simulink model "SecRwLtStCalib"  (R2024b)
settings: Solver=FixedStepDiscrete  StartTime=0.0  StopTime=10.0  FixedStep=0.01  RelTol=1e-3
model workspace (MAT data in the model file):
  KeSMSwAcsMd6SecRwLtStBkReclnUpwdDnwdPos1Max_Val : Simulink.Parameter (value not decoded)
  KeSMSwAcsMd6SecRwLtStBkReclnUpwdDnwdPos1Min_Val : Simulink.Parameter (value not decoded)
  KeSMSwAcsMd6SecRwLtStBkReclnUpwdDnwdPos1_Val : Simulink.Parameter (value not decoded)
  KeSMSwAcsMd6SecRwLtStBkReclnUpwdDnwdPosMax_Val : Simulink.Parameter (value not decoded)
  KeSMSwAcsMd6SecRwLtStBkReclnUpwdDnwdPosMin_Val : Simulink.Parameter (value not decoded)
  KeSMSwAcsMd6SecRwLtStBkReclnUpwdDnwdPos_Val : Simulink.Parameter (value not decoded)
symbols that are objects in the model workspace (value not decoded): KeSMSwAcsMd6SecRwLtStBkReclnUpwdDnwdPos1_Val, KeSMSwAcsMd6SecRwLtStBkReclnUpwdDnwdPos1Max_Val, KeSMSwAcsMd6SecRwLtStBkReclnUpwdDnwdPos1Min_Val, KeSMSwAcsMd6SecRwLtStBkReclnUpwdDnwdPos_Val, KeSMSwAcsMd6SecRwLtStBkReclnUpwdDnwdPosMax_Val, KeSMSwAcsMd6SecRwLtStBkReclnUpwdDnwdPosMin_Val
undefined symbols (not defined in the file or in its folder): KeSMSw4SAcsMd21SecRwLtStBkReclnUpwdDnwdPos_Val, KeSMSw4SAcsMd21SecRwLtStBkReclnUpwdDnwdPosMax_Val, KeSMSw4SAcsMd21SecRwLtStBkReclnUpwdDnwdPosMin_Val, KeSMSw4SAcsMd21SecRwLtStFrwdBkwdPos_Val, KeSMSw4SAcsMd21SecRwLtStFrwdBkwdPosMax_Val, KeSMSw4SAcsMd21SecRwLtStFrwdBkwdPosMin_Val, KeSMSw4SAcsMd21SecRwLtStHdrstFrwdBkwdPos_Val, KeSMSw4SAcsMd21SecRwLtStHdrstFrwdBkwdPosMax_Val, KeSMSw4SAcsMd21SecRwLtStHdrstFrwdBkwdPosMin_Val, KeSMSw4SAcsMd21SecRwLtStHdrstUpwdDnwdPos_Val, KeSMSw4SAcsMd21SecRwLtStHdrstUpwdDnwdPosMax_Val, KeSMSw4SAcsMd21SecRwLtStHdrstUpwdDnwdPosMin_Val, KeSMSw4SAcsMd22SecRwLtStBkReclnUpwdDnwdPos1_Val, KeSMSw4SAcsMd22SecRwLtStBkReclnUpwdDnwdPos2_Val, KeSMSw4SAcsMd22SecRwLtStBkReclnUpwdDnwdPos2Max_Val, KeSMSw4SAcsMd22SecRwLtStBkReclnUpwdDnwdPos2Min_Val, KeSMSw4SAcsMd22SecRwLtStBkReclnUpwdDnwdPosMax_Val, KeSMSw4SAcsMd22SecRwLtStBkReclnUpwdDnwdPosMin_Val, KeSMSw4SAcsMd22SecRwLtStFrwdBkwdPos_Val, KeSMSw4SAcsMd22SecRwLtStFrwdBkwdPosMax_Val, KeSMSw4SAcsMd22SecRwLtStFrwdBkwdPosMin_Val, KeSMSw4SAcsMd22SecRwLtStFtrstUpwdDnwdPos_Val, KeSMSw4SAcsMd22SecRwLtStFtrstUpwdDnwdPosMax_Val, KeSMSw4SAcsMd22SecRwLtStFtrstUpwdDnwdPosMin_Val, KeSMSw4SAcsMd22SecRwLtStHdrstFrwdBkwdPos_Val, KeSMSw4SAcsMd22SecRwLtStHdrstFrwdBkwdPosMax_Val, KeSMSw4SAcsMd22SecRwLtStHdrstFrwdBkwdPosMin_Val, KeSMSw4SAcsMd22SecRwLtStHdrstUpwdDnwdPos_Val, KeSMSw4SAcsMd22SecRwLtStHdrstUpwdDnwdPosMax_Val, KeSMSw4SAcsMd22SecRwLtStHdrstUpwdDnwdPosMin_Val, KeSMSw4SAcsMd22SecRwLtStLegrstOtwdInwdPos_Val, KeSMSw4SAcsMd22SecRwLtStLegrstOtwdInwdPosMax_Val, KeSMSw4SAcsMd22SecRwLtStLegrstOtwdInwdPosMin_Val, KeSMSw4SAcsMd22SecRwLtStLegrstUpwdDnwdPos_Val, KeSMSw4SAcsMd22SecRwLtStLegrstUpwdDnwdPosMax_Val, KeSMSw4SAcsMd22SecRwLtStLegrstUpwdDnwdPosMin_Val, KeSMSw4SAcsMd25SecRwLtStBkReclnUpwdDnwdPos_Val, KeSMSw4SAcsMd25SecRwLtStBkReclnUpwdDnwdPosMax_Val, KeSMSw4SAcsMd25SecRwLtStBkReclnUpwdDnwdPosMin_Val, KeSMSw4SAcsMd25SecRwLtStFrwdBkwdPos_Val, KeSMSw4SAcsMd25SecRwLtStFrwdBkwdPosMax_Val, KeSMSw4SAcsMd25SecRwLtStFrwdBkwdPosMin_Val, KeSMSw4SAcsMd25SecRwLtStHdrstFrwdBkwdPos_Val, KeSMSw4SAcsMd25SecRwLtStHdrstFrwdBkwdPosMax_Val, KeSMSw4SAcsMd25SecRwLtStHdrstFrwdBkwdPosMin_Val, KeSMSw4SAcsMd25SecRwLtStHdrstUpwdDnwdPos_Val, KeSMSw4SAcsMd25SecRwLtStHdrstUpwdDnwdPosMax_Val, KeSMSw4SAcsMd25SecRwLtStHdrstUpwdDnwdPosMin_Val, KeSMSw4SAcsMd26SecRwLtStBkReclnUpwdDnwdPos_Val, KeSMSw4SAcsMd26SecRwLtStBkReclnUpwdDnwdPosMax_Val, KeSMSw4SAcsMd26SecRwLtStBkReclnUpwdDnwdPosMin_Val, KeSMSw4SAcsMd26SecRwLtStFrwdBkwdPos_Val, KeSMSw4SAcsMd26SecRwLtStFrwdBkwdPosMax_Val, KeSMSw4SAcsMd26SecRwLtStFrwdBkwdPosMin_Val, KeSMSw4SAcsMd26SecRwLtStFtrstUpwdDnwdPos_Val, KeSMSw4SAcsMd26SecRwLtStFtrstUpwdDnwdPosMax_Val, KeSMSw4SAcsMd26SecRwLtStFtrstUpwdDnwdPosMin_Val, KeSMSw4SAcsMd26SecRwLtStHdrstFrwdBkwdPos_Val, KeSMSw4SAcsMd26SecRwLtStHdrstFrwdBkwdPosMax_Val, KeSMSw4SAcsMd26SecRwLtStHdrstFrwdBkwdPosMin_Val ... (+496)
libraries: TrgtPosSelcLib x61, StIsPosChkLib x1, simulink x1
(part 4 of 8)

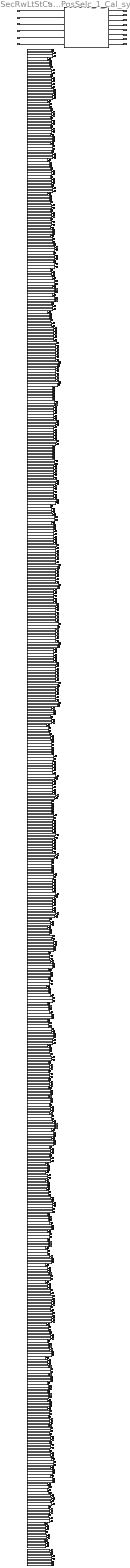
== system SecRwLtStCalib/SecRwLtStZeroTrgtPosSelc_1_Cal_sys ==
  note: Added blocks
  note: Added blocks
  note: Added blocks
  note: Added blocks
  note: Added blocks
  note: Added blocks
  note: Added blocks
  note: Added blocks
  note: Added blocks
  note: Added blocks
  note: Added blocks
  note: Added blocks
  note: Added blocks
  note: Added blocks
  note: Added blocks
  note: Added blocks
  note: Added blocks
  note: Added blocks
  note: Added blocks
  note: Added blocks
  note: Added blocks
  note: Added blocks
  note: Added blocks
  note: Added blocks
  note: Added blocks
  note: Added blocks
  note: Added blocks
  note: Added blocks
  note: Added blocks
  note: Added blocks
  note: Added blocks
  note: Added blocks
  note: Added blocks
  note: Added blocks
  note: Added blocks
  note: Added blocks
  note: Added blocks
  note: Added blocks
  note: Added blocks
  note: Added blocks
  note: Added blocks
  note: Added blocks
  note: Added blocks
  note: Added blocks
  note: Added blocks
  note: Added blocks
  note: Added blocks
  note: Added blocks
  note: Added blocks
  note: Added blocks
  note: Added blocks
  note: Added blocks
  note: Added blocks
  note: Added blocks
  note: Added blocks
  note: Added blocks
  note: Added blocks
  note: Added blocks
  note: Added blocks
  note: Added blocks
  note: Added blocks
  note: Added blocks
  note: Added blocks
  note: Added blocks
  note: Added blocks
  note: Added blocks
  note: Added blocks
  note: Added blocks
  note: Added blocks
  note: Added blocks
  note: Added blocks
  note: Added blocks
  note: Added blocks
  note: Added blocks
  note: Added blocks
  note: Added blocks
  note: Added blocks
  note: Added blocks
  note: Added blocks
  note: Added blocks
  note: Added blocks
  note: Added blocks
  note: Added blocks
  note: Added blocks
  note: Added blocks
  note: Added blocks
  note: Added blocks
  note: Added blocks
  note: Added blocks
  note: Added blocks
  note: Added blocks
  note: Added blocks
  note: Added blocks
  note: Added blocks
  note: Added blocks
  note: Added blocks
  note: Added blocks
  note: Added blocks
  note: Added blocks
  note: Added blocks
  note: Added blocks
  note: Added blocks
  note: Added blocks
  note: Added blocks
  note: Added blocks
  note: Added blocks
  note: Added blocks
  note: Added blocks
  note: Added blocks
  note: Added blocks
  note: Added blocks
  note: Added blocks
  note: Added blocks
  note: Added blocks
  note: Added blocks
  note: Added blocks
  note: Added blocks
  note: Added blocks
  note: Added blocks
  note: Added blocks
  note: Added blocks
  note: Added blocks
  note: Added blocks
  note: Added blocks
  note: Added blocks
  note: Added blocks
  note: Added blocks
  note: Added blocks
  note: Added blocks
  note: Added blocks
  note: Added blocks
  note: Added blocks
  note: Added blocks
  note: Added blocks
  note: Added blocks
  note: Added blocks
  note: Added blocks
  note: Added blocks
  note: Added blocks
  note: Added blocks
  note: Added blocks
  note: Added blocks
  note: Added blocks
  note: Added blocks
  note: Added blocks
  note: Added blocks
  note: Added blocks
  note: Added blocks
  note: Added blocks
  note: Added blocks
  note: Added blocks
  note: Added blocks
  note: Added blocks
  note: Added blocks
  note: Added blocks
  note: Added blocks
  note: Added blocks
  note: Added blocks
  note: Added blocks
  note: Added blocks
  note: Added blocks
  note: Added blocks
  note: Added blocks
  note: Added blocks
  note: Added blocks
  note: Added blocks
  note: Added blocks
  note: Added blocks
  note: Added blocks
  note: Added blocks
  note: Added blocks
  note: Added blocks
  note: Added blocks
  note: Added blocks
  note: Added blocks
  note: Added blocks
  note: Added blocks
  note: Added blocks
  note: Added blocks
  note: Added blocks
  note: Added blocks
  note: Added blocks
  note: Added blocks
  note: Added blocks
  note: Added blocks
  note: Added blocks
  note: Added blocks
  note: Added blocks
  note: Added blocks
  note: Added blocks
  note: Added blocks
  note: Added blocks
  note: Added blocks
  note: Added blocks
  note: Added blocks
  note: Added blocks
  note: Added blocks
  note: Added blocks
  note: Added blocks
  note: Added blocks
  note: Added blocks
  note: Added blocks
  note: Added blocks
  note: Added blocks
  note: Added blocks
  note: Added blocks
  note: Added blocks
  note: Added blocks
  note: Added blocks
  note: Added blocks
  note: Added blocks
  note: Added blocks
  note: Added blocks
  note: Added blocks
  note: Added blocks
  note: Added blocks
  note: Added blocks
  note: Added blocks
  note: Added blocks
  note: Added blocks
  note: Added blocks
  note: Added blocks
  note: Added blocks
  note: Added blocks
  note: Added blocks
  note: Added blocks
  note: Added blocks
  note: Added blocks
  note: Added blocks
  note: Added blocks
  note: Added blocks
  note: Added blocks
  note: Added blocks
  note: Added blocks
  note: Added blocks
  note: Added blocks
  note: Added blocks
  note: Added blocks
  note: Added blocks
  note: Added blocks
  note: Added blocks
  note: Added blocks
  note: Added blocks
  note: Added blocks
  note: Added blocks
  note: Added blocks
  note: Added blocks
  note: Added blocks
  note: Added blocks
  note: Added blocks
  note: Added blocks
  note: Added blocks
  note: Added blocks
  note: Added blocks
  note: Added blocks
  note: Added blocks
  note: Added blocks
  note: Added blocks
  note: Added blocks
  note: Added blocks
  note: Added blocks
  note: Added blocks
  note: Added blocks
  note: Added blocks
  note: Added blocks
  note: Added blocks
  note: Added blocks
  note: Added blocks
  note: Added blocks
  note: Added blocks
  note: Added blocks
  note: Added blocks
  note: Added blocks
  note: Added blocks
  note: Added blocks
  note: Added blocks
  note: Added blocks
  note: Added blocks
  note: Added blocks
  note: Added blocks
  note: Added blocks
  note: Added blocks
  note: Added blocks
  note: Added blocks
  note: Added blocks
  note: Added blocks
  note: Added blocks
  note: Added blocks
  note: Added blocks
  note: Added blocks
  note: Added blocks
  note: Added blocks
  note: Added blocks
  note: Added blocks
  note: Added blocks
  note: Added blocks
  note: Added blocks
  note: Added blocks
  note: Added blocks
  note: Added blocks
  note: Added blocks
  note: Added blocks
  note: Added blocks
  note: Added blocks
  note: Added blocks
  note: Added blocks
  note: Added blocks
  note: Added blocks
  note: Added blocks
  note: Added blocks
  note: Added blocks
  note: Added blocks
  note: Added blocks
  note: Added blocks
  note: Added blocks
  note: Added blocks
  note: Added blocks
  note: Added blocks
  note: Added blocks
  note: Added blocks
  note: Added blocks
  note: Added blocks
  note: Added blocks
  note: Added blocks
  note: Added blocks
  note: Added blocks
  note: Added blocks
  note: Added blocks
  note: Added blocks
  note: Added blocks
  note: Added blocks
  note: Added blocks
  note: Added blocks
  note: Added blocks
  note: Added blocks
  note: Added blocks
  note: Added blocks
  note: Added blocks
  note: Added blocks
  note: Added blocks
  note: Added blocks
  note: Added blocks
  note: Added blocks
  note: Added blocks
  note: Added blocks
  note: Added blocks
  note: Added blocks
  note: Added blocks
  note: Added blocks
  note: Added blocks
  note: Added blocks
  note: Added blocks
  note: Added blocks
  note: Added blocks
  note: Added blocks
  note: Added blocks
  note: Added blocks
  note: Added blocks
  note: Added blocks
  note: Added blocks
  note: Added blocks
  note: Added blocks
  note: Added blocks
  note: Added blocks
  note: Added blocks
  note: Added blocks
  note: Added blocks
  note: Added blocks
  note: Added blocks
  note: Added blocks
  note: Added blocks
  note: Added blocks
  note: Added blocks
  note: Added blocks
  note: Added blocks
  note: Added blocks
  note: Added blocks
  note: Added blocks
  note: Added blocks
  note: Added blocks
  note: Added blocks
  note: Added blocks
  note: Added blocks
  note: Added blocks
  note: Added blocks
  note: Added blocks
  note: Added blocks
  note: Added blocks
  note: Added blocks
  note: Added blocks
  note: Added blocks
  note: Added blocks
  note: Added blocks
  note: Added blocks
  note: Added blocks
  note: Added blocks
  note: Added blocks
  note: Added blocks
  note: Added blocks
  note: Added blocks
  note: Added blocks
  note: Added blocks
  note: Added blocks
  note: Added blocks
  note: Added blocks
  note: Added blocks
  note: Added blocks
  note: Added blocks
  note: Added blocks
  note: Added blocks
  note: Added blocks
  note: Added blocks
  note: Added blocks
  note: Added blocks
  note: Added blocks
  note: Added blocks
  note: Added blocks
  note: Added blocks
  note: Added blocks
  note: Added blocks
  note: Added blocks
  note: Added blocks
  note: Added blocks
  note: Added blocks
  note: Added blocks
  note: Added blocks
  note: Added blocks
  note: Added blocks
  note: Added blocks
  note: Added blocks
  note: Added blocks
  note: Added blocks
  note: Added blocks
  note: Added blocks
  note: Added blocks
  note: Added blocks
  note: Added blocks
  note: Added blocks
  note: Added blocks
  note: Added blocks
  note: Added blocks
  note: Added blocks
  note: Added blocks
  note: Added blocks
  note: Added blocks
  note: Added blocks
  note: Added blocks
  note: Added blocks
  note: Added blocks
  note: Added blocks
  note: Added blocks
  note: Added blocks
  note: Added blocks
  note: Added blocks
  note: Added blocks
  note: Added blocks
  note: Added blocks
  note: Added blocks
  note: Added blocks
  note: Added blocks
  note: Added blocks
  note: Added blocks
  note: Added blocks
  note: Added blocks
  note: Added blocks
  note: Added blocks
  note: Added blocks
  note: Added blocks
  note: Added blocks
  note: Added blocks
  note: Added blocks
  note: Added blocks
  note: Added blocks
  note: Added blocks
  note: Added blocks
  note: Added blocks
  note: Added blocks
  note: Added blocks
  note: Added blocks
  note: Added blocks
  note: Added blocks
  note: Added blocks
  note: Added blocks
  note: Added blocks
  note: Added blocks
  note: Added blocks
  note: Added blocks
  note: Added blocks
  note: Added blocks
  note: Added blocks
  note: Added blocks
  note: Added blocks
  note: Added blocks
  note: Added blocks
  note: Added blocks
  note: Added blocks
  note: Added blocks
  note: Added blocks
  note: Added blocks
  note: Added blocks
  note: Added blocks
  note: Added blocks
  note: Added blocks
  note: Added blocks
  note: Added blocks
  note: Added blocks
  note: Added blocks
  note: Added blocks
  note: Added blocks
  note: Added blocks
  note: Added blocks
  note: Added blocks
  note: Added blocks
  note: Added blocks
  note: Added blocks
  note: Added blocks
  note: Added blocks
  note: Added blocks
  note: Added blocks
  note: Added blocks
  note: Added blocks
  note: Added blocks
  note: Added blocks
  note: Added blocks
  note: Added blocks
  note: Added blocks
  note: Added blocks
  note: Added blocks
  note: Added blocks
  note: Added blocks
  note: Added blocks
  note: Added blocks
  note: Added blocks
  note: Added blocks
  note: Added blocks
  note: Added blocks
  note: Added blocks
  note: Added blocks
  note: Added blocks
  StNumFlg_Is4s_read : Inport
  StNumFlg_Is6s_read : Inport  Port=2
  StNumFlg_Is6s7s_read : Inport  Port=3
  StNumFlg_Is7s_read : Inport  Port=4
  Md61SecRwRtStCushFrntTrgtPosCalib_TrgtPosArray_read : Inport  Port=5
  Md62SecRwLtStCushFrntTrgtPosCalib_TrgtPosArray_read : Inport  Port=6
  function : TriggerPort  TriggerType=function-call  IsSimulinkFunction=on  FunctionName=SecRwLtStZeroTrgtPosSelc_1_Cal  VariantControl=(inherit)
  PA_KeSMSw4SAcsMd21SecRwLtStBkReclnUpwdDnwdPosMax_Val : Constant  Value=KeSMSw4SAcsMd21SecRwLtStBkReclnUpwdDnwdPosMax_Val
  PA_KeSMSw4SAcsMd21SecRwLtStBkReclnUpwdDnwdPosMin_Val : Constant  Value=KeSMSw4SAcsMd21SecRwLtStBkReclnUpwdDnwdPosMin_Val
  PA_KeSMSw4SAcsMd21SecRwLtStBkReclnUpwdDnwdPos_Val : Constant  Value=KeSMSw4SAcsMd21SecRwLtStBkReclnUpwdDnwdPos_Val
  PA_KeSMSw4SAcsMd21SecRwLtStFrwdBkwdPosMax_Val : Constant  Value=KeSMSw4SAcsMd21SecRwLtStFrwdBkwdPosMax_Val
  PA_KeSMSw4SAcsMd21SecRwLtStFrwdBkwdPosMin_Val : Constant  Value=KeSMSw4SAcsMd21SecRwLtStFrwdBkwdPosMin_Val
  PA_KeSMSw4SAcsMd21SecRwLtStFrwdBkwdPos_Val : Constant  Value=KeSMSw4SAcsMd21SecRwLtStFrwdBkwdPos_Val
  PA_KeSMSw4SAcsMd21SecRwLtStHdrstFrwdBkwdPosMax_Val : Constant  Value=KeSMSw4SAcsMd21SecRwLtStHdrstFrwdBkwdPosMax_Val
  PA_KeSMSw4SAcsMd21SecRwLtStHdrstFrwdBkwdPosMin_Val : Constant  Value=KeSMSw4SAcsMd21SecRwLtStHdrstFrwdBkwdPosMin_Val
  PA_KeSMSw4SAcsMd21SecRwLtStHdrstFrwdBkwdPos_Val : Constant  Value=KeSMSw4SAcsMd21SecRwLtStHdrstFrwdBkwdPos_Val
  PA_KeSMSw4SAcsMd21SecRwLtStHdrstUpwdDnwdPosMax_Val : Constant  Value=KeSMSw4SAcsMd21SecRwLtStHdrstUpwdDnwdPosMax_Val
  PA_KeSMSw4SAcsMd21SecRwLtStHdrstUpwdDnwdPosMin_Val : Constant  Value=KeSMSw4SAcsMd21SecRwLtStHdrstUpwdDnwdPosMin_Val
  PA_KeSMSw4SAcsMd21SecRwLtStHdrstUpwdDnwdPos_Val : Constant  Value=KeSMSw4SAcsMd21SecRwLtStHdrstUpwdDnwdPos_Val
  PA_KeSMSw4SAcsMd22SecRwLtStBkReclnUpwdDnwdPos1_Val : Constant  Value=KeSMSw4SAcsMd22SecRwLtStBkReclnUpwdDnwdPos1_Val
  PA_KeSMSw4SAcsMd22SecRwLtStBkReclnUpwdDnwdPos2Max_Val : Constant  Value=KeSMSw4SAcsMd22SecRwLtStBkReclnUpwdDnwdPos2Max_Val
  PA_KeSMSw4SAcsMd22SecRwLtStBkReclnUpwdDnwdPos2Min_Val : Constant  Value=KeSMSw4SAcsMd22SecRwLtStBkReclnUpwdDnwdPos2Min_Val
  PA_KeSMSw4SAcsMd22SecRwLtStBkReclnUpwdDnwdPos2_Val : Constant  Value=KeSMSw4SAcsMd22SecRwLtStBkReclnUpwdDnwdPos2_Val
  PA_KeSMSw4SAcsMd22SecRwLtStBkReclnUpwdDnwdPosMax_Val : Constant  Value=KeSMSw4SAcsMd22SecRwLtStBkReclnUpwdDnwdPosMax_Val
  PA_KeSMSw4SAcsMd22SecRwLtStBkReclnUpwdDnwdPosMin_Val : Constant  Value=KeSMSw4SAcsMd22SecRwLtStBkReclnUpwdDnwdPosMin_Val
  PA_KeSMSw4SAcsMd22SecRwLtStFrwdBkwdPosMax_Val : Constant  Value=KeSMSw4SAcsMd22SecRwLtStFrwdBkwdPosMax_Val
  PA_KeSMSw4SAcsMd22SecRwLtStFrwdBkwdPosMin_Val : Constant  Value=KeSMSw4SAcsMd22SecRwLtStFrwdBkwdPosMin_Val
  PA_KeSMSw4SAcsMd22SecRwLtStFrwdBkwdPos_Val : Constant  Value=KeSMSw4SAcsMd22SecRwLtStFrwdBkwdPos_Val
  PA_KeSMSw4SAcsMd22SecRwLtStFtrstUpwdDnwdPosMax_Val : Constant  Value=KeSMSw4SAcsMd22SecRwLtStFtrstUpwdDnwdPosMax_Val
  PA_KeSMSw4SAcsMd22SecRwLtStFtrstUpwdDnwdPosMin_Val : Constant  Value=KeSMSw4SAcsMd22SecRwLtStFtrstUpwdDnwdPosMin_Val
  PA_KeSMSw4SAcsMd22SecRwLtStFtrstUpwdDnwdPos_Val : Constant  Value=KeSMSw4SAcsMd22SecRwLtStFtrstUpwdDnwdPos_Val
  PA_KeSMSw4SAcsMd22SecRwLtStHdrstFrwdBkwdPosMax_Val : Constant  Value=KeSMSw4SAcsMd22SecRwLtStHdrstFrwdBkwdPosMax_Val
  PA_KeSMSw4SAcsMd22SecRwLtStHdrstFrwdBkwdPosMin_Val : Constant  Value=KeSMSw4SAcsMd22SecRwLtStHdrstFrwdBkwdPosMin_Val
  PA_KeSMSw4SAcsMd22SecRwLtStHdrstFrwdBkwdPos_Val : Constant  Value=KeSMSw4SAcsMd22SecRwLtStHdrstFrwdBkwdPos_Val
  PA_KeSMSw4SAcsMd22SecRwLtStHdrstUpwdDnwdPosMax_Val : Constant  Value=KeSMSw4SAcsMd22SecRwLtStHdrstUpwdDnwdPosMax_Val
  PA_KeSMSw4SAcsMd22SecRwLtStHdrstUpwdDnwdPosMin_Val : Constant  Value=KeSMSw4SAcsMd22SecRwLtStHdrstUpwdDnwdPosMin_Val
  PA_KeSMSw4SAcsMd22SecRwLtStHdrstUpwdDnwdPos_Val : Constant  Value=KeSMSw4SAcsMd22SecRwLtStHdrstUpwdDnwdPos_Val
  PA_KeSMSw4SAcsMd22SecRwLtStLegrstOtwdInwdPosMax_Val : Constant  Value=KeSMSw4SAcsMd22SecRwLtStLegrstOtwdInwdPosMax_Val
  PA_KeSMSw4SAcsMd22SecRwLtStLegrstOtwdInwdPosMin_Val : Constant  Value=KeSMSw4SAcsMd22SecRwLtStLegrstOtwdInwdPosMin_Val
  PA_KeSMSw4SAcsMd22SecRwLtStLegrstOtwdInwdPos_Val : Constant  Value=KeSMSw4SAcsMd22SecRwLtStLegrstOtwdInwdPos_Val
  PA_KeSMSw4SAcsMd22SecRwLtStLegrstUpwdDnwdPosMax_Val : Constant  Value=KeSMSw4SAcsMd22SecRwLtStLegrstUpwdDnwdPosMax_Val
  PA_KeSMSw4SAcsMd22SecRwLtStLegrstUpwdDnwdPosMin_Val : Constant  Value=KeSMSw4SAcsMd22SecRwLtStLegrstUpwdDnwdPosMin_Val
  PA_KeSMSw4SAcsMd22SecRwLtStLegrstUpwdDnwdPos_Val : Constant  Value=KeSMSw4SAcsMd22SecRwLtStLegrstUpwdDnwdPos_Val
  PA_KeSMSw4SAcsMd25SecRwLtStBkReclnUpwdDnwdPosMax_Val : Constant  Value=KeSMSw4SAcsMd25SecRwLtStBkReclnUpwdDnwdPosMax_Val
  PA_KeSMSw4SAcsMd25SecRwLtStBkReclnUpwdDnwdPosMin_Val : Constant  Value=KeSMSw4SAcsMd25SecRwLtStBkReclnUpwdDnwdPosMin_Val
  PA_KeSMSw4SAcsMd25SecRwLtStBkReclnUpwdDnwdPos_Val : Constant  Value=KeSMSw4SAcsMd25SecRwLtStBkReclnUpwdDnwdPos_Val
  PA_KeSMSw4SAcsMd25SecRwLtStFrwdBkwdPosMax_Val : Constant  Value=KeSMSw4SAcsMd25SecRwLtStFrwdBkwdPosMax_Val
  PA_KeSMSw4SAcsMd25SecRwLtStFrwdBkwdPosMin_Val : Constant  Value=KeSMSw4SAcsMd25SecRwLtStFrwdBkwdPosMin_Val
  PA_KeSMSw4SAcsMd25SecRwLtStFrwdBkwdPos_Val : Constant  Value=KeSMSw4SAcsMd25SecRwLtStFrwdBkwdPos_Val
  PA_KeSMSw4SAcsMd25SecRwLtStHdrstFrwdBkwdPosMax_Val : Constant  Value=KeSMSw4SAcsMd25SecRwLtStHdrstFrwdBkwdPosMax_Val
  PA_KeSMSw4SAcsMd25SecRwLtStHdrstFrwdBkwdPosMin_Val : Constant  Value=KeSMSw4SAcsMd25SecRwLtStHdrstFrwdBkwdPosMin_Val
  PA_KeSMSw4SAcsMd25SecRwLtStHdrstFrwdBkwdPos_Val : Constant  Value=KeSMSw4SAcsMd25SecRwLtStHdrstFrwdBkwdPos_Val
  PA_KeSMSw4SAcsMd25SecRwLtStHdrstUpwdDnwdPosMax_Val : Constant  Value=KeSMSw4SAcsMd25SecRwLtStHdrstUpwdDnwdPosMax_Val
  PA_KeSMSw4SAcsMd25SecRwLtStHdrstUpwdDnwdPosMin_Val : Constant  Value=KeSMSw4SAcsMd25SecRwLtStHdrstUpwdDnwdPosMin_Val
  PA_KeSMSw4SAcsMd25SecRwLtStHdrstUpwdDnwdPos_Val : Constant  Value=KeSMSw4SAcsMd25SecRwLtStHdrstUpwdDnwdPos_Val
  PA_KeSMSw4SAcsMd26SecRwLtStBkReclnUpwdDnwdPosMax_Val : Constant  Value=KeSMSw4SAcsMd26SecRwLtStBkReclnUpwdDnwdPosMax_Val
  PA_KeSMSw4SAcsMd26SecRwLtStBkReclnUpwdDnwdPosMin_Val : Constant  Value=KeSMSw4SAcsMd26SecRwLtStBkReclnUpwdDnwdPosMin_Val
  PA_KeSMSw4SAcsMd26SecRwLtStBkReclnUpwdDnwdPos_Val : Constant  Value=KeSMSw4SAcsMd26SecRwLtStBkReclnUpwdDnwdPos_Val
  PA_KeSMSw4SAcsMd26SecRwLtStFrwdBkwdPosMax_Val : Constant  Value=KeSMSw4SAcsMd26SecRwLtStFrwdBkwdPosMax_Val
  PA_KeSMSw4SAcsMd26SecRwLtStFrwdBkwdPosMin_Val : Constant  Value=KeSMSw4SAcsMd26SecRwLtStFrwdBkwdPosMin_Val
  PA_KeSMSw4SAcsMd26SecRwLtStFrwdBkwdPos_Val : Constant  Value=KeSMSw4SAcsMd26SecRwLtStFrwdBkwdPos_Val
  PA_KeSMSw4SAcsMd26SecRwLtStFtrstUpwdDnwdPosMax_Val : Constant  Value=KeSMSw4SAcsMd26SecRwLtStFtrstUpwdDnwdPosMax_Val
  PA_KeSMSw4SAcsMd26SecRwLtStFtrstUpwdDnwdPosMin_Val : Constant  Value=KeSMSw4SAcsMd26SecRwLtStFtrstUpwdDnwdPosMin_Val
  PA_KeSMSw4SAcsMd26SecRwLtStFtrstUpwdDnwdPos_Val : Constant  Value=KeSMSw4SAcsMd26SecRwLtStFtrstUpwdDnwdPos_Val
  PA_KeSMSw4SAcsMd26SecRwLtStHdrstFrwdBkwdPosMax_Val : Constant  Value=KeSMSw4SAcsMd26SecRwLtStHdrstFrwdBkwdPosMax_Val
  PA_KeSMSw4SAcsMd26SecRwLtStHdrstFrwdBkwdPosMin_Val : Constant  Value=KeSMSw4SAcsMd26SecRwLtStHdrstFrwdBkwdPosMin_Val
  PA_KeSMSw4SAcsMd26SecRwLtStHdrstFrwdBkwdPos_Val : Constant  Value=KeSMSw4SAcsMd26SecRwLtStHdrstFrwdBkwdPos_Val
  PA_KeSMSw4SAcsMd26SecRwLtStHdrstUpwdDnwdPosMax_Val : Constant  Value=KeSMSw4SAcsMd26SecRwLtStHdrstUpwdDnwdPosMax_Val
  PA_KeSMSw4SAcsMd26SecRwLtStHdrstUpwdDnwdPosMin_Val : Constant  Value=KeSMSw4SAcsMd26SecRwLtStHdrstUpwdDnwdPosMin_Val
  PA_KeSMSw4SAcsMd26SecRwLtStHdrstUpwdDnwdPos_Val : Constant  Value=KeSMSw4SAcsMd26SecRwLtStHdrstUpwdDnwdPos_Val
  PA_KeSMSw4SAcsMd26SecRwLtStLegrstOtwdInwdPosMax_Val : Constant  Value=KeSMSw4SAcsMd26SecRwLtStLegrstOtwdInwdPosMax_Val
  PA_KeSMSw4SAcsMd26SecRwLtStLegrstOtwdInwdPosMin_Val : Constant  Value=KeSMSw4SAcsMd26SecRwLtStLegrstOtwdInwdPosMin_Val
  PA_KeSMSw4SAcsMd26SecRwLtStLegrstOtwdInwdPos_Val : Constant  Value=KeSMSw4SAcsMd26SecRwLtStLegrstOtwdInwdPos_Val
  PA_KeSMSw4SAcsMd26SecRwLtStLegrstUpwdDnwdPosMax_Val : Constant  Value=KeSMSw4SAcsMd26SecRwLtStLegrstUpwdDnwdPosMax_Val
  PA_KeSMSw4SAcsMd26SecRwLtStLegrstUpwdDnwdPosMin_Val : Constant  Value=KeSMSw4SAcsMd26SecRwLtStLegrstUpwdDnwdPosMin_Val
  PA_KeSMSw4SAcsMd26SecRwLtStLegrstUpwdDnwdPos_Val : Constant  Value=KeSMSw4SAcsMd26SecRwLtStLegrstUpwdDnwdPos_Val
  PA_KeSMSw4SLegrstCloseMdSecRwLtStFtrstUpwdDnwdPosMax_Val : Constant  Value=KeSMSw4SLegrstCloseMdSecRwLtStFtrstUpwdDnwdPosMax_Val
  PA_KeSMSw4SLegrstCloseMdSecRwLtStFtrstUpwdDnwdPosMin_Val : Constant  Value=KeSMSw4SLegrstCloseMdSecRwLtStFtrstUpwdDnwdPosMin_Val
  PA_KeSMSw4SLegrstCloseMdSecRwLtStFtrstUpwdDnwdPos_Val : Constant  Value=KeSMSw4SLegrstCloseMdSecRwLtStFtrstUpwdDnwdPos_Val
  PA_KeSMSw4SLegrstCloseMdSecRwLtStLgrstOtwdInwdPosMax_Val : Constant  Value=KeSMSw4SLegrstCloseMdSecRwLtStLgrstOtwdInwdPosMax_Val
  PA_KeSMSw4SLegrstCloseMdSecRwLtStLgrstOtwdInwdPosMin_Val : Constant  Value=KeSMSw4SLegrstCloseMdSecRwLtStLgrstOtwdInwdPosMin_Val
  PA_KeSMSw4SLegrstCloseMdSecRwLtStLgrstOtwdInwdPos_Val : Constant  Value=KeSMSw4SLegrstCloseMdSecRwLtStLgrstOtwdInwdPos_Val
  PA_KeSMSw4SLegrstCloseMdSecRwLtStLgrstUpwdDnwdPosMax_Val : Constant  Value=KeSMSw4SLegrstCloseMdSecRwLtStLgrstUpwdDnwdPosMax_Val
  PA_KeSMSw4SLegrstCloseMdSecRwLtStLgrstUpwdDnwdPosMin_Val : Constant  Value=KeSMSw4SLegrstCloseMdSecRwLtStLgrstUpwdDnwdPosMin_Val
  PA_KeSMSw4SLegrstCloseMdSecRwLtStLgrstUpwdDnwdPos_Val : Constant  Value=KeSMSw4SLegrstCloseMdSecRwLtStLgrstUpwdDnwdPos_Val
  PA_KeSMSw4SLegrstOpenMdSecRwLtStFrwdBkwdPosMax_Val : Constant  Value=KeSMSw4SLegrstOpenMdSecRwLtStFrwdBkwdPosMax_Val
  PA_KeSMSw4SLegrstOpenMdSecRwLtStFrwdBkwdPosMin_Val : Constant  Value=KeSMSw4SLegrstOpenMdSecRwLtStFrwdBkwdPosMin_Val
  PA_KeSMSw4SLegrstOpenMdSecRwLtStFrwdBkwdPos_Val : Constant  Value=KeSMSw4SLegrstOpenMdSecRwLtStFrwdBkwdPos_Val
  PA_KeSMSw4SLegrstOpenMdSecRwLtStFtrstUpwdDnwdPosMax_Val : Constant  Value=KeSMSw4SLegrstOpenMdSecRwLtStFtrstUpwdDnwdPosMax_Val
  PA_KeSMSw4SLegrstOpenMdSecRwLtStFtrstUpwdDnwdPosMin_Val : Constant  Value=KeSMSw4SLegrstOpenMdSecRwLtStFtrstUpwdDnwdPosMin_Val
  PA_KeSMSw4SLegrstOpenMdSecRwLtStFtrstUpwdDnwdPos_Val : Constant  Value=KeSMSw4SLegrstOpenMdSecRwLtStFtrstUpwdDnwdPos_Val
  PA_KeSMSw4SLegrstOpenMdSecRwLtStLgrstOtwdInwdPosMax_Val : Constant  Value=KeSMSw4SLegrstOpenMdSecRwLtStLgrstOtwdInwdPosMax_Val
  PA_KeSMSw4SLegrstOpenMdSecRwLtStLgrstOtwdInwdPosMin_Val : Constant  Value=KeSMSw4SLegrstOpenMdSecRwLtStLgrstOtwdInwdPosMin_Val
  PA_KeSMSw4SLegrstOpenMdSecRwLtStLgrstOtwdInwdPos_Val : Constant  Value=KeSMSw4SLegrstOpenMdSecRwLtStLgrstOtwdInwdPos_Val
  PA_KeSMSw4SLegrstOpenMdSecRwLtStLgrstUpwdDnwdPosMax_Val : Constant  Value=KeSMSw4SLegrstOpenMdSecRwLtStLgrstUpwdDnwdPosMax_Val
  PA_KeSMSw4SLegrstOpenMdSecRwLtStLgrstUpwdDnwdPosMin_Val : Constant  Value=KeSMSw4SLegrstOpenMdSecRwLtStLgrstUpwdDnwdPosMin_Val
  PA_KeSMSw4SLegrstOpenMdSecRwLtStLgrstUpwdDnwdPos_Val : Constant  Value=KeSMSw4SLegrstOpenMdSecRwLtStLgrstUpwdDnwdPos_Val
  PA_KeSMSw4SLyingMDSecRwLtStFrwdBkwdPosMax_Val : Constant  Value=KeSMSw4SLyingMDSecRwLtStFrwdBkwdPosMax_Val
  PA_KeSMSw4SLyingMDSecRwLtStFrwdBkwdPosMin_Val : Constant  Value=KeSMSw4SLyingMDSecRwLtStFrwdBkwdPosMin_Val
  PA_KeSMSw4SLyingMDSecRwLtStFrwdBkwdPos_Val : Constant  Value=KeSMSw4SLyingMDSecRwLtStFrwdBkwdPos_Val
  PA_KeSMSw4SVIPMDSecRwLtStFrwdBkwdPosMax_Val : Constant  Value=KeSMSw4SVIPMDSecRwLtStFrwdBkwdPosMax_Val
  PA_KeSMSw4SVIPMDSecRwLtStFrwdBkwdPosMin_Val : Constant  Value=KeSMSw4SVIPMDSecRwLtStFrwdBkwdPosMin_Val
  PA_KeSMSw4SVIPMDSecRwLtStFrwdBkwdPos_Val : Constant  Value=KeSMSw4SVIPMDSecRwLtStFrwdBkwdPos_Val
  PA_KeSMSw4sLyingMDSecRwLtStBkReclnUpwdDnwdPosMax_Val : Constant  Value=KeSMSw4sLyingMDSecRwLtStBkReclnUpwdDnwdPosMax_Val
  PA_KeSMSw4sLyingMDSecRwLtStBkReclnUpwdDnwdPosMin_Val : Constant  Value=KeSMSw4sLyingMDSecRwLtStBkReclnUpwdDnwdPosMin_Val
  PA_KeSMSw4sLyingMDSecRwLtStBkReclnUpwdDnwdPos_Val : Constant  Value=KeSMSw4sLyingMDSecRwLtStBkReclnUpwdDnwdPos_Val
  PA_KeSMSw4sLyingMDSecRwLtStFtrstUpwdDnwdPosMax_Val : Constant  Value=KeSMSw4sLyingMDSecRwLtStFtrstUpwdDnwdPosMax_Val
  PA_KeSMSw4sLyingMDSecRwLtStFtrstUpwdDnwdPosMin_Val : Constant  Value=KeSMSw4sLyingMDSecRwLtStFtrstUpwdDnwdPosMin_Val
  PA_KeSMSw4sLyingMDSecRwLtStFtrstUpwdDnwdPos_Val : Constant  Value=KeSMSw4sLyingMDSecRwLtStFtrstUpwdDnwdPos_Val
  PA_KeSMSw4sLyingMDSecRwLtStHdrstFrwdBkwdnwdPosMax_160_Val : Constant  Value=KeSMSw4sLyingMDSecRwLtStHdrstFrwdBkwdnwdPosMax_160_Val
  PA_KeSMSw4sLyingMDSecRwLtStHdrstFrwdBkwdnwdPosMax_165_Val : Constant  Value=KeSMSw4sLyingMDSecRwLtStHdrstFrwdBkwdnwdPosMax_165_Val
  PA_KeSMSw4sLyingMDSecRwLtStHdrstFrwdBkwdnwdPosMax_170_Val : Constant  Value=KeSMSw4sLyingMDSecRwLtStHdrstFrwdBkwdnwdPosMax_170_Val
  PA_KeSMSw4sLyingMDSecRwLtStHdrstFrwdBkwdnwdPosMax_175_Val : Constant  Value=KeSMSw4sLyingMDSecRwLtStHdrstFrwdBkwdnwdPosMax_175_Val
  PA_KeSMSw4sLyingMDSecRwLtStHdrstFrwdBkwdnwdPosMax_180_Val : Constant  Value=KeSMSw4sLyingMDSecRwLtStHdrstFrwdBkwdnwdPosMax_180_Val
  PA_KeSMSw4sLyingMDSecRwLtStHdrstFrwdBkwdnwdPosMax_Below160_Val : Constant  Value=KeSMSw4sLyingMDSecRwLtStHdrstFrwdBkwdnwdPosMax_Below160_Val
  PA_KeSMSw4sLyingMDSecRwLtStHdrstFrwdBkwdnwdPosMax_Over180_Val : Constant  Value=KeSMSw4sLyingMDSecRwLtStHdrstFrwdBkwdnwdPosMax_Over180_Val
  PA_KeSMSw4sLyingMDSecRwLtStHdrstFrwdBkwdnwdPosMin_160_Val : Constant  Value=KeSMSw4sLyingMDSecRwLtStHdrstFrwdBkwdnwdPosMin_160_Val
  PA_KeSMSw4sLyingMDSecRwLtStHdrstFrwdBkwdnwdPosMin_165_Val : Constant  Value=KeSMSw4sLyingMDSecRwLtStHdrstFrwdBkwdnwdPosMin_165_Val
  PA_KeSMSw4sLyingMDSecRwLtStHdrstFrwdBkwdnwdPosMin_170_Val : Constant  Value=KeSMSw4sLyingMDSecRwLtStHdrstFrwdBkwdnwdPosMin_170_Val
  PA_KeSMSw4sLyingMDSecRwLtStHdrstFrwdBkwdnwdPosMin_175_Val : Constant  Value=KeSMSw4sLyingMDSecRwLtStHdrstFrwdBkwdnwdPosMin_175_Val
  PA_KeSMSw4sLyingMDSecRwLtStHdrstFrwdBkwdnwdPosMin_180_Val : Constant  Value=KeSMSw4sLyingMDSecRwLtStHdrstFrwdBkwdnwdPosMin_180_Val
  PA_KeSMSw4sLyingMDSecRwLtStHdrstFrwdBkwdnwdPosMin_Below160_Val : Constant  Value=KeSMSw4sLyingMDSecRwLtStHdrstFrwdBkwdnwdPosMin_Below160_Val
  PA_KeSMSw4sLyingMDSecRwLtStHdrstFrwdBkwdnwdPosMin_Over180_Val : Constant  Value=KeSMSw4sLyingMDSecRwLtStHdrstFrwdBkwdnwdPosMin_Over180_Val
  PA_KeSMSw4sLyingMDSecRwLtStHdrstFrwdBkwdnwdPos_160_Val : Constant  Value=KeSMSw4sLyingMDSecRwLtStHdrstFrwdBkwdnwdPos_160_Val
  PA_KeSMSw4sLyingMDSecRwLtStHdrstFrwdBkwdnwdPos_165_Val : Constant  Value=KeSMSw4sLyingMDSecRwLtStHdrstFrwdBkwdnwdPos_165_Val
  PA_KeSMSw4sLyingMDSecRwLtStHdrstFrwdBkwdnwdPos_170_Val : Constant  Value=KeSMSw4sLyingMDSecRwLtStHdrstFrwdBkwdnwdPos_170_Val
  PA_KeSMSw4sLyingMDSecRwLtStHdrstFrwdBkwdnwdPos_175_Val : Constant  Value=KeSMSw4sLyingMDSecRwLtStHdrstFrwdBkwdnwdPos_175_Val
  PA_KeSMSw4sLyingMDSecRwLtStHdrstFrwdBkwdnwdPos_180_Val : Constant  Value=KeSMSw4sLyingMDSecRwLtStHdrstFrwdBkwdnwdPos_180_Val
  PA_KeSMSw4sLyingMDSecRwLtStHdrstFrwdBkwdnwdPos_Below160_Val : Constant  Value=KeSMSw4sLyingMDSecRwLtStHdrstFrwdBkwdnwdPos_Below160_Val
  PA_KeSMSw4sLyingMDSecRwLtStHdrstFrwdBkwdnwdPos_Over180_Val : Constant  Value=KeSMSw4sLyingMDSecRwLtStHdrstFrwdBkwdnwdPos_Over180_Val
  PA_KeSMSw4sLyingMDSecRwLtStHdrstUpwdDnwdPosMax_160_Val : Constant  Value=KeSMSw4sLyingMDSecRwLtStHdrstUpwdDnwdPosMax_160_Val
  PA_KeSMSw4sLyingMDSecRwLtStHdrstUpwdDnwdPosMax_165_Val : Constant  Value=KeSMSw4sLyingMDSecRwLtStHdrstUpwdDnwdPosMax_165_Val
  PA_KeSMSw4sLyingMDSecRwLtStHdrstUpwdDnwdPosMax_170_Val : Constant  Value=KeSMSw4sLyingMDSecRwLtStHdrstUpwdDnwdPosMax_170_Val
  PA_KeSMSw4sLyingMDSecRwLtStHdrstUpwdDnwdPosMax_175_Val : Constant  Value=KeSMSw4sLyingMDSecRwLtStHdrstUpwdDnwdPosMax_175_Val
  PA_KeSMSw4sLyingMDSecRwLtStHdrstUpwdDnwdPosMax_180_Val : Constant  Value=KeSMSw4sLyingMDSecRwLtStHdrstUpwdDnwdPosMax_180_Val
  PA_KeSMSw4sLyingMDSecRwLtStHdrstUpwdDnwdPosMax_Below160_Val : Constant  Value=KeSMSw4sLyingMDSecRwLtStHdrstUpwdDnwdPosMax_Below160_Val
  PA_KeSMSw4sLyingMDSecRwLtStHdrstUpwdDnwdPosMax_Over180_Val : Constant  Value=KeSMSw4sLyingMDSecRwLtStHdrstUpwdDnwdPosMax_Over180_Val
  PA_KeSMSw4sLyingMDSecRwLtStHdrstUpwdDnwdPosMin_160_Val : Constant  Value=KeSMSw4sLyingMDSecRwLtStHdrstUpwdDnwdPosMin_160_Val
  PA_KeSMSw4sLyingMDSecRwLtStHdrstUpwdDnwdPosMin_165_Val : Constant  Value=KeSMSw4sLyingMDSecRwLtStHdrstUpwdDnwdPosMin_165_Val
  PA_KeSMSw4sLyingMDSecRwLtStHdrstUpwdDnwdPosMin_170_Val : Constant  Value=KeSMSw4sLyingMDSecRwLtStHdrstUpwdDnwdPosMin_170_Val
  PA_KeSMSw4sLyingMDSecRwLtStHdrstUpwdDnwdPosMin_175_Val : Constant  Value=KeSMSw4sLyingMDSecRwLtStHdrstUpwdDnwdPosMin_175_Val
  PA_KeSMSw4sLyingMDSecRwLtStHdrstUpwdDnwdPosMin_180_Val : Constant  Value=KeSMSw4sLyingMDSecRwLtStHdrstUpwdDnwdPosMin_180_Val
  PA_KeSMSw4sLyingMDSecRwLtStHdrstUpwdDnwdPosMin_Below160_Val : Constant  Value=KeSMSw4sLyingMDSecRwLtStHdrstUpwdDnwdPosMin_Below160_Val
  PA_KeSMSw4sLyingMDSecRwLtStHdrstUpwdDnwdPosMin_Over180_Val : Constant  Value=KeSMSw4sLyingMDSecRwLtStHdrstUpwdDnwdPosMin_Over180_Val
  PA_KeSMSw4sLyingMDSecRwLtStHdrstUpwdDnwdPos_160_Val : Constant  Value=KeSMSw4sLyingMDSecRwLtStHdrstUpwdDnwdPos_160_Val
  PA_KeSMSw4sLyingMDSecRwLtStHdrstUpwdDnwdPos_165_Val : Constant  Value=KeSMSw4sLyingMDSecRwLtStHdrstUpwdDnwdPos_165_Val
  PA_KeSMSw4sLyingMDSecRwLtStHdrstUpwdDnwdPos_170_Val : Constant  Value=KeSMSw4sLyingMDSecRwLtStHdrstUpwdDnwdPos_170_Val
  PA_KeSMSw4sLyingMDSecRwLtStHdrstUpwdDnwdPos_175_Val : Constant  Value=KeSMSw4sLyingMDSecRwLtStHdrstUpwdDnwdPos_175_Val
  PA_KeSMSw4sLyingMDSecRwLtStHdrstUpwdDnwdPos_180_Val : Constant  Value=KeSMSw4sLyingMDSecRwLtStHdrstUpwdDnwdPos_180_Val
  PA_KeSMSw4sLyingMDSecRwLtStHdrstUpwdDnwdPos_Below160_Val : Constant  Value=KeSMSw4sLyingMDSecRwLtStHdrstUpwdDnwdPos_Below160_Val
  PA_KeSMSw4sLyingMDSecRwLtStHdrstUpwdDnwdPos_Over180_Val : Constant  Value=KeSMSw4sLyingMDSecRwLtStHdrstUpwdDnwdPos_Over180_Val
  PA_KeSMSw4sLyingMDSecRwLtStLgrstOtwdInwdPosMax_160_Val : Constant  Value=KeSMSw4sLyingMDSecRwLtStLgrstOtwdInwdPosMax_160_Val
  PA_KeSMSw4sLyingMDSecRwLtStLgrstOtwdInwdPosMax_165_Val : Constant  Value=KeSMSw4sLyingMDSecRwLtStLgrstOtwdInwdPosMax_165_Val
  PA_KeSMSw4sLyingMDSecRwLtStLgrstOtwdInwdPosMax_170_Val : Constant  Value=KeSMSw4sLyingMDSecRwLtStLgrstOtwdInwdPosMax_170_Val
  PA_KeSMSw4sLyingMDSecRwLtStLgrstOtwdInwdPosMax_175_Val : Constant  Value=KeSMSw4sLyingMDSecRwLtStLgrstOtwdInwdPosMax_175_Val
  PA_KeSMSw4sLyingMDSecRwLtStLgrstOtwdInwdPosMax_180_Val : Constant  Value=KeSMSw4sLyingMDSecRwLtStLgrstOtwdInwdPosMax_180_Val
  PA_KeSMSw4sLyingMDSecRwLtStLgrstOtwdInwdPosMax_Below160_Val : Constant  Value=KeSMSw4sLyingMDSecRwLtStLgrstOtwdInwdPosMax_Below160_Val
  PA_KeSMSw4sLyingMDSecRwLtStLgrstOtwdInwdPosMax_Over180_Val : Constant  Value=KeSMSw4sLyingMDSecRwLtStLgrstOtwdInwdPosMax_Over180_Val
  PA_KeSMSw4sLyingMDSecRwLtStLgrstOtwdInwdPosMin_160_Val : Constant  Value=KeSMSw4sLyingMDSecRwLtStLgrstOtwdInwdPosMin_160_Val
  PA_KeSMSw4sLyingMDSecRwLtStLgrstOtwdInwdPosMin_165_Val : Constant  Value=KeSMSw4sLyingMDSecRwLtStLgrstOtwdInwdPosMin_165_Val
  PA_KeSMSw4sLyingMDSecRwLtStLgrstOtwdInwdPosMin_170_Val : Constant  Value=KeSMSw4sLyingMDSecRwLtStLgrstOtwdInwdPosMin_170_Val
  PA_KeSMSw4sLyingMDSecRwLtStLgrstOtwdInwdPosMin_175_Val : Constant  Value=KeSMSw4sLyingMDSecRwLtStLgrstOtwdInwdPosMin_175_Val
  PA_KeSMSw4sLyingMDSecRwLtStLgrstOtwdInwdPosMin_180_Val : Constant  Value=KeSMSw4sLyingMDSecRwLtStLgrstOtwdInwdPosMin_180_Val
  PA_KeSMSw4sLyingMDSecRwLtStLgrstOtwdInwdPosMin_Below160_Val : Constant  Value=KeSMSw4sLyingMDSecRwLtStLgrstOtwdInwdPosMin_Below160_Val
  PA_KeSMSw4sLyingMDSecRwLtStLgrstOtwdInwdPosMin_Over180_Val : Constant  Value=KeSMSw4sLyingMDSecRwLtStLgrstOtwdInwdPosMin_Over180_Val
  PA_KeSMSw4sLyingMDSecRwLtStLgrstOtwdInwdPos_160_Val : Constant  Value=KeSMSw4sLyingMDSecRwLtStLgrstOtwdInwdPos_160_Val
  PA_KeSMSw4sLyingMDSecRwLtStLgrstOtwdInwdPos_165_Val : Constant  Value=KeSMSw4sLyingMDSecRwLtStLgrstOtwdInwdPos_165_Val
  PA_KeSMSw4sLyingMDSecRwLtStLgrstOtwdInwdPos_170_Val : Constant  Value=KeSMSw4sLyingMDSecRwLtStLgrstOtwdInwdPos_170_Val
  PA_KeSMSw4sLyingMDSecRwLtStLgrstOtwdInwdPos_175_Val : Constant  Value=KeSMSw4sLyingMDSecRwLtStLgrstOtwdInwdPos_175_Val
  PA_KeSMSw4sLyingMDSecRwLtStLgrstOtwdInwdPos_180_Val : Constant  Value=KeSMSw4sLyingMDSecRwLtStLgrstOtwdInwdPos_180_Val
  PA_KeSMSw4sLyingMDSecRwLtStLgrstOtwdInwdPos_Below160_Val : Constant  Value=KeSMSw4sLyingMDSecRwLtStLgrstOtwdInwdPos_Below160_Val
  PA_KeSMSw4sLyingMDSecRwLtStLgrstOtwdInwdPos_Over180_Val : Constant  Value=KeSMSw4sLyingMDSecRwLtStLgrstOtwdInwdPos_Over180_Val
  PA_KeSMSw4sLyingMDSecRwLtStLgrstUpwdDnwdPosMax_Val : Constant  Value=KeSMSw4sLyingMDSecRwLtStLgrstUpwdDnwdPosMax_Val
  PA_KeSMSw4sLyingMDSecRwLtStLgrstUpwdDnwdPosMin_Val : Constant  Value=KeSMSw4sLyingMDSecRwLtStLgrstUpwdDnwdPosMin_Val
  PA_KeSMSw4sLyingMDSecRwLtStLgrstUpwdDnwdPos_Val : Constant  Value=KeSMSw4sLyingMDSecRwLtStLgrstUpwdDnwdPos_Val
  PA_KeSMSw4sRecoveryMDSecRwLtStBkReclnUpwdDnwdPosMax_Val : Constant  Value=KeSMSw4sRecoveryMDSecRwLtStBkReclnUpwdDnwdPosMax_Val
  PA_KeSMSw4sRecoveryMDSecRwLtStBkReclnUpwdDnwdPosMin_Val : Constant  Value=KeSMSw4sRecoveryMDSecRwLtStBkReclnUpwdDnwdPosMin_Val
  PA_KeSMSw4sRecoveryMDSecRwLtStBkReclnUpwdDnwdPos_Val : Constant  Value=KeSMSw4sRecoveryMDSecRwLtStBkReclnUpwdDnwdPos_Val
  PA_KeSMSw4sRecoveryMDSecRwLtStFtrstUpwdDnwdPosMax_Val : Constant  Value=KeSMSw4sRecoveryMDSecRwLtStFtrstUpwdDnwdPosMax_Val
  PA_KeSMSw4sRecoveryMDSecRwLtStFtrstUpwdDnwdPosMin_Val : Constant  Value=KeSMSw4sRecoveryMDSecRwLtStFtrstUpwdDnwdPosMin_Val
  PA_KeSMSw4sRecoveryMDSecRwLtStFtrstUpwdDnwdPos_Val : Constant  Value=KeSMSw4sRecoveryMDSecRwLtStFtrstUpwdDnwdPos_Val
  PA_KeSMSw4sRecoveryMDSecRwLtStHdrstFrwdBkwdPosMax_160_Val : Constant  Value=KeSMSw4sRecoveryMDSecRwLtStHdrstFrwdBkwdPosMax_160_Val
  PA_KeSMSw4sRecoveryMDSecRwLtStHdrstFrwdBkwdPosMax_165_Val : Constant  Value=KeSMSw4sRecoveryMDSecRwLtStHdrstFrwdBkwdPosMax_165_Val
  PA_KeSMSw4sRecoveryMDSecRwLtStHdrstFrwdBkwdPosMax_170_Val : Constant  Value=KeSMSw4sRecoveryMDSecRwLtStHdrstFrwdBkwdPosMax_170_Val
  PA_KeSMSw4sRecoveryMDSecRwLtStHdrstFrwdBkwdPosMax_175_Val : Constant  Value=KeSMSw4sRecoveryMDSecRwLtStHdrstFrwdBkwdPosMax_175_Val
  PA_KeSMSw4sRecoveryMDSecRwLtStHdrstFrwdBkwdPosMax_180_Val : Constant  Value=KeSMSw4sRecoveryMDSecRwLtStHdrstFrwdBkwdPosMax_180_Val
  PA_KeSMSw4sRecoveryMDSecRwLtStHdrstFrwdBkwdPosMax_Below160_Val : Constant  Value=KeSMSw4sRecoveryMDSecRwLtStHdrstFrwdBkwdPosMax_Below160_Val
  PA_KeSMSw4sRecoveryMDSecRwLtStHdrstFrwdBkwdPosMax_Over180_Val : Constant  Value=KeSMSw4sRecoveryMDSecRwLtStHdrstFrwdBkwdPosMax_Over180_Val
  PA_KeSMSw4sRecoveryMDSecRwLtStHdrstFrwdBkwdPosMin_160_Val : Constant  Value=KeSMSw4sRecoveryMDSecRwLtStHdrstFrwdBkwdPosMin_160_Val
  PA_KeSMSw4sRecoveryMDSecRwLtStHdrstFrwdBkwdPosMin_165_Val : Constant  Value=KeSMSw4sRecoveryMDSecRwLtStHdrstFrwdBkwdPosMin_165_Val
  PA_KeSMSw4sRecoveryMDSecRwLtStHdrstFrwdBkwdPosMin_170_Val : Constant  Value=KeSMSw4sRecoveryMDSecRwLtStHdrstFrwdBkwdPosMin_170_Val
  PA_KeSMSw4sRecoveryMDSecRwLtStHdrstFrwdBkwdPosMin_175_Val : Constant  Value=KeSMSw4sRecoveryMDSecRwLtStHdrstFrwdBkwdPosMin_175_Val
  PA_KeSMSw4sRecoveryMDSecRwLtStHdrstFrwdBkwdPosMin_180_Val : Constant  Value=KeSMSw4sRecoveryMDSecRwLtStHdrstFrwdBkwdPosMin_180_Val
  PA_KeSMSw4sRecoveryMDSecRwLtStHdrstFrwdBkwdPosMin_Below160_Val : Constant  Value=KeSMSw4sRecoveryMDSecRwLtStHdrstFrwdBkwdPosMin_Below160_Val
  PA_KeSMSw4sRecoveryMDSecRwLtStHdrstFrwdBkwdPosMin_Over180_Val : Constant  Value=KeSMSw4sRecoveryMDSecRwLtStHdrstFrwdBkwdPosMin_Over180_Val
  PA_KeSMSw4sRecoveryMDSecRwLtStHdrstFrwdBkwdPos_160_Val : Constant  Value=KeSMSw4sRecoveryMDSecRwLtStHdrstFrwdBkwdPos_160_Val
  PA_KeSMSw4sRecoveryMDSecRwLtStHdrstFrwdBkwdPos_165_Val : Constant  Value=KeSMSw4sRecoveryMDSecRwLtStHdrstFrwdBkwdPos_165_Val
  PA_KeSMSw4sRecoveryMDSecRwLtStHdrstFrwdBkwdPos_170_Val : Constant  Value=KeSMSw4sRecoveryMDSecRwLtStHdrstFrwdBkwdPos_170_Val
  PA_KeSMSw4sRecoveryMDSecRwLtStHdrstFrwdBkwdPos_175_Val : Constant  Value=KeSMSw4sRecoveryMDSecRwLtStHdrstFrwdBkwdPos_175_Val
  PA_KeSMSw4sRecoveryMDSecRwLtStHdrstFrwdBkwdPos_180_Val : Constant  Value=KeSMSw4sRecoveryMDSecRwLtStHdrstFrwdBkwdPos_180_Val
  PA_KeSMSw4sRecoveryMDSecRwLtStHdrstFrwdBkwdPos_Below160_Val : Constant  Value=KeSMSw4sRecoveryMDSecRwLtStHdrstFrwdBkwdPos_Below160_Val
  PA_KeSMSw4sRecoveryMDSecRwLtStHdrstFrwdBkwdPos_Over180_Val : Constant  Value=KeSMSw4sRecoveryMDSecRwLtStHdrstFrwdBkwdPos_Over180_Val
  PA_KeSMSw4sRecoveryMDSecRwLtStHdrstUpwdDnwdPosMax_160_Val : Constant  Value=KeSMSw4sRecoveryMDSecRwLtStHdrstUpwdDnwdPosMax_160_Val
  PA_KeSMSw4sRecoveryMDSecRwLtStHdrstUpwdDnwdPosMax_165_Val : Constant  Value=KeSMSw4sRecoveryMDSecRwLtStHdrstUpwdDnwdPosMax_165_Val
  PA_KeSMSw4sRecoveryMDSecRwLtStHdrstUpwdDnwdPosMax_170_Val : Constant  Value=KeSMSw4sRecoveryMDSecRwLtStHdrstUpwdDnwdPosMax_170_Val
  PA_KeSMSw4sRecoveryMDSecRwLtStHdrstUpwdDnwdPosMax_175_Val : Constant  Value=KeSMSw4sRecoveryMDSecRwLtStHdrstUpwdDnwdPosMax_175_Val
  PA_KeSMSw4sRecoveryMDSecRwLtStHdrstUpwdDnwdPosMax_180_Val : Constant  Value=KeSMSw4sRecoveryMDSecRwLtStHdrstUpwdDnwdPosMax_180_Val
  PA_KeSMSw4sRecoveryMDSecRwLtStHdrstUpwdDnwdPosMax_Below160_Val : Constant  Value=KeSMSw4sRecoveryMDSecRwLtStHdrstUpwdDnwdPosMax_Below160_Val
  PA_KeSMSw4sRecoveryMDSecRwLtStHdrstUpwdDnwdPosMax_Over180_Val : Constant  Value=KeSMSw4sRecoveryMDSecRwLtStHdrstUpwdDnwdPosMax_Over180_Val
  PA_KeSMSw4sRecoveryMDSecRwLtStHdrstUpwdDnwdPosMin_160_Val : Constant  Value=KeSMSw4sRecoveryMDSecRwLtStHdrstUpwdDnwdPosMin_160_Val
  PA_KeSMSw4sRecoveryMDSecRwLtStHdrstUpwdDnwdPosMin_165_Val : Constant  Value=KeSMSw4sRecoveryMDSecRwLtStHdrstUpwdDnwdPosMin_165_Val
  PA_KeSMSw4sRecoveryMDSecRwLtStHdrstUpwdDnwdPosMin_170_Val : Constant  Value=KeSMSw4sRecoveryMDSecRwLtStHdrstUpwdDnwdPosMin_170_Val
  PA_KeSMSw4sRecoveryMDSecRwLtStHdrstUpwdDnwdPosMin_175_Val : Constant  Value=KeSMSw4sRecoveryMDSecRwLtStHdrstUpwdDnwdPosMin_175_Val
  PA_KeSMSw4sRecoveryMDSecRwLtStHdrstUpwdDnwdPosMin_180_Val : Constant  Value=KeSMSw4sRecoveryMDSecRwLtStHdrstUpwdDnwdPosMin_180_Val
  PA_KeSMSw4sRecoveryMDSecRwLtStHdrstUpwdDnwdPosMin_Below160_Val : Constant  Value=KeSMSw4sRecoveryMDSecRwLtStHdrstUpwdDnwdPosMin_Below160_Val
  PA_KeSMSw4sRecoveryMDSecRwLtStHdrstUpwdDnwdPosMin_Over180_Val : Constant  Value=KeSMSw4sRecoveryMDSecRwLtStHdrstUpwdDnwdPosMin_Over180_Val
  PA_KeSMSw4sRecoveryMDSecRwLtStHdrstUpwdDnwdPos_160_Val : Constant  Value=KeSMSw4sRecoveryMDSecRwLtStHdrstUpwdDnwdPos_160_Val
  PA_KeSMSw4sRecoveryMDSecRwLtStHdrstUpwdDnwdPos_165_Val : Constant  Value=KeSMSw4sRecoveryMDSecRwLtStHdrstUpwdDnwdPos_165_Val
  PA_KeSMSw4sRecoveryMDSecRwLtStHdrstUpwdDnwdPos_170_Val : Constant  Value=KeSMSw4sRecoveryMDSecRwLtStHdrstUpwdDnwdPos_170_Val
  PA_KeSMSw4sRecoveryMDSecRwLtStHdrstUpwdDnwdPos_175_Val : Constant  Value=KeSMSw4sRecoveryMDSecRwLtStHdrstUpwdDnwdPos_175_Val
  PA_KeSMSw4sRecoveryMDSecRwLtStHdrstUpwdDnwdPos_180_Val : Constant  Value=KeSMSw4sRecoveryMDSecRwLtStHdrstUpwdDnwdPos_180_Val
  PA_KeSMSw4sRecoveryMDSecRwLtStHdrstUpwdDnwdPos_Below160_Val : Constant  Value=KeSMSw4sRecoveryMDSecRwLtStHdrstUpwdDnwdPos_Below160_Val
  PA_KeSMSw4sRecoveryMDSecRwLtStHdrstUpwdDnwdPos_Over180_Val : Constant  Value=KeSMSw4sRecoveryMDSecRwLtStHdrstUpwdDnwdPos_Over180_Val
  PA_KeSMSw4sRecoveryMDSecRwLtStLgrstOtwdInwdPosMax_160_Val : Constant  Value=KeSMSw4sRecoveryMDSecRwLtStLgrstOtwdInwdPosMax_160_Val
  PA_KeSMSw4sRecoveryMDSecRwLtStLgrstOtwdInwdPosMax_165_Val : Constant  Value=KeSMSw4sRecoveryMDSecRwLtStLgrstOtwdInwdPosMax_165_Val
  PA_KeSMSw4sRecoveryMDSecRwLtStLgrstOtwdInwdPosMax_170_Val : Constant  Value=KeSMSw4sRecoveryMDSecRwLtStLgrstOtwdInwdPosMax_170_Val
  PA_KeSMSw4sRecoveryMDSecRwLtStLgrstOtwdInwdPosMax_175_Val : Constant  Value=KeSMSw4sRecoveryMDSecRwLtStLgrstOtwdInwdPosMax_175_Val
  PA_KeSMSw4sRecoveryMDSecRwLtStLgrstOtwdInwdPosMax_180_Val : Constant  Value=KeSMSw4sRecoveryMDSecRwLtStLgrstOtwdInwdPosMax_180_Val
  PA_KeSMSw4sRecoveryMDSecRwLtStLgrstOtwdInwdPosMax_Below160_Val : Constant  Value=KeSMSw4sRecoveryMDSecRwLtStLgrstOtwdInwdPosMax_Below160_Val
  PA_KeSMSw4sRecoveryMDSecRwLtStLgrstOtwdInwdPosMax_Over180_Val : Constant  Value=KeSMSw4sRecoveryMDSecRwLtStLgrstOtwdInwdPosMax_Over180_Val
  PA_KeSMSw4sRecoveryMDSecRwLtStLgrstOtwdInwdPosMin_160_Val : Constant  Value=KeSMSw4sRecoveryMDSecRwLtStLgrstOtwdInwdPosMin_160_Val
  PA_KeSMSw4sRecoveryMDSecRwLtStLgrstOtwdInwdPosMin_165_Val : Constant  Value=KeSMSw4sRecoveryMDSecRwLtStLgrstOtwdInwdPosMin_165_Val
  PA_KeSMSw4sRecoveryMDSecRwLtStLgrstOtwdInwdPosMin_170_Val : Constant  Value=KeSMSw4sRecoveryMDSecRwLtStLgrstOtwdInwdPosMin_170_Val
  PA_KeSMSw4sRecoveryMDSecRwLtStLgrstOtwdInwdPosMin_175_Val : Constant  Value=KeSMSw4sRecoveryMDSecRwLtStLgrstOtwdInwdPosMin_175_Val
  PA_KeSMSw4sRecoveryMDSecRwLtStLgrstOtwdInwdPosMin_180_Val : Constant  Value=KeSMSw4sRecoveryMDSecRwLtStLgrstOtwdInwdPosMin_180_Val
  PA_KeSMSw4sRecoveryMDSecRwLtStLgrstOtwdInwdPosMin_Below160_Val : Constant  Value=KeSMSw4sRecoveryMDSecRwLtStLgrstOtwdInwdPosMin_Below160_Val
  PA_KeSMSw4sRecoveryMDSecRwLtStLgrstOtwdInwdPosMin_Over180_Val : Constant  Value=KeSMSw4sRecoveryMDSecRwLtStLgrstOtwdInwdPosMin_Over180_Val
  PA_KeSMSw4sRecoveryMDSecRwLtStLgrstOtwdInwdPos_160_Val : Constant  Value=KeSMSw4sRecoveryMDSecRwLtStLgrstOtwdInwdPos_160_Val
  PA_KeSMSw4sRecoveryMDSecRwLtStLgrstOtwdInwdPos_165_Val : Constant  Value=KeSMSw4sRecoveryMDSecRwLtStLgrstOtwdInwdPos_165_Val
  PA_KeSMSw4sRecoveryMDSecRwLtStLgrstOtwdInwdPos_170_Val : Constant  Value=KeSMSw4sRecoveryMDSecRwLtStLgrstOtwdInwdPos_170_Val
  PA_KeSMSw4sRecoveryMDSecRwLtStLgrstOtwdInwdPos_175_Val : Constant  Value=KeSMSw4sRecoveryMDSecRwLtStLgrstOtwdInwdPos_175_Val
  PA_KeSMSw4sRecoveryMDSecRwLtStLgrstOtwdInwdPos_180_Val : Constant  Value=KeSMSw4sRecoveryMDSecRwLtStLgrstOtwdInwdPos_180_Val
  PA_KeSMSw4sRecoveryMDSecRwLtStLgrstOtwdInwdPos_Below160_Val : Constant  Value=KeSMSw4sRecoveryMDSecRwLtStLgrstOtwdInwdPos_Below160_Val
  PA_KeSMSw4sRecoveryMDSecRwLtStLgrstOtwdInwdPos_Over180_Val : Constant  Value=KeSMSw4sRecoveryMDSecRwLtStLgrstOtwdInwdPos_Over180_Val
  PA_KeSMSw4sRecoveryMDSecRwLtStLgrstUpwdDnwdPosMax_Val : Constant  Value=KeSMSw4sRecoveryMDSecRwLtStLgrstUpwdDnwdPosMax_Val
  PA_KeSMSw4sRecoveryMDSecRwLtStLgrstUpwdDnwdPosMin_Val : Constant  Value=KeSMSw4sRecoveryMDSecRwLtStLgrstUpwdDnwdPosMin_Val
  PA_KeSMSw4sRecoveryMDSecRwLtStLgrstUpwdDnwdPos_Val : Constant  Value=KeSMSw4sRecoveryMDSecRwLtStLgrstUpwdDnwdPos_Val
  PA_KeSMSw4sVIPMDSecRwLtStBkReclnUpwdDnwdPosMax_Val : Constant  Value=KeSMSw4sVIPMDSecRwLtStBkReclnUpwdDnwdPosMax_Val
  PA_KeSMSw4sVIPMDSecRwLtStBkReclnUpwdDnwdPosMin_Val : Constant  Value=KeSMSw4sVIPMDSecRwLtStBkReclnUpwdDnwdPosMin_Val
  PA_KeSMSw4sVIPMDSecRwLtStBkReclnUpwdDnwdPos_Val : Constant  Value=KeSMSw4sVIPMDSecRwLtStBkReclnUpwdDnwdPos_Val
  PA_KeSMSw4sVIPMDSecRwLtStFtrstUpwdDnwdPosMax_Val : Constant  Value=KeSMSw4sVIPMDSecRwLtStFtrstUpwdDnwdPosMax_Val
  PA_KeSMSw4sVIPMDSecRwLtStFtrstUpwdDnwdPosMin_Val : Constant  Value=KeSMSw4sVIPMDSecRwLtStFtrstUpwdDnwdPosMin_Val
  PA_KeSMSw4sVIPMDSecRwLtStFtrstUpwdDnwdPos_Val : Constant  Value=KeSMSw4sVIPMDSecRwLtStFtrstUpwdDnwdPos_Val
  PA_KeSMSw4sVIPMDSecRwLtStHdrstFrwdBkwdPosMax_160_Val : Constant  Value=KeSMSw4sVIPMDSecRwLtStHdrstFrwdBkwdPosMax_160_Val
  PA_KeSMSw4sVIPMDSecRwLtStHdrstFrwdBkwdPosMax_165_Val : Constant  Value=KeSMSw4sVIPMDSecRwLtStHdrstFrwdBkwdPosMax_165_Val
  PA_KeSMSw4sVIPMDSecRwLtStHdrstFrwdBkwdPosMax_170_Val : Constant  Value=KeSMSw4sVIPMDSecRwLtStHdrstFrwdBkwdPosMax_170_Val
  PA_KeSMSw4sVIPMDSecRwLtStHdrstFrwdBkwdPosMax_175_Val : Constant  Value=KeSMSw4sVIPMDSecRwLtStHdrstFrwdBkwdPosMax_175_Val
  PA_KeSMSw4sVIPMDSecRwLtStHdrstFrwdBkwdPosMax_180_Val : Constant  Value=KeSMSw4sVIPMDSecRwLtStHdrstFrwdBkwdPosMax_180_Val
  PA_KeSMSw4sVIPMDSecRwLtStHdrstFrwdBkwdPosMax_Below160_Val : Constant  Value=KeSMSw4sVIPMDSecRwLtStHdrstFrwdBkwdPosMax_Below160_Val
  PA_KeSMSw4sVIPMDSecRwLtStHdrstFrwdBkwdPosMax_Over180_Val : Constant  Value=KeSMSw4sVIPMDSecRwLtStHdrstFrwdBkwdPosMax_Over180_Val
  PA_KeSMSw4sVIPMDSecRwLtStHdrstFrwdBkwdPosMin_160_Val : Constant  Value=KeSMSw4sVIPMDSecRwLtStHdrstFrwdBkwdPosMin_160_Val
  PA_KeSMSw4sVIPMDSecRwLtStHdrstFrwdBkwdPosMin_165_Val : Constant  Value=KeSMSw4sVIPMDSecRwLtStHdrstFrwdBkwdPosMin_165_Val
  PA_KeSMSw4sVIPMDSecRwLtStHdrstFrwdBkwdPosMin_170_Val : Constant  Value=KeSMSw4sVIPMDSecRwLtStHdrstFrwdBkwdPosMin_170_Val
  PA_KeSMSw4sVIPMDSecRwLtStHdrstFrwdBkwdPosMin_175_Val : Constant  Value=KeSMSw4sVIPMDSecRwLtStHdrstFrwdBkwdPosMin_175_Val
  PA_KeSMSw4sVIPMDSecRwLtStHdrstFrwdBkwdPosMin_180_Val : Constant  Value=KeSMSw4sVIPMDSecRwLtStHdrstFrwdBkwdPosMin_180_Val
  PA_KeSMSw4sVIPMDSecRwLtStHdrstFrwdBkwdPosMin_Below160_Val : Constant  Value=KeSMSw4sVIPMDSecRwLtStHdrstFrwdBkwdPosMin_Below160_Val
  PA_KeSMSw4sVIPMDSecRwLtStHdrstFrwdBkwdPosMin_Over180_Val : Constant  Value=KeSMSw4sVIPMDSecRwLtStHdrstFrwdBkwdPosMin_Over180_Val
  PA_KeSMSw4sVIPMDSecRwLtStHdrstFrwdBkwdPos_160_Val : Constant  Value=KeSMSw4sVIPMDSecRwLtStHdrstFrwdBkwdPos_160_Val
  PA_KeSMSw4sVIPMDSecRwLtStHdrstFrwdBkwdPos_165_Val : Constant  Value=KeSMSw4sVIPMDSecRwLtStHdrstFrwdBkwdPos_165_Val
  PA_KeSMSw4sVIPMDSecRwLtStHdrstFrwdBkwdPos_170_Val : Constant  Value=KeSMSw4sVIPMDSecRwLtStHdrstFrwdBkwdPos_170_Val
  PA_KeSMSw4sVIPMDSecRwLtStHdrstFrwdBkwdPos_175_Val : Constant  Value=KeSMSw4sVIPMDSecRwLtStHdrstFrwdBkwdPos_175_Val
  PA_KeSMSw4sVIPMDSecRwLtStHdrstFrwdBkwdPos_180_Val : Constant  Value=KeSMSw4sVIPMDSecRwLtStHdrstFrwdBkwdPos_180_Val
  PA_KeSMSw4sVIPMDSecRwLtStHdrstFrwdBkwdPos_Below160_Val : Constant  Value=KeSMSw4sVIPMDSecRwLtStHdrstFrwdBkwdPos_Below160_Val
  PA_KeSMSw4sVIPMDSecRwLtStHdrstFrwdBkwdPos_Over180_Val : Constant  Value=KeSMSw4sVIPMDSecRwLtStHdrstFrwdBkwdPos_Over180_Val
  PA_KeSMSw4sVIPMDSecRwLtStHdrstUpwdDnwdPosMax_160_Val : Constant  Value=KeSMSw4sVIPMDSecRwLtStHdrstUpwdDnwdPosMax_160_Val
  PA_KeSMSw4sVIPMDSecRwLtStHdrstUpwdDnwdPosMax_165_Val : Constant  Value=KeSMSw4sVIPMDSecRwLtStHdrstUpwdDnwdPosMax_165_Val
  PA_KeSMSw4sVIPMDSecRwLtStHdrstUpwdDnwdPosMax_170_Val : Constant  Value=KeSMSw4sVIPMDSecRwLtStHdrstUpwdDnwdPosMax_170_Val
  PA_KeSMSw4sVIPMDSecRwLtStHdrstUpwdDnwdPosMax_175_Val : Constant  Value=KeSMSw4sVIPMDSecRwLtStHdrstUpwdDnwdPosMax_175_Val
  PA_KeSMSw4sVIPMDSecRwLtStHdrstUpwdDnwdPosMax_180_Val : Constant  Value=KeSMSw4sVIPMDSecRwLtStHdrstUpwdDnwdPosMax_180_Val
  PA_KeSMSw4sVIPMDSecRwLtStHdrstUpwdDnwdPosMax_Below160_Val : Constant  Value=KeSMSw4sVIPMDSecRwLtStHdrstUpwdDnwdPosMax_Below160_Val
  PA_KeSMSw4sVIPMDSecRwLtStHdrstUpwdDnwdPosMax_Over180_Val : Constant  Value=KeSMSw4sVIPMDSecRwLtStHdrstUpwdDnwdPosMax_Over180_Val
  PA_KeSMSw4sVIPMDSecRwLtStHdrstUpwdDnwdPosMin_160_Val : Constant  Value=KeSMSw4sVIPMDSecRwLtStHdrstUpwdDnwdPosMin_160_Val
  PA_KeSMSw4sVIPMDSecRwLtStHdrstUpwdDnwdPosMin_165_Val : Constant  Value=KeSMSw4sVIPMDSecRwLtStHdrstUpwdDnwdPosMin_165_Val
  PA_KeSMSw4sVIPMDSecRwLtStHdrstUpwdDnwdPosMin_170_Val : Constant  Value=KeSMSw4sVIPMDSecRwLtStHdrstUpwdDnwdPosMin_170_Val
  PA_KeSMSw4sVIPMDSecRwLtStHdrstUpwdDnwdPosMin_175_Val : Constant  Value=KeSMSw4sVIPMDSecRwLtStHdrstUpwdDnwdPosMin_175_Val
  PA_KeSMSw4sVIPMDSecRwLtStHdrstUpwdDnwdPosMin_180_Val : Constant  Value=KeSMSw4sVIPMDSecRwLtStHdrstUpwdDnwdPosMin_180_Val
  PA_KeSMSw4sVIPMDSecRwLtStHdrstUpwdDnwdPosMin_Below160_Val : Constant  Value=KeSMSw4sVIPMDSecRwLtStHdrstUpwdDnwdPosMin_Below160_Val
  PA_KeSMSw4sVIPMDSecRwLtStHdrstUpwdDnwdPosMin_Over180_Val : Constant  Value=KeSMSw4sVIPMDSecRwLtStHdrstUpwdDnwdPosMin_Over180_Val
  PA_KeSMSw4sVIPMDSecRwLtStHdrstUpwdDnwdPos_160_Val : Constant  Value=KeSMSw4sVIPMDSecRwLtStHdrstUpwdDnwdPos_160_Val
  PA_KeSMSw4sVIPMDSecRwLtStHdrstUpwdDnwdPos_165_Val : Constant  Value=KeSMSw4sVIPMDSecRwLtStHdrstUpwdDnwdPos_165_Val
  PA_KeSMSw4sVIPMDSecRwLtStHdrstUpwdDnwdPos_170_Val : Constant  Value=KeSMSw4sVIPMDSecRwLtStHdrstUpwdDnwdPos_170_Val
  PA_KeSMSw4sVIPMDSecRwLtStHdrstUpwdDnwdPos_175_Val : Constant  Value=KeSMSw4sVIPMDSecRwLtStHdrstUpwdDnwdPos_175_Val
  PA_KeSMSw4sVIPMDSecRwLtStHdrstUpwdDnwdPos_180_Val : Constant  Value=KeSMSw4sVIPMDSecRwLtStHdrstUpwdDnwdPos_180_Val
  PA_KeSMSw4sVIPMDSecRwLtStHdrstUpwdDnwdPos_Below160_Val : Constant  Value=KeSMSw4sVIPMDSecRwLtStHdrstUpwdDnwdPos_Below160_Val
  PA_KeSMSw4sVIPMDSecRwLtStHdrstUpwdDnwdPos_Over180_Val : Constant  Value=KeSMSw4sVIPMDSecRwLtStHdrstUpwdDnwdPos_Over180_Val
  PA_KeSMSw4sVIPMDSecRwLtStLgrstOtwdInwdPosMax_160_Val : Constant  Value=KeSMSw4sVIPMDSecRwLtStLgrstOtwdInwdPosMax_160_Val
  PA_KeSMSw4sVIPMDSecRwLtStLgrstOtwdInwdPosMax_165_Val : Constant  Value=KeSMSw4sVIPMDSecRwLtStLgrstOtwdInwdPosMax_165_Val
  PA_KeSMSw4sVIPMDSecRwLtStLgrstOtwdInwdPosMax_170_Val : Constant  Value=KeSMSw4sVIPMDSecRwLtStLgrstOtwdInwdPosMax_170_Val
  PA_KeSMSw4sVIPMDSecRwLtStLgrstOtwdInwdPosMax_175_Val : Constant  Value=KeSMSw4sVIPMDSecRwLtStLgrstOtwdInwdPosMax_175_Val
  PA_KeSMSw4sVIPMDSecRwLtStLgrstOtwdInwdPosMax_180_Val : Constant  Value=KeSMSw4sVIPMDSecRwLtStLgrstOtwdInwdPosMax_180_Val
  PA_KeSMSw4sVIPMDSecRwLtStLgrstOtwdInwdPosMax_Below160_Val : Constant  Value=KeSMSw4sVIPMDSecRwLtStLgrstOtwdInwdPosMax_Below160_Val
  PA_KeSMSw4sVIPMDSecRwLtStLgrstOtwdInwdPosMax_Over180_Val : Constant  Value=KeSMSw4sVIPMDSecRwLtStLgrstOtwdInwdPosMax_Over180_Val
  PA_KeSMSw4sVIPMDSecRwLtStLgrstOtwdInwdPosMin_160_Val : Constant  Value=KeSMSw4sVIPMDSecRwLtStLgrstOtwdInwdPosMin_160_Val
  PA_KeSMSw4sVIPMDSecRwLtStLgrstOtwdInwdPosMin_165_Val : Constant  Value=KeSMSw4sVIPMDSecRwLtStLgrstOtwdInwdPosMin_165_Val
  PA_KeSMSw4sVIPMDSecRwLtStLgrstOtwdInwdPosMin_170_Val : Constant  Value=KeSMSw4sVIPMDSecRwLtStLgrstOtwdInwdPosMin_170_Val
  PA_KeSMSw4sVIPMDSecRwLtStLgrstOtwdInwdPosMin_175_Val : Constant  Value=KeSMSw4sVIPMDSecRwLtStLgrstOtwdInwdPosMin_175_Val
  PA_KeSMSw4sVIPMDSecRwLtStLgrstOtwdInwdPosMin_180_Val : Constant  Value=KeSMSw4sVIPMDSecRwLtStLgrstOtwdInwdPosMin_180_Val
  PA_KeSMSw4sVIPMDSecRwLtStLgrstOtwdInwdPosMin_Below160_Val : Constant  Value=KeSMSw4sVIPMDSecRwLtStLgrstOtwdInwdPosMin_Below160_Val
  PA_KeSMSw4sVIPMDSecRwLtStLgrstOtwdInwdPosMin_Over180_Val : Constant  Value=KeSMSw4sVIPMDSecRwLtStLgrstOtwdInwdPosMin_Over180_Val
  PA_KeSMSw4sVIPMDSecRwLtStLgrstOtwdInwdPos_160_Val : Constant  Value=KeSMSw4sVIPMDSecRwLtStLgrstOtwdInwdPos_160_Val
  PA_KeSMSw4sVIPMDSecRwLtStLgrstOtwdInwdPos_165_Val : Constant  Value=KeSMSw4sVIPMDSecRwLtStLgrstOtwdInwdPos_165_Val
  PA_KeSMSw4sVIPMDSecRwLtStLgrstOtwdInwdPos_170_Val : Constant  Value=KeSMSw4sVIPMDSecRwLtStLgrstOtwdInwdPos_170_Val
  PA_KeSMSw4sVIPMDSecRwLtStLgrstOtwdInwdPos_175_Val : Constant  Value=KeSMSw4sVIPMDSecRwLtStLgrstOtwdInwdPos_175_Val
  PA_KeSMSw4sVIPMDSecRwLtStLgrstOtwdInwdPos_180_Val : Constant  Value=KeSMSw4sVIPMDSecRwLtStLgrstOtwdInwdPos_180_Val
  PA_KeSMSw4sVIPMDSecRwLtStLgrstOtwdInwdPos_Below160_Val : Constant  Value=KeSMSw4sVIPMDSecRwLtStLgrstOtwdInwdPos_Below160_Val
  PA_KeSMSw4sVIPMDSecRwLtStLgrstOtwdInwdPos_Over180_Val : Constant  Value=KeSMSw4sVIPMDSecRwLtStLgrstOtwdInwdPos_Over180_Val
  PA_KeSMSw4sVIPMDSecRwLtStLgrstUpwdDnwdPosMax_Val : Constant  Value=KeSMSw4sVIPMDSecRwLtStLgrstUpwdDnwdPosMax_Val
  PA_KeSMSw4sVIPMDSecRwLtStLgrstUpwdDnwdPosMin_Val : Constant  Value=KeSMSw4sVIPMDSecRwLtStLgrstUpwdDnwdPosMin_Val
  PA_KeSMSw4sVIPMDSecRwLtStLgrstUpwdDnwdPos_Val : Constant  Value=KeSMSw4sVIPMDSecRwLtStLgrstUpwdDnwdPos_Val
  PA_KeSMSw6SAcsMd56SecRwLtStBkReclnUpwdDnwdPos1Max_Val : Constant  Value=KeSMSw6SAcsMd56SecRwLtStBkReclnUpwdDnwdPos1Max_Val
  PA_KeSMSw6SAcsMd56SecRwLtStBkReclnUpwdDnwdPos1Min_Val : Constant  Value=KeSMSw6SAcsMd56SecRwLtStBkReclnUpwdDnwdPos1Min_Val
  PA_KeSMSw6SAcsMd56SecRwLtStBkReclnUpwdDnwdPos1_Val : Constant  Value=KeSMSw6SAcsMd56SecRwLtStBkReclnUpwdDnwdPos1_Val
  PA_KeSMSw6SAcsMd56SecRwLtStBkReclnUpwdDnwdPosMax_Val : Constant  Value=KeSMSw6SAcsMd56SecRwLtStBkReclnUpwdDnwdPosMax_Val
  PA_KeSMSw6SAcsMd56SecRwLtStBkReclnUpwdDnwdPosMin_Val : Constant  Value=KeSMSw6SAcsMd56SecRwLtStBkReclnUpwdDnwdPosMin_Val
  PA_KeSMSw6SAcsMd56SecRwLtStBkReclnUpwdDnwdPos_Val : Constant  Value=KeSMSw6SAcsMd56SecRwLtStBkReclnUpwdDnwdPos_Val
  PA_KeSMSw6SAcsMd56SecRwLtStFrwdBkwdPosMax_Val : Constant  Value=KeSMSw6SAcsMd56SecRwLtStFrwdBkwdPosMax_Val
  PA_KeSMSw6SAcsMd56SecRwLtStFrwdBkwdPosMin_Val : Constant  Value=KeSMSw6SAcsMd56SecRwLtStFrwdBkwdPosMin_Val
  PA_KeSMSw6SAcsMd56SecRwLtStFrwdBkwdPos_Val : Constant  Value=KeSMSw6SAcsMd56SecRwLtStFrwdBkwdPos_Val
  PA_KeSMSw6SAcsMd56SecRwLtStLgrstInwdOtwdPosMax_Val : Constant  Value=KeSMSw6SAcsMd56SecRwLtStLgrstInwdOtwdPosMax_Val
  PA_KeSMSw6SAcsMd56SecRwLtStLgrstInwdOtwdPosMin_Val : Constant  Value=KeSMSw6SAcsMd56SecRwLtStLgrstInwdOtwdPosMin_Val
  PA_KeSMSw6SAcsMd56SecRwLtStLgrstInwdOtwdPos_Val : Constant  Value=KeSMSw6SAcsMd56SecRwLtStLgrstInwdOtwdPos_Val
  PA_KeSMSw6SAcsMd56SecRwLtStLgrstUpwdPosMax_Val : Constant  Value=KeSMSw6SAcsMd56SecRwLtStLgrstUpwdPosMax_Val
  PA_KeSMSw6SAcsMd56SecRwLtStLgrstUpwdPosMin_Val : Constant  Value=KeSMSw6SAcsMd56SecRwLtStLgrstUpwdPosMin_Val
  PA_KeSMSw6SAcsMd56SecRwLtStLgrstUpwdPos_Val : Constant  Value=KeSMSw6SAcsMd56SecRwLtStLgrstUpwdPos_Val
  PA_KeSMSw6SVIPMdSecRwLtStLgrstInwdOtwdPosMax_Val : Constant  Value=KeSMSw6SVIPMdSecRwLtStLgrstInwdOtwdPosMax_Val
  PA_KeSMSw6SVIPMdSecRwLtStLgrstInwdOtwdPosMin_Val : Constant  Value=KeSMSw6SVIPMdSecRwLtStLgrstInwdOtwdPosMin_Val
  PA_KeSMSw6SVIPMdSecRwLtStLgrstInwdOtwdPos_Val : Constant  Value=KeSMSw6SVIPMdSecRwLtStLgrstInwdOtwdPos_Val
  PA_KeSMSw6sAcsEntrySecRwLtStArmScrnPosMax_Val : Constant  Value=KeSMSw6sAcsEntrySecRwLtStArmScrnPosMax_Val
  PA_KeSMSw6sAcsEntrySecRwLtStArmScrnPosMin_Val : Constant  Value=KeSMSw6sAcsEntrySecRwLtStArmScrnPosMin_Val
  PA_KeSMSw6sAcsEntrySecRwLtStArmScrnPos_Val : Constant  Value=KeSMSw6sAcsEntrySecRwLtStArmScrnPos_Val
  PA_KeSMSw6sAcsEntrySecRwLtStBkReclnUpwdDnwd1Pos_Val : Constant  Value=KeSMSw6sAcsEntrySecRwLtStBkReclnUpwdDnwd1Pos_Val
  PA_KeSMSw6sAcsEntrySecRwLtStBkReclnUpwdDnwdPos1Max_Val : Constant  Value=KeSMSw6sAcsEntrySecRwLtStBkReclnUpwdDnwdPos1Max_Val
  PA_KeSMSw6sAcsEntrySecRwLtStBkReclnUpwdDnwdPos1Min_Val : Constant  Value=KeSMSw6sAcsEntrySecRwLtStBkReclnUpwdDnwdPos1Min_Val
  PA_KeSMSw6sAcsEntrySecRwLtStBkReclnUpwdDnwdPosMax_Val : Constant  Value=KeSMSw6sAcsEntrySecRwLtStBkReclnUpwdDnwdPosMax_Val
  PA_KeSMSw6sAcsEntrySecRwLtStBkReclnUpwdDnwdPosMin_Val : Constant  Value=KeSMSw6sAcsEntrySecRwLtStBkReclnUpwdDnwdPosMin_Val
  PA_KeSMSw6sAcsEntrySecRwLtStBkReclnUpwdDnwdPos_Val : Constant  Value=KeSMSw6sAcsEntrySecRwLtStBkReclnUpwdDnwdPos_Val
  PA_KeSMSw6sAcsEntrySecRwLtStFrwdBkwdPosMax_Val : Constant  Value=KeSMSw6sAcsEntrySecRwLtStFrwdBkwdPosMax_Val
  PA_KeSMSw6sAcsEntrySecRwLtStFrwdBkwdPosMin_Val : Constant  Value=KeSMSw6sAcsEntrySecRwLtStFrwdBkwdPosMin_Val
  PA_KeSMSw6sAcsEntrySecRwLtStFrwdBkwdPos_Val : Constant  Value=KeSMSw6sAcsEntrySecRwLtStFrwdBkwdPos_Val
  PA_KeSMSw6sAcsEntrySecRwLtStLgrstInwdOtwdPosMax_Val : Constant  Value=KeSMSw6sAcsEntrySecRwLtStLgrstInwdOtwdPosMax_Val
  PA_KeSMSw6sAcsEntrySecRwLtStLgrstInwdOtwdPosMin_Val : Constant  Value=KeSMSw6sAcsEntrySecRwLtStLgrstInwdOtwdPosMin_Val
  PA_KeSMSw6sAcsEntrySecRwLtStLgrstInwdOtwdPos_Val : Constant  Value=KeSMSw6sAcsEntrySecRwLtStLgrstInwdOtwdPos_Val
  PA_KeSMSw6sAcsEntrySecRwLtStLgrstUpwdPosMax_Val : Constant  Value=KeSMSw6sAcsEntrySecRwLtStLgrstUpwdPosMax_Val
  PA_KeSMSw6sAcsEntrySecRwLtStLgrstUpwdPosMin_Val : Constant  Value=KeSMSw6sAcsEntrySecRwLtStLgrstUpwdPosMin_Val
  PA_KeSMSw6sAcsEntrySecRwLtStLgrstUpwdPos_Val : Constant  Value=KeSMSw6sAcsEntrySecRwLtStLgrstUpwdPos_Val
  PA_KeSMSw6sAcsEntrySecRwLtStLtwdRtwdPosMax_Val : Constant  Value=KeSMSw6sAcsEntrySecRwLtStLtwdRtwdPosMax_Val
  PA_KeSMSw6sAcsEntrySecRwLtStLtwdRtwdPosMin_Val : Constant  Value=KeSMSw6sAcsEntrySecRwLtStLtwdRtwdPosMin_Val
  PA_KeSMSw6sAcsEntrySecRwLtStLtwdRtwdPos_Val : Constant  Value=KeSMSw6sAcsEntrySecRwLtStLtwdRtwdPos_Val
  PA_KeSMSw6sAcsExtSecRwLtStArmScrnPosMax_Val : Constant  Value=KeSMSw6sAcsExtSecRwLtStArmScrnPosMax_Val
  PA_KeSMSw6sAcsExtSecRwLtStArmScrnPosMin_Val : Constant  Value=KeSMSw6sAcsExtSecRwLtStArmScrnPosMin_Val
  PA_KeSMSw6sAcsExtSecRwLtStArmScrnPos_Val : Constant  Value=KeSMSw6sAcsExtSecRwLtStArmScrnPos_Val
  PA_KeSMSw6sAcsExtSecRwLtStBkReclnUpwdDnwdPosMax_Val : Constant  Value=KeSMSw6sAcsExtSecRwLtStBkReclnUpwdDnwdPosMax_Val
  PA_KeSMSw6sAcsExtSecRwLtStBkReclnUpwdDnwdPosMin_Val : Constant  Value=KeSMSw6sAcsExtSecRwLtStBkReclnUpwdDnwdPosMin_Val
  PA_KeSMSw6sAcsExtSecRwLtStBkReclnUpwdDnwdPos_Val : Constant  Value=KeSMSw6sAcsExtSecRwLtStBkReclnUpwdDnwdPos_Val
  PA_KeSMSw6sAcsExtSecRwLtStFrwdBkwdPosMax_Val : Constant  Value=KeSMSw6sAcsExtSecRwLtStFrwdBkwdPosMax_Val
  PA_KeSMSw6sAcsExtSecRwLtStFrwdBkwdPosMin_Val : Constant  Value=KeSMSw6sAcsExtSecRwLtStFrwdBkwdPosMin_Val
  PA_KeSMSw6sAcsExtSecRwLtStFrwdBkwdPos_Val : Constant  Value=KeSMSw6sAcsExtSecRwLtStFrwdBkwdPos_Val
  PA_KeSMSw6sAcsExtSecRwLtStLgrstUpwdDnwdPosMax_Val : Constant  Value=KeSMSw6sAcsExtSecRwLtStLgrstUpwdDnwdPosMax_Val
  PA_KeSMSw6sAcsExtSecRwLtStLgrstUpwdDnwdPosMin_Val : Constant  Value=KeSMSw6sAcsExtSecRwLtStLgrstUpwdDnwdPosMin_Val
  PA_KeSMSw6sAcsExtSecRwLtStLgrstUpwdDnwdPos_Val : Constant  Value=KeSMSw6sAcsExtSecRwLtStLgrstUpwdDnwdPos_Val
  PA_KeSMSw6sAcsExtSecRwLtStLtwdRtwdPosMax_Val : Constant  Value=KeSMSw6sAcsExtSecRwLtStLtwdRtwdPosMax_Val
  PA_KeSMSw6sAcsExtSecRwLtStLtwdRtwdPosMin_Val : Constant  Value=KeSMSw6sAcsExtSecRwLtStLtwdRtwdPosMin_Val
  PA_KeSMSw6sAcsExtSecRwLtStLtwdRtwdPos_Val : Constant  Value=KeSMSw6sAcsExtSecRwLtStLtwdRtwdPos_Val
  PA_KeSMSw6sFamilyMdSecRwLtStFrwdBkwdPosMax_Val : Constant  Value=KeSMSw6sFamilyMdSecRwLtStFrwdBkwdPosMax_Val
  PA_KeSMSw6sFamilyMdSecRwLtStFrwdBkwdPosMin_Val : Constant  Value=KeSMSw6sFamilyMdSecRwLtStFrwdBkwdPosMin_Val
  PA_KeSMSw6sFamilyMdSecRwLtStFrwdBkwdPos_Val : Constant  Value=KeSMSw6sFamilyMdSecRwLtStFrwdBkwdPos_Val
  PA_KeSMSw6sFamilyMdSecRwLtStLtwdRtwdPosMax_Val : Constant  Value=KeSMSw6sFamilyMdSecRwLtStLtwdRtwdPosMax_Val
  PA_KeSMSw6sFamilyMdSecRwLtStLtwdRtwdPosMin_Val : Constant  Value=KeSMSw6sFamilyMdSecRwLtStLtwdRtwdPosMin_Val
  PA_KeSMSw6sFamilyMdSecRwLtStLtwdRtwdPos_Val : Constant  Value=KeSMSw6sFamilyMdSecRwLtStLtwdRtwdPos_Val
  PA_KeSMSw6sFamilyRMdSecRwLtStFrwdBkwdPosMax_Val : Constant  Value=KeSMSw6sFamilyRMdSecRwLtStFrwdBkwdPosMax_Val
  PA_KeSMSw6sFamilyRMdSecRwLtStFrwdBkwdPosMin_Val : Constant  Value=KeSMSw6sFamilyRMdSecRwLtStFrwdBkwdPosMin_Val
  PA_KeSMSw6sFamilyRMdSecRwLtStFrwdBkwdPos_Val : Constant  Value=KeSMSw6sFamilyRMdSecRwLtStFrwdBkwdPos_Val
  PA_KeSMSw6sFamilyRMdSecRwLtStLtwdRtwdPosMax_Val : Constant  Value=KeSMSw6sFamilyRMdSecRwLtStLtwdRtwdPosMax_Val
  PA_KeSMSw6sFamilyRMdSecRwLtStLtwdRtwdPosMin_Val : Constant  Value=KeSMSw6sFamilyRMdSecRwLtStLtwdRtwdPosMin_Val
  PA_KeSMSw6sFamilyRMdSecRwLtStLtwdRtwdPos_Val : Constant  Value=KeSMSw6sFamilyRMdSecRwLtStLtwdRtwdPos_Val
  PA_KeSMSw6sIntimacyMdSecRwLtStLtwdRtwdPosMax_Val : Constant  Value=KeSMSw6sIntimacyMdSecRwLtStLtwdRtwdPosMax_Val
  PA_KeSMSw6sIntimacyMdSecRwLtStLtwdRtwdPosMin_Val : Constant  Value=KeSMSw6sIntimacyMdSecRwLtStLtwdRtwdPosMin_Val
  PA_KeSMSw6sIntimacyMdSecRwLtStLtwdRtwdPos_Val : Constant  Value=KeSMSw6sIntimacyMdSecRwLtStLtwdRtwdPos_Val
  PA_KeSMSw6sIntimacyRMdSecRwLtStLtwdRtwdPosMax_Val : Constant  Value=KeSMSw6sIntimacyRMdSecRwLtStLtwdRtwdPosMax_Val
  PA_KeSMSw6sIntimacyRMdSecRwLtStLtwdRtwdPosMin_Val : Constant  Value=KeSMSw6sIntimacyRMdSecRwLtStLtwdRtwdPosMin_Val
  PA_KeSMSw6sIntimacyRMdSecRwLtStLtwdRtwdPos_Val : Constant  Value=KeSMSw6sIntimacyRMdSecRwLtStLtwdRtwdPos_Val
  PA_KeSMSw6sRecoveryMdSecRwLtStBkReclnUpwdDnwdPosMax_Val : Constant  Value=KeSMSw6sRecoveryMdSecRwLtStBkReclnUpwdDnwdPosMax_Val
  PA_KeSMSw6sRecoveryMdSecRwLtStBkReclnUpwdDnwdPosMin_Val : Constant  Value=KeSMSw6sRecoveryMdSecRwLtStBkReclnUpwdDnwdPosMin_Val
  PA_KeSMSw6sRecoveryMdSecRwLtStBkReclnUpwdDnwdPos_Val : Constant  Value=KeSMSw6sRecoveryMdSecRwLtStBkReclnUpwdDnwdPos_Val
  PA_KeSMSw6sRecoveryMdSecRwLtStLgrstInwdOtwdPosMax_Val : Constant  Value=KeSMSw6sRecoveryMdSecRwLtStLgrstInwdOtwdPosMax_Val
  PA_KeSMSw6sRecoveryMdSecRwLtStLgrstInwdOtwdPosMin_Val : Constant  Value=KeSMSw6sRecoveryMdSecRwLtStLgrstInwdOtwdPosMin_Val
  PA_KeSMSw6sRecoveryMdSecRwLtStLgrstInwdOtwdPos_Val : Constant  Value=KeSMSw6sRecoveryMdSecRwLtStLgrstInwdOtwdPos_Val
  PA_KeSMSw6sRecoveryMdSecRwLtStLgrstUpwdDnwdPosMax_Val : Constant  Value=KeSMSw6sRecoveryMdSecRwLtStLgrstUpwdDnwdPosMax_Val
  PA_KeSMSw6sRecoveryMdSecRwLtStLgrstUpwdDnwdPosMin_Val : Constant  Value=KeSMSw6sRecoveryMdSecRwLtStLgrstUpwdDnwdPosMin_Val
  PA_KeSMSw6sRecoveryMdSecRwLtStLgrstUpwdDnwdPos_Val : Constant  Value=KeSMSw6sRecoveryMdSecRwLtStLgrstUpwdDnwdPos_Val
  PA_KeSMSw6sVIPSecRwLtStBkReclnUpwdDnwdPosMax_Val : Constant  Value=KeSMSw6sVIPSecRwLtStBkReclnUpwdDnwdPosMax_Val
  PA_KeSMSw6sVIPSecRwLtStBkReclnUpwdDnwdPosMin_Val : Constant  Value=KeSMSw6sVIPSecRwLtStBkReclnUpwdDnwdPosMin_Val
  PA_KeSMSw6sVIPSecRwLtStBkReclnUpwdDnwdPos_Val : Constant  Value=KeSMSw6sVIPSecRwLtStBkReclnUpwdDnwdPos_Val
  PA_KeSMSw6sVIPSecRwLtStFrwdBkwdPosMax_Val : Constant  Value=KeSMSw6sVIPSecRwLtStFrwdBkwdPosMax_Val
  PA_KeSMSw6sVIPSecRwLtStFrwdBkwdPosMin_Val : Constant  Value=KeSMSw6sVIPSecRwLtStFrwdBkwdPosMin_Val
  PA_KeSMSw6sVIPSecRwLtStFrwdBkwdPos_Val : Constant  Value=KeSMSw6sVIPSecRwLtStFrwdBkwdPos_Val
  PA_KeSMSw6sVIPSecRwLtStLgrstUpwdPosMax_Val : Constant  Value=KeSMSw6sVIPSecRwLtStLgrstUpwdPosMax_Val
  PA_KeSMSw6sVIPSecRwLtStLgrstUpwdPosMin_Val : Constant  Value=KeSMSw6sVIPSecRwLtStLgrstUpwdPosMin_Val
  PA_KeSMSw6sVIPSecRwLtStLgrstUpwdPos_Val : Constant  Value=KeSMSw6sVIPSecRwLtStLgrstUpwdPos_Val
  PA_KeSMSw6sVIPSecRwLtStLtwdRtwdPosMax_Val : Constant  Value=KeSMSw6sVIPSecRwLtStLtwdRtwdPosMax_Val
  PA_KeSMSw6sVIPSecRwLtStLtwdRtwdPosMin_Val : Constant  Value=KeSMSw6sVIPSecRwLtStLtwdRtwdPosMin_Val
  PA_KeSMSw6sVIPSecRwLtStLtwdRtwdPos_Val : Constant  Value=KeSMSw6sVIPSecRwLtStLtwdRtwdPos_Val
  PA_KeSMSwAcsEntrySecRwLtStArmScrnPosMax_Val : Constant  Value=KeSMSwAcsEntrySecRwLtStArmScrnPosMax_Val
  PA_KeSMSwAcsEntrySecRwLtStArmScrnPosMin_Val : Constant  Value=KeSMSwAcsEntrySecRwLtStArmScrnPosMin_Val
  PA_KeSMSwAcsEntrySecRwLtStArmScrnPos_Val : Constant  Value=KeSMSwAcsEntrySecRwLtStArmScrnPos_Val
  PA_KeSMSwAcsEntrySecRwLtStBkReclnUpwdDnwdPos1Max_Val : Constant  Value=KeSMSwAcsEntrySecRwLtStBkReclnUpwdDnwdPos1Max_Val
  PA_KeSMSwAcsEntrySecRwLtStBkReclnUpwdDnwdPos1Min_Val : Constant  Value=KeSMSwAcsEntrySecRwLtStBkReclnUpwdDnwdPos1Min_Val
  PA_KeSMSwAcsEntrySecRwLtStBkReclnUpwdDnwdPos1_Val : Constant  Value=KeSMSwAcsEntrySecRwLtStBkReclnUpwdDnwdPos1_Val
  PA_KeSMSwAcsEntrySecRwLtStBkReclnUpwdDnwdPosMax_Val : Constant  Value=KeSMSwAcsEntrySecRwLtStBkReclnUpwdDnwdPosMax_Val
  PA_KeSMSwAcsEntrySecRwLtStBkReclnUpwdDnwdPosMin_Val : Constant  Value=KeSMSwAcsEntrySecRwLtStBkReclnUpwdDnwdPosMin_Val
  PA_KeSMSwAcsEntrySecRwLtStBkReclnUpwdDnwdPos_Val : Constant  Value=KeSMSwAcsEntrySecRwLtStBkReclnUpwdDnwdPos_Val
  PA_KeSMSwAcsEntrySecRwLtStFrwdBkwdPosMax_Val : Constant  Value=KeSMSwAcsEntrySecRwLtStFrwdBkwdPosMax_Val
  PA_KeSMSwAcsEntrySecRwLtStFrwdBkwdPosMin_Val : Constant  Value=KeSMSwAcsEntrySecRwLtStFrwdBkwdPosMin_Val
  PA_KeSMSwAcsEntrySecRwLtStFrwdBkwdPos_Val : Constant  Value=KeSMSwAcsEntrySecRwLtStFrwdBkwdPos_Val
  PA_KeSMSwAcsEntrySecRwLtStLgrstInwdOtwdPosMax_Val : Constant  Value=KeSMSwAcsEntrySecRwLtStLgrstInwdOtwdPosMax_Val
  PA_KeSMSwAcsEntrySecRwLtStLgrstInwdOtwdPosMin_Val : Constant  Value=KeSMSwAcsEntrySecRwLtStLgrstInwdOtwdPosMin_Val
  PA_KeSMSwAcsEntrySecRwLtStLgrstInwdOtwdPos_Val : Constant  Value=KeSMSwAcsEntrySecRwLtStLgrstInwdOtwdPos_Val
  PA_KeSMSwAcsEntrySecRwLtStLgrstUpwdPosMax_Val : Constant  Value=KeSMSwAcsEntrySecRwLtStLgrstUpwdPosMax_Val
  PA_KeSMSwAcsEntrySecRwLtStLgrstUpwdPosMin_Val : Constant  Value=KeSMSwAcsEntrySecRwLtStLgrstUpwdPosMin_Val
  PA_KeSMSwAcsEntrySecRwLtStLgrstUpwdPos_Val : Constant  Value=KeSMSwAcsEntrySecRwLtStLgrstUpwdPos_Val
  PA_KeSMSwAcsEntrySecRwLtStLtwdRtwdPosMax_Val : Constant  Value=KeSMSwAcsEntrySecRwLtStLtwdRtwdPosMax_Val
  PA_KeSMSwAcsEntrySecRwLtStLtwdRtwdPosMin_Val : Constant  Value=KeSMSwAcsEntrySecRwLtStLtwdRtwdPosMin_Val
  PA_KeSMSwAcsEntrySecRwLtStLtwdRtwdPos_Val : Constant  Value=KeSMSwAcsEntrySecRwLtStLtwdRtwdPos_Val
  PA_KeSMSwAcsExtSecRwLtStArmScrnPosMax_Val : Constant  Value=KeSMSwAcsExtSecRwLtStArmScrnPosMax_Val
  PA_KeSMSwAcsExtSecRwLtStArmScrnPosMin_Val : Constant  Value=KeSMSwAcsExtSecRwLtStArmScrnPosMin_Val
  PA_KeSMSwAcsExtSecRwLtStArmScrnPos_Val : Constant  Value=KeSMSwAcsExtSecRwLtStArmScrnPos_Val
  PA_KeSMSwAcsExtSecRwLtStBkReclnUpwdDnwdPosMax_Val : Constant  Value=KeSMSwAcsExtSecRwLtStBkReclnUpwdDnwdPosMax_Val
  PA_KeSMSwAcsExtSecRwLtStBkReclnUpwdDnwdPosMin_Val : Constant  Value=KeSMSwAcsExtSecRwLtStBkReclnUpwdDnwdPosMin_Val
  PA_KeSMSwAcsExtSecRwLtStBkReclnUpwdDnwdPos_Val : Constant  Value=KeSMSwAcsExtSecRwLtStBkReclnUpwdDnwdPos_Val
  PA_KeSMSwAcsExtSecRwLtStFrwdBkwdPosMax_Val : Constant  Value=KeSMSwAcsExtSecRwLtStFrwdBkwdPosMax_Val
  PA_KeSMSwAcsExtSecRwLtStFrwdBkwdPosMin_Val : Constant  Value=KeSMSwAcsExtSecRwLtStFrwdBkwdPosMin_Val
  PA_KeSMSwAcsExtSecRwLtStFrwdBkwdPos_Val : Constant  Value=KeSMSwAcsExtSecRwLtStFrwdBkwdPos_Val
  PA_KeSMSwAcsExtSecRwLtStLgrstUpwdDnwdPosMax_Val : Constant  Value=KeSMSwAcsExtSecRwLtStLgrstUpwdDnwdPosMax_Val
  PA_KeSMSwAcsExtSecRwLtStLgrstUpwdDnwdPosMin_Val : Constant  Value=KeSMSwAcsExtSecRwLtStLgrstUpwdDnwdPosMin_Val
  PA_KeSMSwAcsExtSecRwLtStLgrstUpwdDnwdPos_Val : Constant  Value=KeSMSwAcsExtSecRwLtStLgrstUpwdDnwdPos_Val
  PA_KeSMSwAcsExtSecRwLtStLtwdRtwdPosMax_Val : Constant  Value=KeSMSwAcsExtSecRwLtStLtwdRtwdPosMax_Val
  PA_KeSMSwAcsExtSecRwLtStLtwdRtwdPosMin_Val : Constant  Value=KeSMSwAcsExtSecRwLtStLtwdRtwdPosMin_Val
  PA_KeSMSwAcsExtSecRwLtStLtwdRtwdPos_Val : Constant  Value=KeSMSwAcsExtSecRwLtStLtwdRtwdPos_Val
  PA_KeSMSwAcsMd32SecRwLtStBkReclnUpwdDnwdPos1Max_Val : Constant  Value=KeSMSwAcsMd32SecRwLtStBkReclnUpwdDnwdPos1Max_Val
  PA_KeSMSwAcsMd32SecRwLtStBkReclnUpwdDnwdPos1Min_Val : Constant  Value=KeSMSwAcsMd32SecRwLtStBkReclnUpwdDnwdPos1Min_Val
  PA_KeSMSwAcsMd32SecRwLtStBkReclnUpwdDnwdPos1_Val : Constant  Value=KeSMSwAcsMd32SecRwLtStBkReclnUpwdDnwdPos1_Val
  PA_KeSMSwAcsMd32SecRwLtStBkReclnUpwdDnwdPosMax_Val : Constant  Value=KeSMSwAcsMd32SecRwLtStBkReclnUpwdDnwdPosMax_Val
  PA_KeSMSwAcsMd32SecRwLtStBkReclnUpwdDnwdPosMin_Val : Constant  Value=KeSMSwAcsMd32SecRwLtStBkReclnUpwdDnwdPosMin_Val
  PA_KeSMSwAcsMd32SecRwLtStBkReclnUpwdDnwdPos_Val : Constant  Value=KeSMSwAcsMd32SecRwLtStBkReclnUpwdDnwdPos_Val
  PA_KeSMSwAcsMd56SecRwLtStBkReclnUpwdDnwdPos1Max_Val : Constant  Value=KeSMSwAcsMd56SecRwLtStBkReclnUpwdDnwdPos1Max_Val
  PA_KeSMSwAcsMd56SecRwLtStBkReclnUpwdDnwdPos1Min_Val : Constant  Value=KeSMSwAcsMd56SecRwLtStBkReclnUpwdDnwdPos1Min_Val
  PA_KeSMSwAcsMd56SecRwLtStBkReclnUpwdDnwdPos1_Val : Constant  Value=KeSMSwAcsMd56SecRwLtStBkReclnUpwdDnwdPos1_Val
  PA_KeSMSwAcsMd56SecRwLtStBkReclnUpwdDnwdPosMax_Val : Constant  Value=KeSMSwAcsMd56SecRwLtStBkReclnUpwdDnwdPosMax_Val
  PA_KeSMSwAcsMd56SecRwLtStBkReclnUpwdDnwdPosMin_Val : Constant  Value=KeSMSwAcsMd56SecRwLtStBkReclnUpwdDnwdPosMin_Val
  PA_KeSMSwAcsMd56SecRwLtStBkReclnUpwdDnwdPos_Val : Constant  Value=KeSMSwAcsMd56SecRwLtStBkReclnUpwdDnwdPos_Val
  PA_KeSMSwAcsMd56SecRwLtStFrwdBkwdPosMax_Val : Constant  Value=KeSMSwAcsMd56SecRwLtStFrwdBkwdPosMax_Val
  PA_KeSMSwAcsMd56SecRwLtStFrwdBkwdPosMin_Val : Constant  Value=KeSMSwAcsMd56SecRwLtStFrwdBkwdPosMin_Val
  PA_KeSMSwAcsMd56SecRwLtStFrwdBkwdPos_Val : Constant  Value=KeSMSwAcsMd56SecRwLtStFrwdBkwdPos_Val
  PA_KeSMSwAcsMd56SecRwLtStLgrstInwdOtwdPosMax_Val : Constant  Value=KeSMSwAcsMd56SecRwLtStLgrstInwdOtwdPosMax_Val
  PA_KeSMSwAcsMd56SecRwLtStLgrstInwdOtwdPosMin_Val : Constant  Value=KeSMSwAcsMd56SecRwLtStLgrstInwdOtwdPosMin_Val
  PA_KeSMSwAcsMd56SecRwLtStLgrstInwdOtwdPos_Val : Constant  Value=KeSMSwAcsMd56SecRwLtStLgrstInwdOtwdPos_Val
  PA_KeSMSwAcsMd56SecRwLtStLgrstUpwdPosMax_Val : Constant  Value=KeSMSwAcsMd56SecRwLtStLgrstUpwdPosMax_Val
  PA_KeSMSwAcsMd56SecRwLtStLgrstUpwdPosMin_Val : Constant  Value=KeSMSwAcsMd56SecRwLtStLgrstUpwdPosMin_Val
  PA_KeSMSwAcsMd56SecRwLtStLgrstUpwdPos_Val : Constant  Value=KeSMSwAcsMd56SecRwLtStLgrstUpwdPos_Val
  PA_KeSMSwAcsMd6SecRwLtStBkReclnUpwdDnwdPos1Max_Val : Constant  Value=KeSMSwAcsMd6SecRwLtStBkReclnUpwdDnwdPos1Max_Val
  PA_KeSMSwAcsMd6SecRwLtStBkReclnUpwdDnwdPos1Min_Val : Constant  Value=KeSMSwAcsMd6SecRwLtStBkReclnUpwdDnwdPos1Min_Val
  PA_KeSMSwAcsMd6SecRwLtStBkReclnUpwdDnwdPos1_Val : Constant  Value=KeSMSwAcsMd6SecRwLtStBkReclnUpwdDnwdPos1_Val
  PA_KeSMSwAcsMd6SecRwLtStBkReclnUpwdDnwdPosMax_Val : Constant  Value=KeSMSwAcsMd6SecRwLtStBkReclnUpwdDnwdPosMax_Val
  PA_KeSMSwAcsMd6SecRwLtStBkReclnUpwdDnwdPosMin_Val : Constant  Value=KeSMSwAcsMd6SecRwLtStBkReclnUpwdDnwdPosMin_Val
  PA_KeSMSwAcsMd6SecRwLtStBkReclnUpwdDnwdPos_Val : Constant  Value=KeSMSwAcsMd6SecRwLtStBkReclnUpwdDnwdPos_Val
  PA_KeSMSwAcsMd8SecRwLtStBkReclnUpwdDnwdPosMax_Val : Constant  Value=KeSMSwAcsMd8SecRwLtStBkReclnUpwdDnwdPosMax_Val
  PA_KeSMSwAcsMd8SecRwLtStBkReclnUpwdDnwdPosMin_Val : Constant  Value=KeSMSwAcsMd8SecRwLtStBkReclnUpwdDnwdPosMin_Val
  PA_KeSMSwAcsMd8SecRwLtStBkReclnUpwdDnwdPos_Val : Constant  Value=KeSMSwAcsMd8SecRwLtStBkReclnUpwdDnwdPos_Val
  PA_KeSMSwAcsMd8SecRwLtStFrwdBkwdPosMax_Val : Constant  Value=KeSMSwAcsMd8SecRwLtStFrwdBkwdPosMax_Val
  PA_KeSMSwAcsMd8SecRwLtStFrwdBkwdPosMin_Val : Constant  Value=KeSMSwAcsMd8SecRwLtStFrwdBkwdPosMin_Val
  PA_KeSMSwAcsMd8SecRwLtStFrwdBkwdPos_Val : Constant  Value=KeSMSwAcsMd8SecRwLtStFrwdBkwdPos_Val
  PA_KeSMSwAcsMd8SecRwLtStLgrstInwdOtwdPosMax_Val : Constant  Value=KeSMSwAcsMd8SecRwLtStLgrstInwdOtwdPosMax_Val
  PA_KeSMSwAcsMd8SecRwLtStLgrstInwdOtwdPosMin_Val : Constant  Value=KeSMSwAcsMd8SecRwLtStLgrstInwdOtwdPosMin_Val
  PA_KeSMSwAcsMd8SecRwLtStLgrstInwdOtwdPos_Val : Constant  Value=KeSMSwAcsMd8SecRwLtStLgrstInwdOtwdPos_Val
  PA_KeSMSwAcsMd8SecRwLtStLgrstUpwdDnwdPosMax_Val : Constant  Value=KeSMSwAcsMd8SecRwLtStLgrstUpwdDnwdPosMax_Val
  PA_KeSMSwAcsMd8SecRwLtStLgrstUpwdDnwdPosMin_Val : Constant  Value=KeSMSwAcsMd8SecRwLtStLgrstUpwdDnwdPosMin_Val
  PA_KeSMSwAcsMd8SecRwLtStLgrstUpwdDnwdPos_Val : Constant  Value=KeSMSwAcsMd8SecRwLtStLgrstUpwdDnwdPos_Val
  PA_KeSMSwFamilyMdSecRwLtStFrwdBkwdPosMax_Val : Constant  Value=KeSMSwFamilyMdSecRwLtStFrwdBkwdPosMax_Val
  PA_KeSMSwFamilyMdSecRwLtStFrwdBkwdPosMin_Val : Constant  Value=KeSMSwFamilyMdSecRwLtStFrwdBkwdPosMin_Val
  PA_KeSMSwFamilyMdSecRwLtStFrwdBkwdPos_Val : Constant  Value=KeSMSwFamilyMdSecRwLtStFrwdBkwdPos_Val
  PA_KeSMSwFamilyMdSecRwLtStLtwdRtwdPosMax_Val : Constant  Value=KeSMSwFamilyMdSecRwLtStLtwdRtwdPosMax_Val
  PA_KeSMSwFamilyMdSecRwLtStLtwdRtwdPosMin_Val : Constant  Value=KeSMSwFamilyMdSecRwLtStLtwdRtwdPosMin_Val
  PA_KeSMSwFamilyMdSecRwLtStLtwdRtwdPos_Val : Constant  Value=KeSMSwFamilyMdSecRwLtStLtwdRtwdPos_Val
  PA_KeSMSwFamilyRMdSecRwLtStFrwdBkwdPosMax_Val : Constant  Value=KeSMSwFamilyRMdSecRwLtStFrwdBkwdPosMax_Val
  PA_KeSMSwFamilyRMdSecRwLtStFrwdBkwdPosMin_Val : Constant  Value=KeSMSwFamilyRMdSecRwLtStFrwdBkwdPosMin_Val
  PA_KeSMSwFamilyRMdSecRwLtStFrwdBkwdPos_Val : Constant  Value=KeSMSwFamilyRMdSecRwLtStFrwdBkwdPos_Val
  PA_KeSMSwFamilyRMdSecRwLtStLtwdRtwdPosMax_Val : Constant  Value=KeSMSwFamilyRMdSecRwLtStLtwdRtwdPosMax_Val
  PA_KeSMSwFamilyRMdSecRwLtStLtwdRtwdPosMin_Val : Constant  Value=KeSMSwFamilyRMdSecRwLtStLtwdRtwdPosMin_Val
  PA_KeSMSwFamilyRMdSecRwLtStLtwdRtwdPos_Val : Constant  Value=KeSMSwFamilyRMdSecRwLtStLtwdRtwdPos_Val
  PA_KeSMSwIntimacyMdSecRwLtStLtwdRtwdPosMax_Val : Constant  Value=KeSMSwIntimacyMdSecRwLtStLtwdRtwdPosMax_Val
  PA_KeSMSwIntimacyMdSecRwLtStLtwdRtwdPosMin_Val : Constant  Value=KeSMSwIntimacyMdSecRwLtStLtwdRtwdPosMin_Val
  PA_KeSMSwIntimacyMdSecRwLtStLtwdRtwdPos_Val : Constant  Value=KeSMSwIntimacyMdSecRwLtStLtwdRtwdPos_Val
  PA_KeSMSwIntimacyRMdSecRwLtStLtwdRtwdPosMax_Val : Constant  Value=KeSMSwIntimacyRMdSecRwLtStLtwdRtwdPosMax_Val
  PA_KeSMSwIntimacyRMdSecRwLtStLtwdRtwdPosMin_Val : Constant  Value=KeSMSwIntimacyRMdSecRwLtStLtwdRtwdPosMin_Val
  PA_KeSMSwIntimacyRMdSecRwLtStLtwdRtwdPos_Val : Constant  Value=KeSMSwIntimacyRMdSecRwLtStLtwdRtwdPos_Val
  PA_KeSMSwMd27SecRwLtStBkReclnUpwdDnwdPos1Max_Val : Constant  Value=KeSMSwMd27SecRwLtStBkReclnUpwdDnwdPos1Max_Val
  PA_KeSMSwMd27SecRwLtStBkReclnUpwdDnwdPos1Min_Val : Constant  Value=KeSMSwMd27SecRwLtStBkReclnUpwdDnwdPos1Min_Val
  PA_KeSMSwMd27SecRwLtStBkReclnUpwdDnwdPos1_Val : Constant  Value=KeSMSwMd27SecRwLtStBkReclnUpwdDnwdPos1_Val
  PA_KeSMSwMd27SecRwLtStBkReclnUpwdDnwdPos2Max_Val : Constant  Value=KeSMSwMd27SecRwLtStBkReclnUpwdDnwdPos2Max_Val
  PA_KeSMSwMd27SecRwLtStBkReclnUpwdDnwdPos2Min_Val : Constant  Value=KeSMSwMd27SecRwLtStBkReclnUpwdDnwdPos2Min_Val
  PA_KeSMSwMd27SecRwLtStBkReclnUpwdDnwdPos2_Val : Constant  Value=KeSMSwMd27SecRwLtStBkReclnUpwdDnwdPos2_Val
  PA_KeSMSwMd27SecRwLtStBkReclnUpwdDnwdPos3Max_Val : Constant  Value=KeSMSwMd27SecRwLtStBkReclnUpwdDnwdPos3Max_Val
  PA_KeSMSwMd27SecRwLtStBkReclnUpwdDnwdPos3Min_Val : Constant  Value=KeSMSwMd27SecRwLtStBkReclnUpwdDnwdPos3Min_Val
  PA_KeSMSwMd27SecRwLtStBkReclnUpwdDnwdPos3_Val : Constant  Value=KeSMSwMd27SecRwLtStBkReclnUpwdDnwdPos3_Val
  PA_KeSMSwRecoveryMdSecRwLtStBkReclnUpwdDnwdPosMax_Val : Constant  Value=KeSMSwRecoveryMdSecRwLtStBkReclnUpwdDnwdPosMax_Val
  PA_KeSMSwRecoveryMdSecRwLtStBkReclnUpwdDnwdPosMin_Val : Constant  Value=KeSMSwRecoveryMdSecRwLtStBkReclnUpwdDnwdPosMin_Val
  PA_KeSMSwRecoveryMdSecRwLtStBkReclnUpwdDnwdPos_Val : Constant  Value=KeSMSwRecoveryMdSecRwLtStBkReclnUpwdDnwdPos_Val
  PA_KeSMSwRecoveryMdSecRwLtStLgrstInwdOtwdPosMax_Val : Constant  Value=KeSMSwRecoveryMdSecRwLtStLgrstInwdOtwdPosMax_Val
  PA_KeSMSwRecoveryMdSecRwLtStLgrstInwdOtwdPosMin_Val : Constant  Value=KeSMSwRecoveryMdSecRwLtStLgrstInwdOtwdPosMin_Val
  PA_KeSMSwRecoveryMdSecRwLtStLgrstInwdOtwdPos_Val : Constant  Value=KeSMSwRecoveryMdSecRwLtStLgrstInwdOtwdPos_Val
  PA_KeSMSwRecoveryMdSecRwLtStLgrstUpwdDnwdPosMax_Val : Constant  Value=KeSMSwRecoveryMdSecRwLtStLgrstUpwdDnwdPosMax_Val
  PA_KeSMSwRecoveryMdSecRwLtStLgrstUpwdDnwdPosMin_Val : Constant  Value=KeSMSwRecoveryMdSecRwLtStLgrstUpwdDnwdPosMin_Val
  PA_KeSMSwRecoveryMdSecRwLtStLgrstUpwdDnwdPos_Val : Constant  Value=KeSMSwRecoveryMdSecRwLtStLgrstUpwdDnwdPos_Val
  PA_KeSMSwSecRwLtStBkReclnEnTrigBitMask6s_Val : Constant  Value=KeSMSwSecRwLtStBkReclnEnTrigBitMask6s_Val
  PA_KeSMSwSecRwLtStBkReclnEnTrigBitMask_Val : Constant  Value=KeSMSwSecRwLtStBkReclnEnTrigBitMask_Val
  PA_KeSMSwSecRwLtStFwdBkwdEnTrigBitMask6s_Val : Constant  Value=KeSMSwSecRwLtStFwdBkwdEnTrigBitMask6s_Val
  PA_KeSMSwSecRwLtStFwdBkwdEnTrigBitMask_Val : Constant  Value=KeSMSwSecRwLtStFwdBkwdEnTrigBitMask_Val
  PA_KeSMSwSecRwLtStLgrstInwdOtwdEnTrigBitMask6s_Val : Constant  Value=KeSMSwSecRwLtStLgrstInwdOtwdEnTrigBitMask6s_Val
  PA_KeSMSwSecRwLtStLgrstInwdOtwdEnTrigBitMask_Val : Constant  Value=KeSMSwSecRwLtStLgrstInwdOtwdEnTrigBitMask_Val
  PA_KeSMSwSecRwLtStLgrstUpwdDnwdEnTrigBitMask6s_Val : Constant  Value=KeSMSwSecRwLtStLgrstUpwdDnwdEnTrigBitMask6s_Val
  PA_KeSMSwSecRwLtStLgrstUpwdDnwdEnTrigBitMask_Val : Constant  Value=KeSMSwSecRwLtStLgrstUpwdDnwdEnTrigBitMask_Val
  PA_KeSMSwVIPMdSecRwLtStLgrstInwdOtwdPosMax_Val : Constant  Value=KeSMSwVIPMdSecRwLtStLgrstInwdOtwdPosMax_Val
  PA_KeSMSwVIPMdSecRwLtStLgrstInwdOtwdPosMin_Val : Constant  Value=KeSMSwVIPMdSecRwLtStLgrstInwdOtwdPosMin_Val
  PA_KeSMSwVIPMdSecRwLtStLgrstInwdOtwdPos_Val : Constant  Value=KeSMSwVIPMdSecRwLtStLgrstInwdOtwdPos_Val
  PA_KeSMSwVIPSecRwLtStBkReclnUpwdDnwdPosMax_Val : Constant  Value=KeSMSwVIPSecRwLtStBkReclnUpwdDnwdPosMax_Val
  PA_KeSMSwVIPSecRwLtStBkReclnUpwdDnwdPosMin_Val : Constant  Value=KeSMSwVIPSecRwLtStBkReclnUpwdDnwdPosMin_Val
  PA_KeSMSwVIPSecRwLtStBkReclnUpwdDnwdPos_Val : Constant  Value=KeSMSwVIPSecRwLtStBkReclnUpwdDnwdPos_Val
  PA_KeSMSwVIPSecRwLtStFrwdBkwdPosMax_Val : Constant  Value=KeSMSwVIPSecRwLtStFrwdBkwdPosMax_Val
  PA_KeSMSwVIPSecRwLtStFrwdBkwdPosMin_Val : Constant  Value=KeSMSwVIPSecRwLtStFrwdBkwdPosMin_Val
  PA_KeSMSwVIPSecRwLtStFrwdBkwdPos_Val : Constant  Value=KeSMSwVIPSecRwLtStFrwdBkwdPos_Val
  PA_KeSMSwVIPSecRwLtStLgrstUpwdPosMax_Val : Constant  Value=KeSMSwVIPSecRwLtStLgrstUpwdPosMax_Val
  PA_KeSMSwVIPSecRwLtStLgrstUpwdPosMin_Val : Constant  Value=KeSMSwVIPSecRwLtStLgrstUpwdPosMin_Val
  PA_KeSMSwVIPSecRwLtStLgrstUpwdPos_Val : Constant  Value=KeSMSwVIPSecRwLtStLgrstUpwdPos_Val
  PA_KeSMSwVIPSecRwLtStLtwdRtwdPosMax_Val : Constant  Value=KeSMSwVIPSecRwLtStLtwdRtwdPosMax_Val
  PA_KeSMSwVIPSecRwLtStLtwdRtwdPosMin_Val : Constant  Value=KeSMSwVIPSecRwLtStLtwdRtwdPosMin_Val
  PA_KeSMSwVIPSecRwLtStLtwdRtwdPos_Val : Constant  Value=KeSMSwVIPSecRwLtStLtwdRtwdPos_Val
  SecRwLtStZeroTrgtPosSelc_Cal_sys : Subsystem
  Terminator_{1..539} (539 alike) : Terminator
  ComfortMdR2LZeroTrgtPosCalib_TrgtPosArray_write : Outport  VectorParamsAs1DForOutWhenUnconnected=off
  EZEMdR2LZeroTrgtPosCalib_TrgtPosArray_write : Outport  Port=2  VectorParamsAs1DForOutWhenUnconnected=off
  Md56R2LZeroTrgtPosCalib_TrgtPosArray_write : Outport  Port=3  VectorParamsAs1DForOutWhenUnconnected=off
  Md8R2LZeroTrgtPosCalib_TrgtPosArray_write : Outport  Port=4  VectorParamsAs1DForOutWhenUnconnected=off
  SecRwLtStZeroEnTrigBitMask_Val_write : Outport  Port=5  VectorParamsAs1DForOutWhenUnconnected=off
  SecRwLtStZeroTrgtPosCalibArray32_TrgtPosArray32_write : Outport  Port=6  VectorParamsAs1DForOutWhenUnconnected=off
  VIPLExitMdR2LZeroTrgtPosCalib_TrgtPosArray_write : Outport  Port=7  VectorParamsAs1DForOutWhenUnconnected=off
  VIPLMdR2LZeroTrgtPosCalib_TrgtPosArray_write : Outport  Port=8  VectorParamsAs1DForOutWhenUnconnected=off
  wires:
  SecRwLtStZeroTrgtPosSelc_Cal_sys/1(ComfortMdR2LZeroTrgtPosCalib_TrgtPosArray_write) -> ComfortMdR2LZeroTrgtPosCalib_TrgtPosArray_write/1
  SecRwLtStZeroTrgtPosSelc_Cal_sys/2(EZEMdR2LZeroTrgtPosCalib_TrgtPosArray_write) -> EZEMdR2LZeroTrgtPosCalib_TrgtPosArray_write/1
  SecRwLtStZeroTrgtPosSelc_Cal_sys/3(SecRwLtStZeroTrgtPosCalibArray32_TrgtPosArray32_write) -> SecRwLtStZeroTrgtPosCalibArray32_TrgtPosArray32_write/1
  SecRwLtStZeroTrgtPosSelc_Cal_sys/4(VIPLMdR2LZeroTrgtPosCalib_TrgtPosArray_write) -> VIPLMdR2LZeroTrgtPosCalib_TrgtPosArray_write/1
  SecRwLtStZeroTrgtPosSelc_Cal_sys/5(VIPLExitMdR2LZeroTrgtPosCalib_TrgtPosArray_write) -> VIPLExitMdR2LZeroTrgtPosCalib_TrgtPosArray_write/1
  SecRwLtStZeroTrgtPosSelc_Cal_sys/6(SecRwLtStZeroEnTrigBitMask_Val_write) -> SecRwLtStZeroEnTrigBitMask_Val_write/1
  SecRwLtStZeroTrgtPosSelc_Cal_sys/7(Md8R2LZeroTrgtPosCalib_TrgtPosArray_write) -> Md8R2LZeroTrgtPosCalib_TrgtPosArray_write/1
  SecRwLtStZeroTrgtPosSelc_Cal_sys/8(Md56R2LZeroTrgtPosCalib_TrgtPosArray_write) -> Md56R2LZeroTrgtPosCalib_TrgtPosArray_write/1
  StNumFlg_Is4s_read/1 -> SecRwLtStZeroTrgtPosSelc_Cal_sys/1(StNumFlg_Is4s_read)
  StNumFlg_Is6s_read/1 -> SecRwLtStZeroTrgtPosSelc_Cal_sys/2(StNumFlg_Is6s_read)
  StNumFlg_Is6s7s_read/1 -> SecRwLtStZeroTrgtPosSelc_Cal_sys/3(StNumFlg_Is6s7s_read)
  StNumFlg_Is7s_read/1 -> SecRwLtStZeroTrgtPosSelc_Cal_sys/4(StNumFlg_Is7s_read)
  Md61SecRwRtStCushFrntTrgtPosCalib_TrgtPosArray_read/1 -> SecRwLtStZeroTrgtPosSelc_Cal_sys/5(Md61SecRwRtStCushFrntTrgtPosCalib_TrgtPosArray_read)
  Md62SecRwLtStCushFrntTrgtPosCalib_TrgtPosArray_read/1 -> SecRwLtStZeroTrgtPosSelc_Cal_sys/6(Md62SecRwLtStCushFrntTrgtPosCalib_TrgtPosArray_read)
  PA_KeSMSw4SAcsMd21SecRwLtStBkReclnUpwdDnwdPosMax_Val/1 -> Terminator_1/1
  PA_KeSMSw4SAcsMd21SecRwLtStBkReclnUpwdDnwdPosMin_Val/1 -> Terminator_2/1
  PA_KeSMSw4SAcsMd21SecRwLtStBkReclnUpwdDnwdPos_Val/1 -> Terminator_3/1
  PA_KeSMSw4SAcsMd21SecRwLtStFrwdBkwdPosMax_Val/1 -> Terminator_4/1
  PA_KeSMSw4SAcsMd21SecRwLtStFrwdBkwdPosMin_Val/1 -> Terminator_5/1
  PA_KeSMSw4SAcsMd21SecRwLtStFrwdBkwdPos_Val/1 -> Terminator_6/1
  PA_KeSMSw4SAcsMd21SecRwLtStHdrstFrwdBkwdPosMax_Val/1 -> Terminator_7/1
  PA_KeSMSw4SAcsMd21SecRwLtStHdrstFrwdBkwdPosMin_Val/1 -> Terminator_8/1
  PA_KeSMSw4SAcsMd21SecRwLtStHdrstFrwdBkwdPos_Val/1 -> Terminator_9/1
  PA_KeSMSw4SAcsMd21SecRwLtStHdrstUpwdDnwdPosMax_Val/1 -> Terminator_10/1
  PA_KeSMSw4SAcsMd21SecRwLtStHdrstUpwdDnwdPosMin_Val/1 -> Terminator_11/1
  PA_KeSMSw4SAcsMd21SecRwLtStHdrstUpwdDnwdPos_Val/1 -> Terminator_12/1
  PA_KeSMSw4SAcsMd22SecRwLtStBkReclnUpwdDnwdPos1_Val/1 -> Terminator_13/1
  PA_KeSMSw4SAcsMd22SecRwLtStBkReclnUpwdDnwdPos2Max_Val/1 -> Terminator_14/1
  PA_KeSMSw4SAcsMd22SecRwLtStBkReclnUpwdDnwdPos2Min_Val/1 -> Terminator_15/1
  PA_KeSMSw4SAcsMd22SecRwLtStBkReclnUpwdDnwdPos2_Val/1 -> Terminator_16/1
  PA_KeSMSw4SAcsMd22SecRwLtStBkReclnUpwdDnwdPosMax_Val/1 -> Terminator_17/1
  PA_KeSMSw4SAcsMd22SecRwLtStBkReclnUpwdDnwdPosMin_Val/1 -> Terminator_18/1
  PA_KeSMSw4SAcsMd22SecRwLtStFrwdBkwdPosMax_Val/1 -> Terminator_19/1
  PA_KeSMSw4SAcsMd22SecRwLtStFrwdBkwdPosMin_Val/1 -> Terminator_20/1
  PA_KeSMSw4SAcsMd22SecRwLtStFrwdBkwdPos_Val/1 -> Terminator_21/1
  PA_KeSMSw4SAcsMd22SecRwLtStFtrstUpwdDnwdPosMax_Val/1 -> Terminator_22/1
  PA_KeSMSw4SAcsMd22SecRwLtStFtrstUpwdDnwdPosMin_Val/1 -> Terminator_23/1
  PA_KeSMSw4SAcsMd22SecRwLtStFtrstUpwdDnwdPos_Val/1 -> Terminator_24/1
  PA_KeSMSw4SAcsMd22SecRwLtStHdrstFrwdBkwdPosMax_Val/1 -> Terminator_25/1
  PA_KeSMSw4SAcsMd22SecRwLtStHdrstFrwdBkwdPosMin_Val/1 -> Terminator_26/1
  PA_KeSMSw4SAcsMd22SecRwLtStHdrstFrwdBkwdPos_Val/1 -> Terminator_27/1
  PA_KeSMSw4SAcsMd22SecRwLtStHdrstUpwdDnwdPosMax_Val/1 -> Terminator_28/1
  PA_KeSMSw4SAcsMd22SecRwLtStHdrstUpwdDnwdPosMin_Val/1 -> Terminator_29/1
  PA_KeSMSw4SAcsMd22SecRwLtStHdrstUpwdDnwdPos_Val/1 -> Terminator_30/1
  PA_KeSMSw4SAcsMd22SecRwLtStLegrstOtwdInwdPosMax_Val/1 -> Terminator_31/1
  PA_KeSMSw4SAcsMd22SecRwLtStLegrstOtwdInwdPosMin_Val/1 -> Terminator_32/1
  PA_KeSMSw4SAcsMd22SecRwLtStLegrstOtwdInwdPos_Val/1 -> Terminator_33/1
  PA_KeSMSw4SAcsMd22SecRwLtStLegrstUpwdDnwdPosMax_Val/1 -> Terminator_34/1
  PA_KeSMSw4SAcsMd22SecRwLtStLegrstUpwdDnwdPosMin_Val/1 -> Terminator_35/1
  PA_KeSMSw4SAcsMd22SecRwLtStLegrstUpwdDnwdPos_Val/1 -> Terminator_36/1
  PA_KeSMSw4SAcsMd25SecRwLtStBkReclnUpwdDnwdPosMax_Val/1 -> Terminator_37/1
  PA_KeSMSw4SAcsMd25SecRwLtStBkReclnUpwdDnwdPosMin_Val/1 -> Terminator_38/1
  PA_KeSMSw4SAcsMd25SecRwLtStBkReclnUpwdDnwdPos_Val/1 -> Terminator_39/1
  PA_KeSMSw4SAcsMd25SecRwLtStFrwdBkwdPosMax_Val/1 -> Terminator_40/1
  PA_KeSMSw4SAcsMd25SecRwLtStFrwdBkwdPosMin_Val/1 -> Terminator_41/1
  PA_KeSMSw4SAcsMd25SecRwLtStFrwdBkwdPos_Val/1 -> Terminator_42/1
  PA_KeSMSw4SAcsMd25SecRwLtStHdrstFrwdBkwdPosMax_Val/1 -> Terminator_43/1
  PA_KeSMSw4SAcsMd25SecRwLtStHdrstFrwdBkwdPosMin_Val/1 -> Terminator_44/1
  PA_KeSMSw4SAcsMd25SecRwLtStHdrstFrwdBkwdPos_Val/1 -> Terminator_45/1
  PA_KeSMSw4SAcsMd25SecRwLtStHdrstUpwdDnwdPosMax_Val/1 -> Terminator_46/1
  PA_KeSMSw4SAcsMd25SecRwLtStHdrstUpwdDnwdPosMin_Val/1 -> Terminator_47/1
  PA_KeSMSw4SAcsMd25SecRwLtStHdrstUpwdDnwdPos_Val/1 -> Terminator_48/1
  PA_KeSMSw4SAcsMd26SecRwLtStBkReclnUpwdDnwdPosMax_Val/1 -> Terminator_49/1
  PA_KeSMSw4SAcsMd26SecRwLtStBkReclnUpwdDnwdPosMin_Val/1 -> Terminator_50/1
  PA_KeSMSw4SAcsMd26SecRwLtStBkReclnUpwdDnwdPos_Val/1 -> Terminator_51/1
  PA_KeSMSw4SAcsMd26SecRwLtStFrwdBkwdPosMax_Val/1 -> Terminator_52/1
  PA_KeSMSw4SAcsMd26SecRwLtStFrwdBkwdPosMin_Val/1 -> Terminator_53/1
  PA_KeSMSw4SAcsMd26SecRwLtStFrwdBkwdPos_Val/1 -> Terminator_54/1
  PA_KeSMSw4SAcsMd26SecRwLtStFtrstUpwdDnwdPosMax_Val/1 -> Terminator_55/1
  PA_KeSMSw4SAcsMd26SecRwLtStFtrstUpwdDnwdPosMin_Val/1 -> Terminator_56/1
  PA_KeSMSw4SAcsMd26SecRwLtStFtrstUpwdDnwdPos_Val/1 -> Terminator_57/1
  PA_KeSMSw4SAcsMd26SecRwLtStHdrstFrwdBkwdPosMax_Val/1 -> Terminator_58/1
  PA_KeSMSw4SAcsMd26SecRwLtStHdrstFrwdBkwdPosMin_Val/1 -> Terminator_59/1
  PA_KeSMSw4SAcsMd26SecRwLtStHdrstFrwdBkwdPos_Val/1 -> Terminator_60/1
  PA_KeSMSw4SAcsMd26SecRwLtStHdrstUpwdDnwdPosMax_Val/1 -> Terminator_61/1
  PA_KeSMSw4SAcsMd26SecRwLtStHdrstUpwdDnwdPosMin_Val/1 -> Terminator_62/1
  PA_KeSMSw4SAcsMd26SecRwLtStHdrstUpwdDnwdPos_Val/1 -> Terminator_63/1
  PA_KeSMSw4SAcsMd26SecRwLtStLegrstOtwdInwdPosMax_Val/1 -> Terminator_64/1
  PA_KeSMSw4SAcsMd26SecRwLtStLegrstOtwdInwdPosMin_Val/1 -> Terminator_65/1
  PA_KeSMSw4SAcsMd26SecRwLtStLegrstOtwdInwdPos_Val/1 -> Terminator_66/1
  PA_KeSMSw4SAcsMd26SecRwLtStLegrstUpwdDnwdPosMax_Val/1 -> Terminator_67/1
  PA_KeSMSw4SAcsMd26SecRwLtStLegrstUpwdDnwdPosMin_Val/1 -> Terminator_68/1
  PA_KeSMSw4SAcsMd26SecRwLtStLegrstUpwdDnwdPos_Val/1 -> Terminator_69/1
  PA_KeSMSw4SLegrstCloseMdSecRwLtStFtrstUpwdDnwdPosMax_Val/1 -> Terminator_70/1
  PA_KeSMSw4SLegrstCloseMdSecRwLtStFtrstUpwdDnwdPosMin_Val/1 -> Terminator_71/1
  PA_KeSMSw4SLegrstCloseMdSecRwLtStFtrstUpwdDnwdPos_Val/1 -> Terminator_72/1
  PA_KeSMSw4SLegrstCloseMdSecRwLtStLgrstOtwdInwdPosMax_Val/1 -> Terminator_73/1
  PA_KeSMSw4SLegrstCloseMdSecRwLtStLgrstOtwdInwdPosMin_Val/1 -> Terminator_74/1
  PA_KeSMSw4SLegrstCloseMdSecRwLtStLgrstOtwdInwdPos_Val/1 -> Terminator_75/1
  PA_KeSMSw4SLegrstCloseMdSecRwLtStLgrstUpwdDnwdPosMax_Val/1 -> Terminator_76/1
  PA_KeSMSw4SLegrstCloseMdSecRwLtStLgrstUpwdDnwdPosMin_Val/1 -> Terminator_77/1
  PA_KeSMSw4SLegrstCloseMdSecRwLtStLgrstUpwdDnwdPos_Val/1 -> Terminator_78/1
  PA_KeSMSw4SLegrstOpenMdSecRwLtStFrwdBkwdPosMax_Val/1 -> Terminator_79/1
  PA_KeSMSw4SLegrstOpenMdSecRwLtStFrwdBkwdPosMin_Val/1 -> Terminator_80/1
  PA_KeSMSw4SLegrstOpenMdSecRwLtStFrwdBkwdPos_Val/1 -> Terminator_81/1
  PA_KeSMSw4SLegrstOpenMdSecRwLtStFtrstUpwdDnwdPosMax_Val/1 -> Terminator_82/1
  PA_KeSMSw4SLegrstOpenMdSecRwLtStFtrstUpwdDnwdPosMin_Val/1 -> Terminator_83/1
  PA_KeSMSw4SLegrstOpenMdSecRwLtStFtrstUpwdDnwdPos_Val/1 -> Terminator_84/1
  PA_KeSMSw4SLegrstOpenMdSecRwLtStLgrstOtwdInwdPosMax_Val/1 -> Terminator_85/1
  PA_KeSMSw4SLegrstOpenMdSecRwLtStLgrstOtwdInwdPosMin_Val/1 -> Terminator_86/1
  PA_KeSMSw4SLegrstOpenMdSecRwLtStLgrstOtwdInwdPos_Val/1 -> Terminator_87/1
  PA_KeSMSw4SLegrstOpenMdSecRwLtStLgrstUpwdDnwdPosMax_Val/1 -> Terminator_88/1
  PA_KeSMSw4SLegrstOpenMdSecRwLtStLgrstUpwdDnwdPosMin_Val/1 -> Terminator_89/1
  PA_KeSMSw4SLegrstOpenMdSecRwLtStLgrstUpwdDnwdPos_Val/1 -> Terminator_90/1
  PA_KeSMSw4SLyingMDSecRwLtStFrwdBkwdPosMax_Val/1 -> Terminator_91/1
  PA_KeSMSw4SLyingMDSecRwLtStFrwdBkwdPosMin_Val/1 -> Terminator_92/1
  PA_KeSMSw4SLyingMDSecRwLtStFrwdBkwdPos_Val/1 -> Terminator_93/1
  PA_KeSMSw4SVIPMDSecRwLtStFrwdBkwdPosMax_Val/1 -> Terminator_94/1
  PA_KeSMSw4SVIPMDSecRwLtStFrwdBkwdPosMin_Val/1 -> Terminator_95/1
  PA_KeSMSw4SVIPMDSecRwLtStFrwdBkwdPos_Val/1 -> Terminator_96/1
  PA_KeSMSw4sLyingMDSecRwLtStBkReclnUpwdDnwdPosMax_Val/1 -> Terminator_97/1
  PA_KeSMSw4sLyingMDSecRwLtStBkReclnUpwdDnwdPosMin_Val/1 -> Terminator_98/1
  PA_KeSMSw4sLyingMDSecRwLtStBkReclnUpwdDnwdPos_Val/1 -> Terminator_99/1
  PA_KeSMSw4sLyingMDSecRwLtStFtrstUpwdDnwdPosMax_Val/1 -> Terminator_100/1
  PA_KeSMSw4sLyingMDSecRwLtStFtrstUpwdDnwdPosMin_Val/1 -> Terminator_101/1
  PA_KeSMSw4sLyingMDSecRwLtStFtrstUpwdDnwdPos_Val/1 -> Terminator_102/1
  PA_KeSMSw4sLyingMDSecRwLtStHdrstFrwdBkwdnwdPosMax_160_Val/1 -> Terminator_103/1
  PA_KeSMSw4sLyingMDSecRwLtStHdrstFrwdBkwdnwdPosMax_165_Val/1 -> Terminator_104/1
  PA_KeSMSw4sLyingMDSecRwLtStHdrstFrwdBkwdnwdPosMax_170_Val/1 -> Terminator_105/1
  PA_KeSMSw4sLyingMDSecRwLtStHdrstFrwdBkwdnwdPosMax_175_Val/1 -> Terminator_106/1
  PA_KeSMSw4sLyingMDSecRwLtStHdrstFrwdBkwdnwdPosMax_180_Val/1 -> Terminator_107/1
  PA_KeSMSw4sLyingMDSecRwLtStHdrstFrwdBkwdnwdPosMax_Below160_Val/1 -> Terminator_108/1
  PA_KeSMSw4sLyingMDSecRwLtStHdrstFrwdBkwdnwdPosMax_Over180_Val/1 -> Terminator_109/1
  PA_KeSMSw4sLyingMDSecRwLtStHdrstFrwdBkwdnwdPosMin_160_Val/1 -> Terminator_110/1
  PA_KeSMSw4sLyingMDSecRwLtStHdrstFrwdBkwdnwdPosMin_165_Val/1 -> Terminator_111/1
  PA_KeSMSw4sLyingMDSecRwLtStHdrstFrwdBkwdnwdPosMin_170_Val/1 -> Terminator_112/1
  PA_KeSMSw4sLyingMDSecRwLtStHdrstFrwdBkwdnwdPosMin_175_Val/1 -> Terminator_113/1
  PA_KeSMSw4sLyingMDSecRwLtStHdrstFrwdBkwdnwdPosMin_180_Val/1 -> Terminator_114/1
  PA_KeSMSw4sLyingMDSecRwLtStHdrstFrwdBkwdnwdPosMin_Below160_Val/1 -> Terminator_115/1
  PA_KeSMSw4sLyingMDSecRwLtStHdrstFrwdBkwdnwdPosMin_Over180_Val/1 -> Terminator_116/1
  PA_KeSMSw4sLyingMDSecRwLtStHdrstFrwdBkwdnwdPos_160_Val/1 -> Terminator_117/1
  PA_KeSMSw4sLyingMDSecRwLtStHdrstFrwdBkwdnwdPos_165_Val/1 -> Terminator_118/1
  PA_KeSMSw4sLyingMDSecRwLtStHdrstFrwdBkwdnwdPos_170_Val/1 -> Terminator_119/1
  PA_KeSMSw4sLyingMDSecRwLtStHdrstFrwdBkwdnwdPos_175_Val/1 -> Terminator_120/1
  PA_KeSMSw4sLyingMDSecRwLtStHdrstFrwdBkwdnwdPos_180_Val/1 -> Terminator_121/1
  PA_KeSMSw4sLyingMDSecRwLtStHdrstFrwdBkwdnwdPos_Below160_Val/1 -> Terminator_122/1
  PA_KeSMSw4sLyingMDSecRwLtStHdrstFrwdBkwdnwdPos_Over180_Val/1 -> Terminator_123/1
  PA_KeSMSw4sLyingMDSecRwLtStHdrstUpwdDnwdPosMax_160_Val/1 -> Terminator_124/1
  PA_KeSMSw4sLyingMDSecRwLtStHdrstUpwdDnwdPosMax_165_Val/1 -> Terminator_125/1
  PA_KeSMSw4sLyingMDSecRwLtStHdrstUpwdDnwdPosMax_170_Val/1 -> Terminator_126/1
  PA_KeSMSw4sLyingMDSecRwLtStHdrstUpwdDnwdPosMax_175_Val/1 -> Terminator_127/1
  PA_KeSMSw4sLyingMDSecRwLtStHdrstUpwdDnwdPosMax_180_Val/1 -> Terminator_128/1
  PA_KeSMSw4sLyingMDSecRwLtStHdrstUpwdDnwdPosMax_Below160_Val/1 -> Terminator_129/1
  PA_KeSMSw4sLyingMDSecRwLtStHdrstUpwdDnwdPosMax_Over180_Val/1 -> Terminator_130/1
  PA_KeSMSw4sLyingMDSecRwLtStHdrstUpwdDnwdPosMin_160_Val/1 -> Terminator_131/1
  PA_KeSMSw4sLyingMDSecRwLtStHdrstUpwdDnwdPosMin_165_Val/1 -> Terminator_132/1
  PA_KeSMSw4sLyingMDSecRwLtStHdrstUpwdDnwdPosMin_170_Val/1 -> Terminator_133/1
  PA_KeSMSw4sLyingMDSecRwLtStHdrstUpwdDnwdPosMin_175_Val/1 -> Terminator_134/1
  PA_KeSMSw4sLyingMDSecRwLtStHdrstUpwdDnwdPosMin_180_Val/1 -> Terminator_135/1
  PA_KeSMSw4sLyingMDSecRwLtStHdrstUpwdDnwdPosMin_Below160_Val/1 -> Terminator_136/1
  PA_KeSMSw4sLyingMDSecRwLtStHdrstUpwdDnwdPosMin_Over180_Val/1 -> Terminator_137/1
  PA_KeSMSw4sLyingMDSecRwLtStHdrstUpwdDnwdPos_160_Val/1 -> Terminator_138/1
  PA_KeSMSw4sLyingMDSecRwLtStHdrstUpwdDnwdPos_165_Val/1 -> Terminator_139/1
  PA_KeSMSw4sLyingMDSecRwLtStHdrstUpwdDnwdPos_170_Val/1 -> Terminator_140/1
  PA_KeSMSw4sLyingMDSecRwLtStHdrstUpwdDnwdPos_175_Val/1 -> Terminator_141/1
  PA_KeSMSw4sLyingMDSecRwLtStHdrstUpwdDnwdPos_180_Val/1 -> Terminator_142/1
  PA_KeSMSw4sLyingMDSecRwLtStHdrstUpwdDnwdPos_Below160_Val/1 -> Terminator_143/1
  PA_KeSMSw4sLyingMDSecRwLtStHdrstUpwdDnwdPos_Over180_Val/1 -> Terminator_144/1
  PA_KeSMSw4sLyingMDSecRwLtStLgrstOtwdInwdPosMax_160_Val/1 -> Terminator_145/1
  PA_KeSMSw4sLyingMDSecRwLtStLgrstOtwdInwdPosMax_165_Val/1 -> Terminator_146/1
  PA_KeSMSw4sLyingMDSecRwLtStLgrstOtwdInwdPosMax_170_Val/1 -> Terminator_147/1
  PA_KeSMSw4sLyingMDSecRwLtStLgrstOtwdInwdPosMax_175_Val/1 -> Terminator_148/1
  PA_KeSMSw4sLyingMDSecRwLtStLgrstOtwdInwdPosMax_180_Val/1 -> Terminator_149/1
  PA_KeSMSw4sLyingMDSecRwLtStLgrstOtwdInwdPosMax_Below160_Val/1 -> Terminator_150/1
  PA_KeSMSw4sLyingMDSecRwLtStLgrstOtwdInwdPosMax_Over180_Val/1 -> Terminator_151/1
  PA_KeSMSw4sLyingMDSecRwLtStLgrstOtwdInwdPosMin_160_Val/1 -> Terminator_152/1
  PA_KeSMSw4sLyingMDSecRwLtStLgrstOtwdInwdPosMin_165_Val/1 -> Terminator_153/1
  PA_KeSMSw4sLyingMDSecRwLtStLgrstOtwdInwdPosMin_170_Val/1 -> Terminator_154/1
  PA_KeSMSw4sLyingMDSecRwLtStLgrstOtwdInwdPosMin_175_Val/1 -> Terminator_155/1
  PA_KeSMSw4sLyingMDSecRwLtStLgrstOtwdInwdPosMin_180_Val/1 -> Terminator_156/1
  PA_KeSMSw4sLyingMDSecRwLtStLgrstOtwdInwdPosMin_Below160_Val/1 -> Terminator_157/1
  PA_KeSMSw4sLyingMDSecRwLtStLgrstOtwdInwdPosMin_Over180_Val/1 -> Terminator_158/1
  PA_KeSMSw4sLyingMDSecRwLtStLgrstOtwdInwdPos_160_Val/1 -> Terminator_159/1
  PA_KeSMSw4sLyingMDSecRwLtStLgrstOtwdInwdPos_165_Val/1 -> Terminator_160/1
  PA_KeSMSw4sLyingMDSecRwLtStLgrstOtwdInwdPos_170_Val/1 -> Terminator_161/1
  PA_KeSMSw4sLyingMDSecRwLtStLgrstOtwdInwdPos_175_Val/1 -> Terminator_162/1
  PA_KeSMSw4sLyingMDSecRwLtStLgrstOtwdInwdPos_180_Val/1 -> Terminator_163/1
  PA_KeSMSw4sLyingMDSecRwLtStLgrstOtwdInwdPos_Below160_Val/1 -> Terminator_164/1
  PA_KeSMSw4sLyingMDSecRwLtStLgrstOtwdInwdPos_Over180_Val/1 -> Terminator_165/1
  PA_KeSMSw4sLyingMDSecRwLtStLgrstUpwdDnwdPosMax_Val/1 -> Terminator_166/1
  PA_KeSMSw4sLyingMDSecRwLtStLgrstUpwdDnwdPosMin_Val/1 -> Terminator_167/1
  PA_KeSMSw4sLyingMDSecRwLtStLgrstUpwdDnwdPos_Val/1 -> Terminator_168/1
  PA_KeSMSw4sRecoveryMDSecRwLtStBkReclnUpwdDnwdPosMax_Val/1 -> Terminator_169/1
  PA_KeSMSw4sRecoveryMDSecRwLtStBkReclnUpwdDnwdPosMin_Val/1 -> Terminator_170/1
  PA_KeSMSw4sRecoveryMDSecRwLtStBkReclnUpwdDnwdPos_Val/1 -> Terminator_171/1
  PA_KeSMSw4sRecoveryMDSecRwLtStFtrstUpwdDnwdPosMax_Val/1 -> Terminator_172/1
  PA_KeSMSw4sRecoveryMDSecRwLtStFtrstUpwdDnwdPosMin_Val/1 -> Terminator_173/1
  PA_KeSMSw4sRecoveryMDSecRwLtStFtrstUpwdDnwdPos_Val/1 -> Terminator_174/1
  PA_KeSMSw4sRecoveryMDSecRwLtStHdrstFrwdBkwdPosMax_160_Val/1 -> Terminator_175/1
  PA_KeSMSw4sRecoveryMDSecRwLtStHdrstFrwdBkwdPosMax_165_Val/1 -> Terminator_176/1
  PA_KeSMSw4sRecoveryMDSecRwLtStHdrstFrwdBkwdPosMax_170_Val/1 -> Terminator_177/1
  PA_KeSMSw4sRecoveryMDSecRwLtStHdrstFrwdBkwdPosMax_175_Val/1 -> Terminator_178/1
  PA_KeSMSw4sRecoveryMDSecRwLtStHdrstFrwdBkwdPosMax_180_Val/1 -> Terminator_179/1
  PA_KeSMSw4sRecoveryMDSecRwLtStHdrstFrwdBkwdPosMax_Below160_Val/1 -> Terminator_180/1
  PA_KeSMSw4sRecoveryMDSecRwLtStHdrstFrwdBkwdPosMax_Over180_Val/1 -> Terminator_181/1
  PA_KeSMSw4sRecoveryMDSecRwLtStHdrstFrwdBkwdPosMin_160_Val/1 -> Terminator_182/1
  PA_KeSMSw4sRecoveryMDSecRwLtStHdrstFrwdBkwdPosMin_165_Val/1 -> Terminator_183/1
  PA_KeSMSw4sRecoveryMDSecRwLtStHdrstFrwdBkwdPosMin_170_Val/1 -> Terminator_184/1
  PA_KeSMSw4sRecoveryMDSecRwLtStHdrstFrwdBkwdPosMin_175_Val/1 -> Terminator_185/1
  PA_KeSMSw4sRecoveryMDSecRwLtStHdrstFrwdBkwdPosMin_180_Val/1 -> Terminator_186/1
  PA_KeSMSw4sRecoveryMDSecRwLtStHdrstFrwdBkwdPosMin_Below160_Val/1 -> Terminator_187/1
  PA_KeSMSw4sRecoveryMDSecRwLtStHdrstFrwdBkwdPosMin_Over180_Val/1 -> Terminator_188/1
  PA_KeSMSw4sRecoveryMDSecRwLtStHdrstFrwdBkwdPos_160_Val/1 -> Terminator_189/1
  PA_KeSMSw4sRecoveryMDSecRwLtStHdrstFrwdBkwdPos_165_Val/1 -> Terminator_190/1
  PA_KeSMSw4sRecoveryMDSecRwLtStHdrstFrwdBkwdPos_170_Val/1 -> Terminator_191/1
  PA_KeSMSw4sRecoveryMDSecRwLtStHdrstFrwdBkwdPos_175_Val/1 -> Terminator_192/1
  PA_KeSMSw4sRecoveryMDSecRwLtStHdrstFrwdBkwdPos_180_Val/1 -> Terminator_193/1
  PA_KeSMSw4sRecoveryMDSecRwLtStHdrstFrwdBkwdPos_Below160_Val/1 -> Terminator_194/1
  PA_KeSMSw4sRecoveryMDSecRwLtStHdrstFrwdBkwdPos_Over180_Val/1 -> Terminator_195/1
  PA_KeSMSw4sRecoveryMDSecRwLtStHdrstUpwdDnwdPosMax_160_Val/1 -> Terminator_196/1
  PA_KeSMSw4sRecoveryMDSecRwLtStHdrstUpwdDnwdPosMax_165_Val/1 -> Terminator_197/1
  PA_KeSMSw4sRecoveryMDSecRwLtStHdrstUpwdDnwdPosMax_170_Val/1 -> Terminator_198/1
  PA_KeSMSw4sRecoveryMDSecRwLtStHdrstUpwdDnwdPosMax_175_Val/1 -> Terminator_199/1
  PA_KeSMSw4sRecoveryMDSecRwLtStHdrstUpwdDnwdPosMax_180_Val/1 -> Terminator_200/1
  PA_KeSMSw4sRecoveryMDSecRwLtStHdrstUpwdDnwdPosMax_Below160_Val/1 -> Terminator_201/1
  PA_KeSMSw4sRecoveryMDSecRwLtStHdrstUpwdDnwdPosMax_Over180_Val/1 -> Terminator_202/1
  PA_KeSMSw4sRecoveryMDSecRwLtStHdrstUpwdDnwdPosMin_160_Val/1 -> Terminator_203/1
  PA_KeSMSw4sRecoveryMDSecRwLtStHdrstUpwdDnwdPosMin_165_Val/1 -> Terminator_204/1
  PA_KeSMSw4sRecoveryMDSecRwLtStHdrstUpwdDnwdPosMin_170_Val/1 -> Terminator_205/1
  PA_KeSMSw4sRecoveryMDSecRwLtStHdrstUpwdDnwdPosMin_175_Val/1 -> Terminator_206/1
  PA_KeSMSw4sRecoveryMDSecRwLtStHdrstUpwdDnwdPosMin_180_Val/1 -> Terminator_207/1
  PA_KeSMSw4sRecoveryMDSecRwLtStHdrstUpwdDnwdPosMin_Below160_Val/1 -> Terminator_208/1
  PA_KeSMSw4sRecoveryMDSecRwLtStHdrstUpwdDnwdPosMin_Over180_Val/1 -> Terminator_209/1
  PA_KeSMSw4sRecoveryMDSecRwLtStHdrstUpwdDnwdPos_160_Val/1 -> Terminator_210/1
  PA_KeSMSw4sRecoveryMDSecRwLtStHdrstUpwdDnwdPos_165_Val/1 -> Terminator_211/1
  PA_KeSMSw4sRecoveryMDSecRwLtStHdrstUpwdDnwdPos_170_Val/1 -> Terminator_212/1
  PA_KeSMSw4sRecoveryMDSecRwLtStHdrstUpwdDnwdPos_175_Val/1 -> Terminator_213/1
  PA_KeSMSw4sRecoveryMDSecRwLtStHdrstUpwdDnwdPos_180_Val/1 -> Terminator_214/1
  PA_KeSMSw4sRecoveryMDSecRwLtStHdrstUpwdDnwdPos_Below160_Val/1 -> Terminator_215/1
  PA_KeSMSw4sRecoveryMDSecRwLtStHdrstUpwdDnwdPos_Over180_Val/1 -> Terminator_216/1
  PA_KeSMSw4sRecoveryMDSecRwLtStLgrstOtwdInwdPosMax_160_Val/1 -> Terminator_217/1
  PA_KeSMSw4sRecoveryMDSecRwLtStLgrstOtwdInwdPosMax_165_Val/1 -> Terminator_218/1
  PA_KeSMSw4sRecoveryMDSecRwLtStLgrstOtwdInwdPosMax_170_Val/1 -> Terminator_219/1
  PA_KeSMSw4sRecoveryMDSecRwLtStLgrstOtwdInwdPosMax_175_Val/1 -> Terminator_220/1
  PA_KeSMSw4sRecoveryMDSecRwLtStLgrstOtwdInwdPosMax_180_Val/1 -> Terminator_221/1
  PA_KeSMSw4sRecoveryMDSecRwLtStLgrstOtwdInwdPosMax_Below160_Val/1 -> Terminator_222/1
  PA_KeSMSw4sRecoveryMDSecRwLtStLgrstOtwdInwdPosMax_Over180_Val/1 -> Terminator_223/1
  PA_KeSMSw4sRecoveryMDSecRwLtStLgrstOtwdInwdPosMin_160_Val/1 -> Terminator_224/1
  PA_KeSMSw4sRecoveryMDSecRwLtStLgrstOtwdInwdPosMin_165_Val/1 -> Terminator_225/1
  PA_KeSMSw4sRecoveryMDSecRwLtStLgrstOtwdInwdPosMin_170_Val/1 -> Terminator_226/1
  PA_KeSMSw4sRecoveryMDSecRwLtStLgrstOtwdInwdPosMin_175_Val/1 -> Terminator_227/1
  PA_KeSMSw4sRecoveryMDSecRwLtStLgrstOtwdInwdPosMin_180_Val/1 -> Terminator_228/1
  PA_KeSMSw4sRecoveryMDSecRwLtStLgrstOtwdInwdPosMin_Below160_Val/1 -> Terminator_229/1
  PA_KeSMSw4sRecoveryMDSecRwLtStLgrstOtwdInwdPosMin_Over180_Val/1 -> Terminator_230/1
  PA_KeSMSw4sRecoveryMDSecRwLtStLgrstOtwdInwdPos_160_Val/1 -> Terminator_231/1
  PA_KeSMSw4sRecoveryMDSecRwLtStLgrstOtwdInwdPos_165_Val/1 -> Terminator_232/1
  PA_KeSMSw4sRecoveryMDSecRwLtStLgrstOtwdInwdPos_170_Val/1 -> Terminator_233/1
  PA_KeSMSw4sRecoveryMDSecRwLtStLgrstOtwdInwdPos_175_Val/1 -> Terminator_234/1
  PA_KeSMSw4sRecoveryMDSecRwLtStLgrstOtwdInwdPos_180_Val/1 -> Terminator_235/1
  PA_KeSMSw4sRecoveryMDSecRwLtStLgrstOtwdInwdPos_Below160_Val/1 -> Terminator_236/1
  PA_KeSMSw4sRecoveryMDSecRwLtStLgrstOtwdInwdPos_Over180_Val/1 -> Terminator_237/1
  PA_KeSMSw4sRecoveryMDSecRwLtStLgrstUpwdDnwdPosMax_Val/1 -> Terminator_238/1
  PA_KeSMSw4sRecoveryMDSecRwLtStLgrstUpwdDnwdPosMin_Val/1 -> Terminator_239/1
  PA_KeSMSw4sRecoveryMDSecRwLtStLgrstUpwdDnwdPos_Val/1 -> Terminator_240/1
  PA_KeSMSw4sVIPMDSecRwLtStBkReclnUpwdDnwdPosMax_Val/1 -> Terminator_241/1
  PA_KeSMSw4sVIPMDSecRwLtStBkReclnUpwdDnwdPosMin_Val/1 -> Terminator_242/1
  PA_KeSMSw4sVIPMDSecRwLtStBkReclnUpwdDnwdPos_Val/1 -> Terminator_243/1
  PA_KeSMSw4sVIPMDSecRwLtStFtrstUpwdDnwdPosMax_Val/1 -> Terminator_244/1
  PA_KeSMSw4sVIPMDSecRwLtStFtrstUpwdDnwdPosMin_Val/1 -> Terminator_245/1
  PA_KeSMSw4sVIPMDSecRwLtStFtrstUpwdDnwdPos_Val/1 -> Terminator_246/1
  PA_KeSMSw4sVIPMDSecRwLtStHdrstFrwdBkwdPosMax_160_Val/1 -> Terminator_247/1
  PA_KeSMSw4sVIPMDSecRwLtStHdrstFrwdBkwdPosMax_165_Val/1 -> Terminator_248/1
  PA_KeSMSw4sVIPMDSecRwLtStHdrstFrwdBkwdPosMax_170_Val/1 -> Terminator_249/1
  PA_KeSMSw4sVIPMDSecRwLtStHdrstFrwdBkwdPosMax_175_Val/1 -> Terminator_250/1
  PA_KeSMSw4sVIPMDSecRwLtStHdrstFrwdBkwdPosMax_180_Val/1 -> Terminator_251/1
  PA_KeSMSw4sVIPMDSecRwLtStHdrstFrwdBkwdPosMax_Below160_Val/1 -> Terminator_252/1
  PA_KeSMSw4sVIPMDSecRwLtStHdrstFrwdBkwdPosMax_Over180_Val/1 -> Terminator_253/1
  PA_KeSMSw4sVIPMDSecRwLtStHdrstFrwdBkwdPosMin_160_Val/1 -> Terminator_254/1
  PA_KeSMSw4sVIPMDSecRwLtStHdrstFrwdBkwdPosMin_165_Val/1 -> Terminator_255/1
  PA_KeSMSw4sVIPMDSecRwLtStHdrstFrwdBkwdPosMin_170_Val/1 -> Terminator_256/1
  PA_KeSMSw4sVIPMDSecRwLtStHdrstFrwdBkwdPosMin_175_Val/1 -> Terminator_257/1
  PA_KeSMSw4sVIPMDSecRwLtStHdrstFrwdBkwdPosMin_180_Val/1 -> Terminator_258/1
  PA_KeSMSw4sVIPMDSecRwLtStHdrstFrwdBkwdPosMin_Below160_Val/1 -> Terminator_259/1
  PA_KeSMSw4sVIPMDSecRwLtStHdrstFrwdBkwdPosMin_Over180_Val/1 -> Terminator_260/1
  PA_KeSMSw4sVIPMDSecRwLtStHdrstFrwdBkwdPos_160_Val/1 -> Terminator_261/1
  PA_KeSMSw4sVIPMDSecRwLtStHdrstFrwdBkwdPos_165_Val/1 -> Terminator_262/1
  PA_KeSMSw4sVIPMDSecRwLtStHdrstFrwdBkwdPos_170_Val/1 -> Terminator_263/1
  PA_KeSMSw4sVIPMDSecRwLtStHdrstFrwdBkwdPos_175_Val/1 -> Terminator_264/1
  PA_KeSMSw4sVIPMDSecRwLtStHdrstFrwdBkwdPos_180_Val/1 -> Terminator_265/1
  PA_KeSMSw4sVIPMDSecRwLtStHdrstFrwdBkwdPos_Below160_Val/1 -> Terminator_266/1
  PA_KeSMSw4sVIPMDSecRwLtStHdrstFrwdBkwdPos_Over180_Val/1 -> Terminator_267/1
  PA_KeSMSw4sVIPMDSecRwLtStHdrstUpwdDnwdPosMax_160_Val/1 -> Terminator_268/1
  PA_KeSMSw4sVIPMDSecRwLtStHdrstUpwdDnwdPosMax_165_Val/1 -> Terminator_269/1
  PA_KeSMSw4sVIPMDSecRwLtStHdrstUpwdDnwdPosMax_170_Val/1 -> Terminator_270/1
  PA_KeSMSw4sVIPMDSecRwLtStHdrstUpwdDnwdPosMax_175_Val/1 -> Terminator_271/1
  PA_KeSMSw4sVIPMDSecRwLtStHdrstUpwdDnwdPosMax_180_Val/1 -> Terminator_272/1
  PA_KeSMSw4sVIPMDSecRwLtStHdrstUpwdDnwdPosMax_Below160_Val/1 -> Terminator_273/1
  PA_KeSMSw4sVIPMDSecRwLtStHdrstUpwdDnwdPosMax_Over180_Val/1 -> Terminator_274/1
  PA_KeSMSw4sVIPMDSecRwLtStHdrstUpwdDnwdPosMin_160_Val/1 -> Terminator_275/1
  PA_KeSMSw4sVIPMDSecRwLtStHdrstUpwdDnwdPosMin_165_Val/1 -> Terminator_276/1
  PA_KeSMSw4sVIPMDSecRwLtStHdrstUpwdDnwdPosMin_170_Val/1 -> Terminator_277/1
  PA_KeSMSw4sVIPMDSecRwLtStHdrstUpwdDnwdPosMin_175_Val/1 -> Terminator_278/1
  PA_KeSMSw4sVIPMDSecRwLtStHdrstUpwdDnwdPosMin_180_Val/1 -> Terminator_279/1
  PA_KeSMSw4sVIPMDSecRwLtStHdrstUpwdDnwdPosMin_Below160_Val/1 -> Terminator_280/1
  PA_KeSMSw4sVIPMDSecRwLtStHdrstUpwdDnwdPosMin_Over180_Val/1 -> Terminator_281/1
  PA_KeSMSw4sVIPMDSecRwLtStHdrstUpwdDnwdPos_160_Val/1 -> Terminator_282/1
  PA_KeSMSw4sVIPMDSecRwLtStHdrstUpwdDnwdPos_165_Val/1 -> Terminator_283/1
  PA_KeSMSw4sVIPMDSecRwLtStHdrstUpwdDnwdPos_170_Val/1 -> Terminator_284/1
  PA_KeSMSw4sVIPMDSecRwLtStHdrstUpwdDnwdPos_175_Val/1 -> Terminator_285/1
  PA_KeSMSw4sVIPMDSecRwLtStHdrstUpwdDnwdPos_180_Val/1 -> Terminator_286/1
  PA_KeSMSw4sVIPMDSecRwLtStHdrstUpwdDnwdPos_Below160_Val/1 -> Terminator_287/1
  PA_KeSMSw4sVIPMDSecRwLtStHdrstUpwdDnwdPos_Over180_Val/1 -> Terminator_288/1
  PA_KeSMSw4sVIPMDSecRwLtStLgrstOtwdInwdPosMax_160_Val/1 -> Terminator_289/1
  PA_KeSMSw4sVIPMDSecRwLtStLgrstOtwdInwdPosMax_165_Val/1 -> Terminator_290/1
  PA_KeSMSw4sVIPMDSecRwLtStLgrstOtwdInwdPosMax_170_Val/1 -> Terminator_291/1
  PA_KeSMSw4sVIPMDSecRwLtStLgrstOtwdInwdPosMax_175_Val/1 -> Terminator_292/1
  PA_KeSMSw4sVIPMDSecRwLtStLgrstOtwdInwdPosMax_180_Val/1 -> Terminator_293/1
  PA_KeSMSw4sVIPMDSecRwLtStLgrstOtwdInwdPosMax_Below160_Val/1 -> Terminator_294/1
  PA_KeSMSw4sVIPMDSecRwLtStLgrstOtwdInwdPosMax_Over180_Val/1 -> Terminator_295/1
  PA_KeSMSw4sVIPMDSecRwLtStLgrstOtwdInwdPosMin_160_Val/1 -> Terminator_296/1
  PA_KeSMSw4sVIPMDSecRwLtStLgrstOtwdInwdPosMin_165_Val/1 -> Terminator_297/1
  PA_KeSMSw4sVIPMDSecRwLtStLgrstOtwdInwdPosMin_170_Val/1 -> Terminator_298/1
  PA_KeSMSw4sVIPMDSecRwLtStLgrstOtwdInwdPosMin_175_Val/1 -> Terminator_299/1
  PA_KeSMSw4sVIPMDSecRwLtStLgrstOtwdInwdPosMin_180_Val/1 -> Terminator_300/1
  PA_KeSMSw4sVIPMDSecRwLtStLgrstOtwdInwdPosMin_Below160_Val/1 -> Terminator_301/1
  PA_KeSMSw4sVIPMDSecRwLtStLgrstOtwdInwdPosMin_Over180_Val/1 -> Terminator_302/1
  PA_KeSMSw4sVIPMDSecRwLtStLgrstOtwdInwdPos_160_Val/1 -> Terminator_303/1
  PA_KeSMSw4sVIPMDSecRwLtStLgrstOtwdInwdPos_165_Val/1 -> Terminator_304/1
  PA_KeSMSw4sVIPMDSecRwLtStLgrstOtwdInwdPos_170_Val/1 -> Terminator_305/1
  PA_KeSMSw4sVIPMDSecRwLtStLgrstOtwdInwdPos_175_Val/1 -> Terminator_306/1
  PA_KeSMSw4sVIPMDSecRwLtStLgrstOtwdInwdPos_180_Val/1 -> Terminator_307/1
  PA_KeSMSw4sVIPMDSecRwLtStLgrstOtwdInwdPos_Below160_Val/1 -> Terminator_308/1
  PA_KeSMSw4sVIPMDSecRwLtStLgrstOtwdInwdPos_Over180_Val/1 -> Terminator_309/1
  PA_KeSMSw4sVIPMDSecRwLtStLgrstUpwdDnwdPosMax_Val/1 -> Terminator_310/1
  PA_KeSMSw4sVIPMDSecRwLtStLgrstUpwdDnwdPosMin_Val/1 -> Terminator_311/1
  PA_KeSMSw4sVIPMDSecRwLtStLgrstUpwdDnwdPos_Val/1 -> Terminator_312/1
  PA_KeSMSw6SAcsMd56SecRwLtStBkReclnUpwdDnwdPos1Max_Val/1 -> Terminator_313/1
  PA_KeSMSw6SAcsMd56SecRwLtStBkReclnUpwdDnwdPos1Min_Val/1 -> Terminator_314/1
  PA_KeSMSw6SAcsMd56SecRwLtStBkReclnUpwdDnwdPos1_Val/1 -> Terminator_315/1
  PA_KeSMSw6SAcsMd56SecRwLtStBkReclnUpwdDnwdPosMax_Val/1 -> Terminator_316/1
  PA_KeSMSw6SAcsMd56SecRwLtStBkReclnUpwdDnwdPosMin_Val/1 -> Terminator_317/1
  PA_KeSMSw6SAcsMd56SecRwLtStBkReclnUpwdDnwdPos_Val/1 -> Terminator_318/1
  PA_KeSMSw6SAcsMd56SecRwLtStFrwdBkwdPosMax_Val/1 -> Terminator_319/1
  PA_KeSMSw6SAcsMd56SecRwLtStFrwdBkwdPosMin_Val/1 -> Terminator_320/1
  PA_KeSMSw6SAcsMd56SecRwLtStFrwdBkwdPos_Val/1 -> Terminator_321/1
  PA_KeSMSw6SAcsMd56SecRwLtStLgrstInwdOtwdPosMax_Val/1 -> Terminator_322/1
  PA_KeSMSw6SAcsMd56SecRwLtStLgrstInwdOtwdPosMin_Val/1 -> Terminator_323/1
  PA_KeSMSw6SAcsMd56SecRwLtStLgrstInwdOtwdPos_Val/1 -> Terminator_324/1
  PA_KeSMSw6SAcsMd56SecRwLtStLgrstUpwdPosMax_Val/1 -> Terminator_325/1
  PA_KeSMSw6SAcsMd56SecRwLtStLgrstUpwdPosMin_Val/1 -> Terminator_326/1
  PA_KeSMSw6SAcsMd56SecRwLtStLgrstUpwdPos_Val/1 -> Terminator_327/1
  PA_KeSMSw6SVIPMdSecRwLtStLgrstInwdOtwdPosMax_Val/1 -> Terminator_328/1
  PA_KeSMSw6SVIPMdSecRwLtStLgrstInwdOtwdPosMin_Val/1 -> Terminator_329/1
  PA_KeSMSw6SVIPMdSecRwLtStLgrstInwdOtwdPos_Val/1 -> Terminator_330/1
  PA_KeSMSw6sAcsEntrySecRwLtStArmScrnPosMax_Val/1 -> Terminator_331/1
  PA_KeSMSw6sAcsEntrySecRwLtStArmScrnPosMin_Val/1 -> Terminator_332/1
  PA_KeSMSw6sAcsEntrySecRwLtStArmScrnPos_Val/1 -> Terminator_333/1
  PA_KeSMSw6sAcsEntrySecRwLtStBkReclnUpwdDnwd1Pos_Val/1 -> Terminator_334/1
  PA_KeSMSw6sAcsEntrySecRwLtStBkReclnUpwdDnwdPos1Max_Val/1 -> Terminator_335/1
  PA_KeSMSw6sAcsEntrySecRwLtStBkReclnUpwdDnwdPos1Min_Val/1 -> Terminator_336/1
  PA_KeSMSw6sAcsEntrySecRwLtStBkReclnUpwdDnwdPosMax_Val/1 -> Terminator_337/1
  PA_KeSMSw6sAcsEntrySecRwLtStBkReclnUpwdDnwdPosMin_Val/1 -> Terminator_338/1
  PA_KeSMSw6sAcsEntrySecRwLtStBkReclnUpwdDnwdPos_Val/1 -> Terminator_339/1
  PA_KeSMSw6sAcsEntrySecRwLtStFrwdBkwdPosMax_Val/1 -> Terminator_340/1
  PA_KeSMSw6sAcsEntrySecRwLtStFrwdBkwdPosMin_Val/1 -> Terminator_341/1
  PA_KeSMSw6sAcsEntrySecRwLtStFrwdBkwdPos_Val/1 -> Terminator_342/1
  PA_KeSMSw6sAcsEntrySecRwLtStLgrstInwdOtwdPosMax_Val/1 -> Terminator_343/1
  PA_KeSMSw6sAcsEntrySecRwLtStLgrstInwdOtwdPosMin_Val/1 -> Terminator_344/1
  PA_KeSMSw6sAcsEntrySecRwLtStLgrstInwdOtwdPos_Val/1 -> Terminator_345/1
  PA_KeSMSw6sAcsEntrySecRwLtStLgrstUpwdPosMax_Val/1 -> Terminator_346/1
  PA_KeSMSw6sAcsEntrySecRwLtStLgrstUpwdPosMin_Val/1 -> Terminator_347/1
  PA_KeSMSw6sAcsEntrySecRwLtStLgrstUpwdPos_Val/1 -> Terminator_348/1
  PA_KeSMSw6sAcsEntrySecRwLtStLtwdRtwdPosMax_Val/1 -> Terminator_349/1
  PA_KeSMSw6sAcsEntrySecRwLtStLtwdRtwdPosMin_Val/1 -> Terminator_350/1
  PA_KeSMSw6sAcsEntrySecRwLtStLtwdRtwdPos_Val/1 -> Terminator_351/1
  PA_KeSMSw6sAcsExtSecRwLtStArmScrnPosMax_Val/1 -> Terminator_352/1
  PA_KeSMSw6sAcsExtSecRwLtStArmScrnPosMin_Val/1 -> Terminator_353/1
  PA_KeSMSw6sAcsExtSecRwLtStArmScrnPos_Val/1 -> Terminator_354/1
  PA_KeSMSw6sAcsExtSecRwLtStBkReclnUpwdDnwdPosMax_Val/1 -> Terminator_355/1
  PA_KeSMSw6sAcsExtSecRwLtStBkReclnUpwdDnwdPosMin_Val/1 -> Terminator_356/1
  PA_KeSMSw6sAcsExtSecRwLtStBkReclnUpwdDnwdPos_Val/1 -> Terminator_357/1
  PA_KeSMSw6sAcsExtSecRwLtStFrwdBkwdPosMax_Val/1 -> Terminator_358/1
  PA_KeSMSw6sAcsExtSecRwLtStFrwdBkwdPosMin_Val/1 -> Terminator_359/1
  PA_KeSMSw6sAcsExtSecRwLtStFrwdBkwdPos_Val/1 -> Terminator_360/1
  PA_KeSMSw6sAcsExtSecRwLtStLgrstUpwdDnwdPosMax_Val/1 -> Terminator_361/1
  PA_KeSMSw6sAcsExtSecRwLtStLgrstUpwdDnwdPosMin_Val/1 -> Terminator_362/1
  PA_KeSMSw6sAcsExtSecRwLtStLgrstUpwdDnwdPos_Val/1 -> Terminator_363/1
  PA_KeSMSw6sAcsExtSecRwLtStLtwdRtwdPosMax_Val/1 -> Terminator_364/1
  PA_KeSMSw6sAcsExtSecRwLtStLtwdRtwdPosMin_Val/1 -> Terminator_365/1
  PA_KeSMSw6sAcsExtSecRwLtStLtwdRtwdPos_Val/1 -> Terminator_366/1
  PA_KeSMSw6sFamilyMdSecRwLtStFrwdBkwdPosMax_Val/1 -> Terminator_367/1
  PA_KeSMSw6sFamilyMdSecRwLtStFrwdBkwdPosMin_Val/1 -> Terminator_368/1
  PA_KeSMSw6sFamilyMdSecRwLtStFrwdBkwdPos_Val/1 -> Terminator_369/1
  PA_KeSMSw6sFamilyMdSecRwLtStLtwdRtwdPosMax_Val/1 -> Terminator_370/1
  PA_KeSMSw6sFamilyMdSecRwLtStLtwdRtwdPosMin_Val/1 -> Terminator_371/1
  PA_KeSMSw6sFamilyMdSecRwLtStLtwdRtwdPos_Val/1 -> Terminator_372/1
  PA_KeSMSw6sFamilyRMdSecRwLtStFrwdBkwdPosMax_Val/1 -> Terminator_373/1
  PA_KeSMSw6sFamilyRMdSecRwLtStFrwdBkwdPosMin_Val/1 -> Terminator_374/1
  PA_KeSMSw6sFamilyRMdSecRwLtStFrwdBkwdPos_Val/1 -> Terminator_375/1
  PA_KeSMSw6sFamilyRMdSecRwLtStLtwdRtwdPosMax_Val/1 -> Terminator_376/1
  PA_KeSMSw6sFamilyRMdSecRwLtStLtwdRtwdPosMin_Val/1 -> Terminator_377/1
  PA_KeSMSw6sFamilyRMdSecRwLtStLtwdRtwdPos_Val/1 -> Terminator_378/1
  PA_KeSMSw6sIntimacyMdSecRwLtStLtwdRtwdPosMax_Val/1 -> Terminator_379/1
  PA_KeSMSw6sIntimacyMdSecRwLtStLtwdRtwdPosMin_Val/1 -> Terminator_380/1
  PA_KeSMSw6sIntimacyMdSecRwLtStLtwdRtwdPos_Val/1 -> Terminator_381/1
  PA_KeSMSw6sIntimacyRMdSecRwLtStLtwdRtwdPosMax_Val/1 -> Terminator_382/1
  PA_KeSMSw6sIntimacyRMdSecRwLtStLtwdRtwdPosMin_Val/1 -> Terminator_383/1
  PA_KeSMSw6sIntimacyRMdSecRwLtStLtwdRtwdPos_Val/1 -> Terminator_384/1
  PA_KeSMSw6sRecoveryMdSecRwLtStBkReclnUpwdDnwdPosMax_Val/1 -> Terminator_385/1
  PA_KeSMSw6sRecoveryMdSecRwLtStBkReclnUpwdDnwdPosMin_Val/1 -> Terminator_386/1
  PA_KeSMSw6sRecoveryMdSecRwLtStBkReclnUpwdDnwdPos_Val/1 -> Terminator_387/1
  PA_KeSMSw6sRecoveryMdSecRwLtStLgrstInwdOtwdPosMax_Val/1 -> Terminator_388/1
  PA_KeSMSw6sRecoveryMdSecRwLtStLgrstInwdOtwdPosMin_Val/1 -> Terminator_389/1
  PA_KeSMSw6sRecoveryMdSecRwLtStLgrstInwdOtwdPos_Val/1 -> Terminator_390/1
  PA_KeSMSw6sRecoveryMdSecRwLtStLgrstUpwdDnwdPosMax_Val/1 -> Terminator_391/1
  PA_KeSMSw6sRecoveryMdSecRwLtStLgrstUpwdDnwdPosMin_Val/1 -> Terminator_392/1
  PA_KeSMSw6sRecoveryMdSecRwLtStLgrstUpwdDnwdPos_Val/1 -> Terminator_393/1
  PA_KeSMSw6sVIPSecRwLtStBkReclnUpwdDnwdPosMax_Val/1 -> Terminator_394/1
  PA_KeSMSw6sVIPSecRwLtStBkReclnUpwdDnwdPosMin_Val/1 -> Terminator_395/1
  PA_KeSMSw6sVIPSecRwLtStBkReclnUpwdDnwdPos_Val/1 -> Terminator_396/1
  PA_KeSMSw6sVIPSecRwLtStFrwdBkwdPosMax_Val/1 -> Terminator_397/1
  PA_KeSMSw6sVIPSecRwLtStFrwdBkwdPosMin_Val/1 -> Terminator_398/1
  PA_KeSMSw6sVIPSecRwLtStFrwdBkwdPos_Val/1 -> Terminator_399/1
  PA_KeSMSw6sVIPSecRwLtStLgrstUpwdPosMax_Val/1 -> Terminator_400/1
  PA_KeSMSw6sVIPSecRwLtStLgrstUpwdPosMin_Val/1 -> Terminator_401/1
  PA_KeSMSw6sVIPSecRwLtStLgrstUpwdPos_Val/1 -> Terminator_402/1
  PA_KeSMSw6sVIPSecRwLtStLtwdRtwdPosMax_Val/1 -> Terminator_403/1
  PA_KeSMSw6sVIPSecRwLtStLtwdRtwdPosMin_Val/1 -> Terminator_404/1
  PA_KeSMSw6sVIPSecRwLtStLtwdRtwdPos_Val/1 -> Terminator_405/1
  PA_KeSMSwAcsEntrySecRwLtStArmScrnPosMax_Val/1 -> Terminator_406/1
  PA_KeSMSwAcsEntrySecRwLtStArmScrnPosMin_Val/1 -> Terminator_407/1
  PA_KeSMSwAcsEntrySecRwLtStArmScrnPos_Val/1 -> Terminator_408/1
  PA_KeSMSwAcsEntrySecRwLtStBkReclnUpwdDnwdPos1Max_Val/1 -> Terminator_409/1
  PA_KeSMSwAcsEntrySecRwLtStBkReclnUpwdDnwdPos1Min_Val/1 -> Terminator_410/1
  PA_KeSMSwAcsEntrySecRwLtStBkReclnUpwdDnwdPos1_Val/1 -> Terminator_411/1
  PA_KeSMSwAcsEntrySecRwLtStBkReclnUpwdDnwdPosMax_Val/1 -> Terminator_412/1
  PA_KeSMSwAcsEntrySecRwLtStBkReclnUpwdDnwdPosMin_Val/1 -> Terminator_413/1
  PA_KeSMSwAcsEntrySecRwLtStBkReclnUpwdDnwdPos_Val/1 -> Terminator_414/1
  PA_KeSMSwAcsEntrySecRwLtStFrwdBkwdPosMax_Val/1 -> Terminator_415/1
  PA_KeSMSwAcsEntrySecRwLtStFrwdBkwdPosMin_Val/1 -> Terminator_416/1
  PA_KeSMSwAcsEntrySecRwLtStFrwdBkwdPos_Val/1 -> Terminator_417/1
  PA_KeSMSwAcsEntrySecRwLtStLgrstInwdOtwdPosMax_Val/1 -> Terminator_418/1
  PA_KeSMSwAcsEntrySecRwLtStLgrstInwdOtwdPosMin_Val/1 -> Terminator_419/1
  PA_KeSMSwAcsEntrySecRwLtStLgrstInwdOtwdPos_Val/1 -> Terminator_420/1
  PA_KeSMSwAcsEntrySecRwLtStLgrstUpwdPosMax_Val/1 -> Terminator_421/1
  PA_KeSMSwAcsEntrySecRwLtStLgrstUpwdPosMin_Val/1 -> Terminator_422/1
  PA_KeSMSwAcsEntrySecRwLtStLgrstUpwdPos_Val/1 -> Terminator_423/1
  PA_KeSMSwAcsEntrySecRwLtStLtwdRtwdPosMax_Val/1 -> Terminator_424/1
  PA_KeSMSwAcsEntrySecRwLtStLtwdRtwdPosMin_Val/1 -> Terminator_425/1
  PA_KeSMSwAcsEntrySecRwLtStLtwdRtwdPos_Val/1 -> Terminator_426/1
  PA_KeSMSwAcsExtSecRwLtStArmScrnPosMax_Val/1 -> Terminator_427/1
  PA_KeSMSwAcsExtSecRwLtStArmScrnPosMin_Val/1 -> Terminator_428/1
  PA_KeSMSwAcsExtSecRwLtStArmScrnPos_Val/1 -> Terminator_429/1
  PA_KeSMSwAcsExtSecRwLtStBkReclnUpwdDnwdPosMax_Val/1 -> Terminator_430/1
  PA_KeSMSwAcsExtSecRwLtStBkReclnUpwdDnwdPosMin_Val/1 -> Terminator_431/1
  PA_KeSMSwAcsExtSecRwLtStBkReclnUpwdDnwdPos_Val/1 -> Terminator_432/1
  PA_KeSMSwAcsExtSecRwLtStFrwdBkwdPosMax_Val/1 -> Terminator_433/1
  PA_KeSMSwAcsExtSecRwLtStFrwdBkwdPosMin_Val/1 -> Terminator_434/1
  PA_KeSMSwAcsExtSecRwLtStFrwdBkwdPos_Val/1 -> Terminator_435/1
  PA_KeSMSwAcsExtSecRwLtStLgrstUpwdDnwdPosMax_Val/1 -> Terminator_436/1
  PA_KeSMSwAcsExtSecRwLtStLgrstUpwdDnwdPosMin_Val/1 -> Terminator_437/1
  PA_KeSMSwAcsExtSecRwLtStLgrstUpwdDnwdPos_Val/1 -> Terminator_438/1
  PA_KeSMSwAcsExtSecRwLtStLtwdRtwdPosMax_Val/1 -> Terminator_439/1
  PA_KeSMSwAcsExtSecRwLtStLtwdRtwdPosMin_Val/1 -> Terminator_440/1
  PA_KeSMSwAcsExtSecRwLtStLtwdRtwdPos_Val/1 -> Terminator_441/1
  PA_KeSMSwAcsMd32SecRwLtStBkReclnUpwdDnwdPos1Max_Val/1 -> Terminator_442/1
  PA_KeSMSwAcsMd32SecRwLtStBkReclnUpwdDnwdPos1Min_Val/1 -> Terminator_443/1
  PA_KeSMSwAcsMd32SecRwLtStBkReclnUpwdDnwdPos1_Val/1 -> Terminator_444/1
  PA_KeSMSwAcsMd32SecRwLtStBkReclnUpwdDnwdPosMax_Val/1 -> Terminator_445/1
  PA_KeSMSwAcsMd32SecRwLtStBkReclnUpwdDnwdPosMin_Val/1 -> Terminator_446/1
  PA_KeSMSwAcsMd32SecRwLtStBkReclnUpwdDnwdPos_Val/1 -> Terminator_447/1
  PA_KeSMSwAcsMd56SecRwLtStBkReclnUpwdDnwdPos1Max_Val/1 -> Terminator_448/1
  PA_KeSMSwAcsMd56SecRwLtStBkReclnUpwdDnwdPos1Min_Val/1 -> Terminator_449/1
  PA_KeSMSwAcsMd56SecRwLtStBkReclnUpwdDnwdPos1_Val/1 -> Terminator_450/1
  PA_KeSMSwAcsMd56SecRwLtStBkReclnUpwdDnwdPosMax_Val/1 -> Terminator_451/1
  PA_KeSMSwAcsMd56SecRwLtStBkReclnUpwdDnwdPosMin_Val/1 -> Terminator_452/1
  PA_KeSMSwAcsMd56SecRwLtStBkReclnUpwdDnwdPos_Val/1 -> Terminator_453/1
  PA_KeSMSwAcsMd56SecRwLtStFrwdBkwdPosMax_Val/1 -> Terminator_454/1
  PA_KeSMSwAcsMd56SecRwLtStFrwdBkwdPosMin_Val/1 -> Terminator_455/1
  PA_KeSMSwAcsMd56SecRwLtStFrwdBkwdPos_Val/1 -> Terminator_456/1
  PA_KeSMSwAcsMd56SecRwLtStLgrstInwdOtwdPosMax_Val/1 -> Terminator_457/1
  PA_KeSMSwAcsMd56SecRwLtStLgrstInwdOtwdPosMin_Val/1 -> Terminator_458/1
  PA_KeSMSwAcsMd56SecRwLtStLgrstInwdOtwdPos_Val/1 -> Terminator_459/1
  PA_KeSMSwAcsMd56SecRwLtStLgrstUpwdPosMax_Val/1 -> Terminator_460/1
  PA_KeSMSwAcsMd56SecRwLtStLgrstUpwdPosMin_Val/1 -> Terminator_461/1
  PA_KeSMSwAcsMd56SecRwLtStLgrstUpwdPos_Val/1 -> Terminator_462/1
  PA_KeSMSwAcsMd8SecRwLtStBkReclnUpwdDnwdPosMax_Val/1 -> Terminator_463/1
  PA_KeSMSwAcsMd8SecRwLtStBkReclnUpwdDnwdPosMin_Val/1 -> Terminator_464/1
  PA_KeSMSwAcsMd8SecRwLtStBkReclnUpwdDnwdPos_Val/1 -> Terminator_465/1
  PA_KeSMSwAcsMd8SecRwLtStFrwdBkwdPosMax_Val/1 -> Terminator_466/1
  PA_KeSMSwAcsMd8SecRwLtStFrwdBkwdPosMin_Val/1 -> Terminator_467/1
  PA_KeSMSwAcsMd8SecRwLtStFrwdBkwdPos_Val/1 -> Terminator_468/1
  PA_KeSMSwAcsMd8SecRwLtStLgrstInwdOtwdPosMax_Val/1 -> Terminator_469/1
  PA_KeSMSwAcsMd8SecRwLtStLgrstInwdOtwdPosMin_Val/1 -> Terminator_470/1
  PA_KeSMSwAcsMd8SecRwLtStLgrstInwdOtwdPos_Val/1 -> Terminator_471/1
  PA_KeSMSwAcsMd8SecRwLtStLgrstUpwdDnwdPosMax_Val/1 -> Terminator_472/1
  PA_KeSMSwAcsMd8SecRwLtStLgrstUpwdDnwdPosMin_Val/1 -> Terminator_473/1
  PA_KeSMSwAcsMd8SecRwLtStLgrstUpwdDnwdPos_Val/1 -> Terminator_474/1
  PA_KeSMSwFamilyMdSecRwLtStFrwdBkwdPosMax_Val/1 -> Terminator_475/1
  PA_KeSMSwFamilyMdSecRwLtStFrwdBkwdPosMin_Val/1 -> Terminator_476/1
  PA_KeSMSwFamilyMdSecRwLtStFrwdBkwdPos_Val/1 -> Terminator_477/1
  PA_KeSMSwFamilyMdSecRwLtStLtwdRtwdPosMax_Val/1 -> Terminator_478/1
  PA_KeSMSwFamilyMdSecRwLtStLtwdRtwdPosMin_Val/1 -> Terminator_479/1
  PA_KeSMSwFamilyMdSecRwLtStLtwdRtwdPos_Val/1 -> Terminator_480/1
  PA_KeSMSwFamilyRMdSecRwLtStFrwdBkwdPosMax_Val/1 -> Terminator_481/1
  PA_KeSMSwFamilyRMdSecRwLtStFrwdBkwdPosMin_Val/1 -> Terminator_482/1
  PA_KeSMSwFamilyRMdSecRwLtStFrwdBkwdPos_Val/1 -> Terminator_483/1
  PA_KeSMSwFamilyRMdSecRwLtStLtwdRtwdPosMax_Val/1 -> Terminator_484/1
  PA_KeSMSwFamilyRMdSecRwLtStLtwdRtwdPosMin_Val/1 -> Terminator_485/1
  PA_KeSMSwFamilyRMdSecRwLtStLtwdRtwdPos_Val/1 -> Terminator_486/1
  PA_KeSMSwIntimacyMdSecRwLtStLtwdRtwdPosMax_Val/1 -> Terminator_487/1
  PA_KeSMSwIntimacyMdSecRwLtStLtwdRtwdPosMin_Val/1 -> Terminator_488/1
  PA_KeSMSwIntimacyMdSecRwLtStLtwdRtwdPos_Val/1 -> Terminator_489/1
  PA_KeSMSwIntimacyRMdSecRwLtStLtwdRtwdPosMax_Val/1 -> Terminator_490/1
  PA_KeSMSwIntimacyRMdSecRwLtStLtwdRtwdPosMin_Val/1 -> Terminator_491/1
  PA_KeSMSwIntimacyRMdSecRwLtStLtwdRtwdPos_Val/1 -> Terminator_492/1
  PA_KeSMSwMd27SecRwLtStBkReclnUpwdDnwdPos1Max_Val/1 -> Terminator_493/1
  PA_KeSMSwMd27SecRwLtStBkReclnUpwdDnwdPos1Min_Val/1 -> Terminator_494/1
  PA_KeSMSwMd27SecRwLtStBkReclnUpwdDnwdPos1_Val/1 -> Terminator_495/1
  PA_KeSMSwMd27SecRwLtStBkReclnUpwdDnwdPos2Max_Val/1 -> Terminator_496/1
  PA_KeSMSwMd27SecRwLtStBkReclnUpwdDnwdPos2Min_Val/1 -> Terminator_497/1
  PA_KeSMSwMd27SecRwLtStBkReclnUpwdDnwdPos2_Val/1 -> Terminator_498/1
  PA_KeSMSwMd27SecRwLtStBkReclnUpwdDnwdPos3Max_Val/1 -> Terminator_499/1
  PA_KeSMSwMd27SecRwLtStBkReclnUpwdDnwdPos3Min_Val/1 -> Terminator_500/1
  PA_KeSMSwMd27SecRwLtStBkReclnUpwdDnwdPos3_Val/1 -> Terminator_501/1
  PA_KeSMSwRecoveryMdSecRwLtStBkReclnUpwdDnwdPosMax_Val/1 -> Terminator_502/1
  PA_KeSMSwRecoveryMdSecRwLtStBkReclnUpwdDnwdPosMin_Val/1 -> Terminator_503/1
  PA_KeSMSwRecoveryMdSecRwLtStBkReclnUpwdDnwdPos_Val/1 -> Terminator_504/1
  PA_KeSMSwRecoveryMdSecRwLtStLgrstInwdOtwdPosMax_Val/1 -> Terminator_505/1
  PA_KeSMSwRecoveryMdSecRwLtStLgrstInwdOtwdPosMin_Val/1 -> Terminator_506/1
  PA_KeSMSwRecoveryMdSecRwLtStLgrstInwdOtwdPos_Val/1 -> Terminator_507/1
  PA_KeSMSwRecoveryMdSecRwLtStLgrstUpwdDnwdPosMax_Val/1 -> Terminator_508/1
  PA_KeSMSwRecoveryMdSecRwLtStLgrstUpwdDnwdPosMin_Val/1 -> Terminator_509/1
  PA_KeSMSwRecoveryMdSecRwLtStLgrstUpwdDnwdPos_Val/1 -> Terminator_510/1
  PA_KeSMSwSecRwLtStBkReclnEnTrigBitMask6s_Val/1 -> Terminator_511/1
  PA_KeSMSwSecRwLtStBkReclnEnTrigBitMask_Val/1 -> Terminator_512/1
  PA_KeSMSwSecRwLtStFwdBkwdEnTrigBitMask6s_Val/1 -> Terminator_513/1
  PA_KeSMSwSecRwLtStFwdBkwdEnTrigBitMask_Val/1 -> Terminator_514/1
  PA_KeSMSwSecRwLtStLgrstInwdOtwdEnTrigBitMask6s_Val/1 -> Terminator_515/1
  PA_KeSMSwSecRwLtStLgrstInwdOtwdEnTrigBitMask_Val/1 -> Terminator_516/1
  PA_KeSMSwSecRwLtStLgrstUpwdDnwdEnTrigBitMask6s_Val/1 -> Terminator_517/1
  PA_KeSMSwSecRwLtStLgrstUpwdDnwdEnTrigBitMask_Val/1 -> Terminator_518/1
  PA_KeSMSwVIPMdSecRwLtStLgrstInwdOtwdPosMax_Val/1 -> Terminator_519/1
  PA_KeSMSwVIPMdSecRwLtStLgrstInwdOtwdPosMin_Val/1 -> Terminator_520/1
  PA_KeSMSwVIPMdSecRwLtStLgrstInwdOtwdPos_Val/1 -> Terminator_521/1
  PA_KeSMSwVIPSecRwLtStBkReclnUpwdDnwdPosMax_Val/1 -> Terminator_522/1
  PA_KeSMSwVIPSecRwLtStBkReclnUpwdDnwdPosMin_Val/1 -> Terminator_523/1
  PA_KeSMSwVIPSecRwLtStBkReclnUpwdDnwdPos_Val/1 -> Terminator_524/1
  PA_KeSMSwVIPSecRwLtStFrwdBkwdPosMax_Val/1 -> Terminator_525/1
  PA_KeSMSwVIPSecRwLtStFrwdBkwdPosMin_Val/1 -> Terminator_526/1
  PA_KeSMSwVIPSecRwLtStFrwdBkwdPos_Val/1 -> Terminator_527/1
  PA_KeSMSwVIPSecRwLtStLgrstUpwdPosMax_Val/1 -> Terminator_528/1
  PA_KeSMSwVIPSecRwLtStLgrstUpwdPosMin_Val/1 -> Terminator_529/1
  PA_KeSMSwVIPSecRwLtStLgrstUpwdPos_Val/1 -> Terminator_530/1
  PA_KeSMSwVIPSecRwLtStLtwdRtwdPosMax_Val/1 -> Terminator_531/1
  PA_KeSMSwVIPSecRwLtStLtwdRtwdPosMin_Val/1 -> Terminator_532/1
  PA_KeSMSwVIPSecRwLtStLtwdRtwdPos_Val/1 -> Terminator_533/1
  PA_KeSMSwAcsMd6SecRwLtStBkReclnUpwdDnwdPos1Max_Val/1 -> Terminator_534/1
  PA_KeSMSwAcsMd6SecRwLtStBkReclnUpwdDnwdPos1Min_Val/1 -> Terminator_535/1
  PA_KeSMSwAcsMd6SecRwLtStBkReclnUpwdDnwdPos1_Val/1 -> Terminator_536/1
  PA_KeSMSwAcsMd6SecRwLtStBkReclnUpwdDnwdPosMax_Val/1 -> Terminator_537/1
  PA_KeSMSwAcsMd6SecRwLtStBkReclnUpwdDnwdPosMin_Val/1 -> Terminator_538/1
  PA_KeSMSwAcsMd6SecRwLtStBkReclnUpwdDnwdPos_Val/1 -> Terminator_539/1
